simulink library "outp"  (R2021b)
settings: Solver=VariableStepAuto  StartTime=0.0  StopTime=10.0  RelTol=1e-3
undefined symbols (not defined in the file or in its folder): ENUM_PMMMODE_CHARGE, ENUM_PMMMODE_IDLE, ENUM_PMMMODE_INITIALIZE, ENUM_PMMMODE_POWERDOWN, ENUM_PMMMODE_SLEEP, FALSE, Left, outp, slcm, TRUE
libraries: FVT_lib x956, hcu_lib x4, simulink x1
(part 2 of 10)

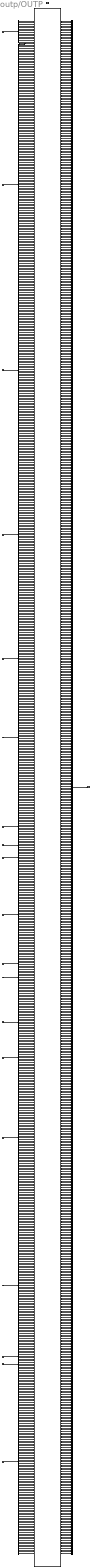
== system outp/OUTP ==
  BACC_outputs : Inport  OutDataTypeStr=Bus: BACC_outputs
  BAPM_outputs : Inport  Port=2  OutDataTypeStr=Bus: BAPM_outputs
  BBCM_outputs : Inport  Port=3  OutDataTypeStr=Bus: BBCM_outputs
  BDDM_outputs : Inport  Port=4  OutDataTypeStr=Bus: BDDM_outputs
  BDHP_outputs : Inport  Port=5  OutDataTypeStr=Bus: BDHP_outputs
  BDID_outputs : Inport  Port=6  OutDataTypeStr=Bus: BDID_outputs
  BDKC_outputs : Inport  Port=7  OutDataTypeStr=Bus: BDKC_outputs
  BDSC_outputs : Inport  Port=8  OutDataTypeStr=Bus: BDSC_outputs
  BNMM_outputs : Inport  Port=9  OutDataTypeStr=Bus: BNMM_outputs
  BPMM_outputs : Inport  Port=10  OutDataTypeStr=Bus: BPMM_outputs
  BPSA_outputs : Inport  Port=11  OutDataTypeStr=Bus: BPSA_outputs
  BSCP_outputs : Inport  Port=12  OutDataTypeStr=Bus: BSCP_outputs
  BSYS_outputs : Inport  Port=13  OutDataTypeStr=Bus: BSYS_outputs
  BTHC_outputs : Inport  Port=14  OutDataTypeStr=Bus: BTHC_outputs
  BTPM_outputs : Inport  Port=15  OutDataTypeStr=Bus: BTPM_outputs
  BTQD_outputs : Inport  Port=16  OutDataTypeStr=Bus: BTQD_outputs
  BTQR_outputs : Inport  Port=17  OutDataTypeStr=Bus: BTQR_outputs
  BV2L_outputs : Inport  Port=18  OutDataTypeStr=Bus: BV2L_outputs
  BVMC_outputs : Inport  Port=19  OutDataTypeStr=Bus: BVMC_outputs
  trig_OUTP : TriggerPort  TriggerType=function-call  VariantControl=(inherit)
  Constant : Constant  Value=FALSE
  bus_creator : BusCreator  Inputs=956  OutDataTypeStr=Bus: BOUTP_outputs  NonVirtualBus=on
  bus_selector1 : BusSelector  OutputSignals=VACC_EACEnDemand_enum,VACC_CACTempOverHigh_flg,VACC_CACPresWarn_flg,VACC_CACPresReady_flg,VACC_EHPSEnDemand_enum,VACC_CACOverrun_flg,VACC_CACRunFail_flg,VACC_EHPSMotorDemSpd_rpm,VACC_EHPSSpdDemTimeout_flg,VACC_EHPSEnTimeout_flg,VACC_EHPSDisEnTimeout_flg,VACC_DCDCEnDemamd_enum,VACC_EHPSSpdCtrlMode_enum,VACC_EACSpdDemand_rpm
  bus_selector10 : BusSelector  OutputSignals=VPMM_SysPowerMode_enum,VPMM_PowerUpState_enum,VPMM_PowerDownState_enum,VPMM_ChrgState_enum,VPMM_PowerUpFault_enum,VPMM_PowerDownFault_enum,VPMM_ChrgFault_enum,VPMM_IRCRlyClose_flg,VPMM_IGNRlyClose_flg,VPMM_BattHVDem_enum,VPMM_DCDCRlyDem_enum,VPMM_CACRlyDem_enum,VPMM_MCUHVLoopDem_enum,VPMM_EHPSRlyDem_enum,VPMM_ACHVLoopDem_enum,VPMM_HVSysReady_enum,VPMM_DrivelineRelease_enum,VPMM_ActiveDischargeReq_enum,VPMM_VCUMCUEn_flg,VPMM_VCUMCUFailRst_flg,VPMM_HVILFail_flg,VPMM_LostHVComActivePwrDown_flg,VPMM_LVBattLowInd_enum,VPMM_ChrgPowerUpFail_flg,VPMM_ChrgBCUHVFail_flg,VPMM_HVFailureChkPass_flg,VPMM_HVILDetectFail_flg,VPMM_V2BLifeSig_cnt,VPMM_V2BAux1OnOff_enum,VPMM_V2BAux2OnOff_enum,VPMM_V2BAux3OnOff_enum,VPMM_V2BMainPosRlySta_enum,VPMM_V2BMainPosRlyFit_enum,VPMM_V2BACPosRlySta_enum,VPMM_V2BACPosRlyFit_enum,VPMM_V2BAirPosRlySta_enum,VPMM_V2BAirPosRlyFit_enum,VPMM_V2BOilPosRlySta_enum,VPMM_V2BOilPosRlyFit_enum,VPMM_V2BDCDCPosRlySta_enum,VPMM_V2BDCDCPosRlyFit_enum,VPMM_V2BAux1RlySta_enum,VPMM_V2BAux1RlyFit_enum,VPMM_V2BAux2RlySta_enum,VPMM_V2BAux2RlyFit_enum,VPMM_V2BAux3RlySta_enum,VPMM_V2BAux3RlyFit_enum,VPMM_V2BAux4RlySta_enum,VPMM_V2BAux4RlyFit_enum,VPMM_VCULife1_cnt,VPMM_VCULife2_cnt,VPMM_VSPFunc_enum,VPMM_VSPIGNKeySta_enum,VPMM_VSPReversed_flg,VPMM_VSPTurnRight_enum,VPMM_VSPTurnLeft_enum,VPMM_FogTMSRlyCMD_enum,VPMM_DCCurr_A,VPMM_DCVol_V
  bus_selector11 : BusSelector  OutputSignals=VPSA_Keystatus_enum,VPSA_EmergencyShutDown_flg
  bus_selector12 : BusSelector  OutputSignals=VSCP_triggerBAM_flg,VSCP_CFGEM1Ctrl_raw,VSCP_CFGEM1BAMTSize_raw,VSCP_CFGEM1BAMTNum_raw,VSCP_CFGEM1BAMRsv_raw,VSCP_CFGEM1BAMPGN_raw,VSCP_triggerDT_flg,VSCP_DTbyte0_raw,VSCP_DTbyte1_raw,VSCP_DTbyte2_raw,VSCP_DTbyte3_raw,VSCP_DTbyte4_raw,VSCP_DTbyte5_raw,VSCP_DTbyte6_raw,VSCP_DTbyte7_raw
  bus_selector13 : BusSelector  OutputSignals=VSYS_HWVer1_cnt,VSYS_HWVer2_cnt,VSYS_HWVer3_cnt,VSYS_CarModel1_cnt,VSYS_CarModel2_cnt,VSYS_CarModel3_cnt,VSYS_ECU1_cnt,VSYS_ECU2_cnt,VSYS_Major1_cnt,VSYS_Major2_cnt,VSYS_Minor1_cnt,VSYS_Minor2_cnt,VSYS_Patch1_cnt,VSYS_Patch2_cnt,VSYS_Country1_cnt,VSYS_Country2_cnt,VSYS_Variation_cnt,VSYS_Dash1_cnt,VSYS_Change1_cnt,VSYS_Change2_cnt,VSYS_Dash2_cnt,VSYS_SHA1_cnt,VSYS_SHA2_cnt,VSYS_SHA3_cnt,VSYS_SHA4_cnt,VSYS_SHA5_cnt,VSYS_SHA6_cnt,VSYS_SHA7_cnt,VSYS_SHA8_cnt,VSYS_NvWriteReqRisingEdge_flg,VSYS_FdcSlpReqRisingEdge_flg,VSYS_FdcSlpTime_sec,VSYS_PmicBootReason_enum,VSYS_WisrBootReason_raw32,VSYS_AcoreRebootCmdACK_flg,VSYS_CurrentNmState_enum,VSYS_ECUGen1_cnt,VSYS_ECUGen2_cnt,VSYS_PmicBootPath_raw32,VSYS_DrivingMode_cnt,VSYS_ModelYear_cnt
  bus_selector14 : BusSelector  OutputSignals=VTHC_EWPPEReq_rpm,VTHC_CoolFanReq_pct,VTHC_AfterrunningMode_flg
  bus_selector15 : BusSelector  OutputSignals=VTPM_LFBatWarn_flg,VTPM_RFBatWarn_flg,VTPM_LRBatWarn_flg,VTPM_RRBatWarn_flg,VTPM_LFWheelPress_raw8,VTPM_RFWheelPress_raw8,VTPM_LRWheelPress_raw8,VTPM_RRWheelPress_raw8,VTPM_LFWheelTemp_C,VTPM_RFWheelTemp_C,VTPM_LRWheelTemp_C,VTPM_RRWheelTemp_C,VTPM_LFSensorFail_flg,VTPM_RFSensorFail_flg,VTPM_LRSensorFail_flg,VTPM_RRSensorFail_flg,VTPM_LFWheelDebug_flg,VTPM_LRWheelDebug_flg,VTPM_RFWheelDebug_flg,VTPM_RRWheelDebug_flg,VTPM_TPMSResButtAllow_flg,VTPM_TPMSCaliButtAllow_flg,VTPM_LFPressIndi_enum,VTPM_RFPressIndi_enum,VTPM_LRPressIndi_enum,VTPM_RRPressIndi_enum,VTPM_TPMSWarnIndi_enum,VTPM_LFWheelTmpIndi_flg,VTPM_RFWheelTmpIndi_flg,VTPM_LRWheelTmpIndi_flg,VTPM_RRWheelTmpIndi_flg,VTPM_LFWheelPSW_raw8,VTPM_LRWheelPSW_raw8,VTPM_RFWheelPSW_raw8,VTPM_RRWheelPSW_raw8,VTPM_CWheelTips_enum,VTPM_AutoLTips_enum,VTPM_LFSensorMode_flg,VTPM_RFSensorMode_flg,VTPM_LRSensorMode_flg,VTPM_RRSensorMode_flg,VTPM_S1ID_raw32,VTPM_S2ID_raw32,VTPM_S3ID_raw32,VTPM_S4ID_raw32,VTPM_S1L_enum,VTPM_S2L_enum,VTPM_S3L_enum,VTPM_S4L_enum,VTPM_ALFin_flg,VTPM_LFP20_raw8,VTPM_RFP20_raw8,VTPM_LRP20_raw8,VTPM_RRP20_raw8,VTPM_FAT_flg,VTPM_IDin_raw32,VTPM_S1WheelDebugALTU_pct,VTPM_S2WheelDebugALTU_pct,VTPM_S3WheelDebugALTU_pct,VTPM_S4WheelDebugALTU_pct,VTPM_ID1messageALTU_raw8,VTPM_ID2messageALTU_raw8,VTPM_ID3messageALTU_raw8,VTPM_ID4messageALTU_raw8,VTPM_Chkfin_flg,VTPM_SetIDLoc_flg,VTPM_TPMSStorge_flg,VTPM_ChkStorge_flg,VTPM_TPMSResButt_flg,VTPM_LFPindi_enum,VTPM_RFPind_enum,VTPM_LRPindi_enum,VTPM_RRPindi_enum,VTPM_WriteChkLFID_raw,VTPM_WriteChkRFID_raw,VTPM_WriteChkLRID_raw,VTPM_WriteChkRRID_raw,VTPM_WriteChkfinLFID_raw,VTPM_WriteChkfinRFID_raw,VTPM_WriteChkfinLRID_raw,VTPM_WriteChkfinRRID_raw,VTPM_Flashchkdatavalid_enum,VTPM_Flashdatavalid_enum,VTPM_unlearnSfali_flg,VTPM_unlearnSfailvalid_enum,VTPM_Prepresstempvalid_enum,VTPM_FlashS1ID_raw,VTPM_FlashS2ID_raw,VTPM_FlashS3ID_raw,VTPM_FlashS4ID_raw,VTPM_FlashIDvalid_enum,VTPM_WritingCnt_enum,VTPM_TPMSTLCmd_flg,VTPM_LProgress_enum,VTPM_TPMSSensorIDRegStart_flg,VTPM_ModelVersion_raw,VTPM_ModelVersionChksum_raw
  bus_selector16 : BusSelector  OutputSignals=VTQD_VCUMCUCtrlMdTQD_enum,VTQD_CreepSpdReq_rpm,VTQD_CreepIND_enum,VTQD_ActTUpAIND_enum,VTQD_VCUMCUDemHiPosVal_rpm,VTQD_VehAcclLimitTG_mps2,VTQD_VCUEBSHHSw_enum,VTQD_VCUEBSRd4BR_enum,VTQD_ParkingProtectWarning_flg,VTQD_ActDriveMode_enum,VTQD_VCU4PweLmtInd_flg,VTQD_GearFlashIndDis_flg,VTQD_GearFlashInd_flg,VTQD_SpdLimSta_flg,VTQD_VehSpdLimitTG_kph,VTQD_VCUTMVehSpd_kph,VTQD_TMTqReq_Nm,VTQD_VCUBCMBuzzReq_flg,VTQD_VCUEBSHBSw_enum,VTQD_EVCU1ActDrvMode_enum,VTQD_EVCU1WheelSlipdet_enum,VTQD_EVCU1EMotorSpd_rpm,VTQD_EVCU1EMotorOvrerSpd_enum,VTQD_EVCU1EMotorPerformance_pct,VTQD_EVCU1EBrakeTorqLow_enum,VTQD_EVCU2MaxTorqAvail_pct,VTQD_EVCU2MinTorqAvail_pct,VTQD_EEC3NFricPercTorq_pct,VTQD_EEC3EMPressLoss_pct,VTQD_ETC2ActDriveDirect_enum,VTQD_RC1PctTrqP4_pct,VTQD_RC1PctTrqPekTrqP5_pct,VTQD_EMRC1EMTquModeDrvBrk_enum,VTQD_EMRC1ActEMpTrq_pct,VTQD_EMRC1ActEMOutSftSpd_rpm,VTQD_EMRC1ActEMpTrqHrls_pct,VTQD_EMRC1ActMaxAvaEMRecpTrq_pct,VTQD_EC1EMSpdIdleP1_rpm,VTQD_EC1PercTorqIdleP1_pct,VTQD_EC1EMSpdIdleP2_rpm,VTQD_EC1PercTorqIdleP2_pct,VTQD_EC1EMSpdIdleP3_rpm,VTQD_EC1PercTorqIdleP3_pct,VTQD_EC1EMSpdIdleP4_rpm,VTQD_EC1PercTorqIdleP4_pct,VTQD_EC1PercTorqIdleP5_pct,VTQD_EC1EMSpdIdleP5_rpm,VTQD_EC1EMRefTorq_Nm,VTQD_EC1EMMaxMEngOvrSP7_rpm,VTQD_EC1EMMaxMOvrTmt_s,VTQD_EC1EMReqSpdCtrlLoLmt_rpm,VTQD_EC1EMReqTrqCtrlLoLmt_pct,VTQD_EC1EMReqSpdCtrlUpLmt_rpm,VTQD_EC1EMReqTrqCtrlUpLmt_pct,VTQD_EC1EMExtRSCtrlUpLmt_rpm,VTQD_EC1EMMomOfInertia_kgpm2,VTQD_EC1EMDefTrqLmt_rpm,VTQD_EC1EMSupVarRTSC1MSG_cnt,VTQD_EC1EMSupTSC1CtrlPG1_cnt,VTQD_EC1EMSupTSC1CtrlPG3_cnt,VTQD_EC1EMSupTSC1CtrlPG2_cnt,VTQD_EC1EMSupTSC1CtrlPG4_cnt,VTQD_EC1EMSpdHdleP6_rpm,VTQD_EC1EMGainEndSpdGvn_gain,VTQD_RC1RetType_enum,VTQD_RC1RetLocat_enum,VTQD_RC1RetCtrlMth_enum,VTQD_RC1RetSpdIdleP1_rpm,VTQD_RC1PctTrqIdleP1_pct,VTQD_RC1MaxRetSpdP2_rpm,VTQD_RC1RetSpdP2_pct,VTQD_RC1MaxRetSpdP3_rpm,VTQD_RC1PctTrqP3_pct,VTQD_RC1RefRetTrq_Nm,VTQD_RC1RetSpdPekTrqP5_Nm,VTQD_RC1RetSpdP4_rpm,VTQD_VCUMCUDemLoNegVal_rpm,VTQD_VCUMCUDemSpd_rpm,VTQD_VCUMCUGearSta_enum,VTQD_TUpAIND_enum,VTQD_ETC1ShiftrPgs_enum,VTQD_EVCU1RecuperHighSta_enum,VTQD_EMRC1DrvDemEMRtapTrq_pct,VTQD_EMRC1RetSelNonEng_pct,VTQD_EMRC1SACtrlDev_cnt,VTQD_VCUMCUHandBrk_flg,VTQD_VCUMCUFootBrk_flg
  bus_selector17 : BusSelector  OutputSignals=VTQR_FrTMTqReq_Nm,VTQR_RrTMTqReq_Nm
  bus_selector18 : BusSelector  OutputSignals=VV2L_ReqOBCV2LEna_enum,VV2L_ReqV2LIVIPopup_enum,VV2L_ReqV2LIVIDisChrg_enum,VV2L_ReqOBCExtrV2LEna_enum,VV2L_ReqOBCIntrV2LEna_enum,VV2L_HVPO120VGrpALDSt_enum,VV2L_HVPO120VGrpBLDSt_enum
  bus_selector19 : BusSelector  OutputSignals=VVMC_FeatSetSpdFinal_raw32,VVMC_VehicleSpeed_mph,VVMC_VehicleSpeed_kph,VVMC_MeterIndSpeed_raw32,VVMC_VMCAEBCtrlAvail_flg,VVMC_VMCACCCtrlAvail_flg,VVMC_VMCCCCtrlAvail_flg,VVMC_VMCMSACtrlAvail_flg,VVMC_FeatArbitrSta_enum,VVMC_FeatReqSpd_kph,VVMC_JerkPCT_pct,VVMC_LimitPCT_pct,VVMC_FrontRearSlipRatioCtrl_flg,VVMC_RearWhlSlipRatioCtrl_flg,VVMC_SingleWhlSlipRatioCtrl_flg,VVMC_LatAccCtrl_flg,VVMC_SafetyCtrl_flg,VVMC_SPD2ACCAct_flg,VVMC_AccCalcuPID_mps2,VVMC_ISOAccLimit_mps2,VVMC_ISODecLimit_mps2,VVMC_ISOJerkLimit_mps3,VVMC_ACCRequiredAccel_mps2,VVMC_DISCReqAcc_mps2,VVMC_FeatArbitrFinal_enum,VVMC_ActACCRequiredAccel_mps2,VVMC_LateralCtrl_flg,VVMC_ADASLKASta_enum,VVMC_LKAStrToqReq_Nm,VVMC_LKATOIFault_flg,VVMC_LKATOIAct_enum,VVMC_ADASAEBReq_enum,VVMC_ADASFaultSta_flg,VVMC_AEBVehHoldReq_flg,VVMC_ACCVehHoldReq_flg,VVMC_ADASDBSReq_enum,VVMC_ADASACCSta_enum,VVMC_ACCObjDist_m,VVMC_ACCObjRelSpd_mps,VVMC_TimeGapLevel_enum,VVMC_ACCJerkUpperLimit_mps3,VVMC_ACCComfortBandUpper_mps2,VVMC_ACCJerkLowerLimit_mps3,VVMC_ACCComfortBandLower_mps2,VVMC_ADASVehSpdLim_raw32,VVMC_ADASShftPosnReqA_flg,VVMC_ADASShftPosnReq_enum,VVMC_ADASForceIdle_flg,VVMC_HazardWarningReq_flg,VVMC_RightTurnLightReq_flg,VVMC_LeftTurnLightReq_flg,VVMC_ADASFCWSta_enum,VVMC_ADASLDWSta_enum,VVMC_ADASFltWrnReq_flg,VVMC_ACCObjDstLvl_enum,VVMC_ForceLowBeam_enum,VVMC_ACCTakeoverReq_flg,VVMC_ADASWarningMsg_enum,VVMC_ADASCAMSpdLim_enum,VVMC_TargetType_enum,VVMC_ADASSLIFSpdLim_enum,VVMC_LKAHODDisplayWarning_flg,VVMC_LKAHODSoundWarning_flg,VVMC_ADASLFCSta_enum,VVMC_ADASLaneModeL_enum,VVMC_ADASLaneModeR_enum,VVMC_ADASSLIFSta_enum,VVMC_ADASISASta_enum,VVMC_ADASLDWMute_flg,VVMC_ADASFCWMute_flg,VVMC_ADASLFCHandsOffWarning_enum,VVMC_LVDADisabled_flg,VVMC_LVDAMuteSta_enum,VVMC_LVDAFailinfo_flg,VVMC_LVDAWarning_flg,VVMC_LVDAACCStatusInformation_flg,VVMC_ADASLFCWarnSound_enum,VVMC_FCMACCmode_enum,VVMC_ADASLanetypeR_enum,VVMC_ADASLanetypeL_enum,VVMC_ADASLanecurveL_raw32,VVMC_ADASLanecurveR_raw32,VVMC_ADASAEBSta_enum,VVMC_FCMLDWRequest_enum,VVMC_FCMLDWFault_flg,VVMC_ACCCtrlAvail_flg,VVMC_ACCPedalOvrd_flg,VVMC_TimeGapCalcu_s,VVMC_CCCtrlSta_enum,VVMC_MSACtrlSta_enum,VVMC_APSCtrlAvail_flg,VVMC_APSActive_flg,VVMC_APSStaSys_enum,VVMC_APSDecReqA_flg,VVMC_APSDecReq_mps2,VVMC_APSReq_enum,VVMC_LongAcc_Gps,VVMC_CCMSASpdWar_flg,VVMC_IMUEnaCmd_flg,VVMC_CAASCtrlAvail_flg,VVMC_CAASActive_flg,VVMC_ExtraMSACtrlSta_enum,VVMC_CalibratedAccX_G,VVMC_CalibratedAccY_G,VVMC_CalibratedAccZ_G,VVMC_CalibratedGyroX_Dps,VVMC_CalibratedGyroY_Dps,VVMC_CalibratedGyroZ_Dps,VVMC_FDCVMCAPSVRqEPSCtrl_flg,VVMC_FDCVMCAPSAngleTarget_deg,VVMC_FDCVMCAPSRqEPSCtrl_flg,VVMC_FDCVMCAngCtrlTqWtGn_pct,VVMC_FDCVMCDrInpTqBstAct_flg,VVMC_FDCVMCMaxAngCtrlOutTqLim_Nm,VVMC_FDCVMCDrInpTqBstGn_pct
  bus_selector2 : BusSelector  OutputSignals=VAPM_VehSpeed_kph,VAPM_VehSpeedTimeOut_flg,VAPM_FSOffSw_enum,VAPM_FSOffSwTimeOut_flg,VAPM_ChrgPlugSta_enum,VAPM_PASDRMR_cm,VAPM_PASDRML_cm,VAPM_PASDRCR_cm,VAPM_PASDRCL_cm,VAPM_PASDFMR_cm,VAPM_PASDFML_cm,VAPM_PASDFCR_cm,VAPM_PASDFCL_cm,VAPM_APSDRLR_cm,VAPM_APSDRLL_cm,VAPM_APSDFLR_cm,VAPM_APSDFLL_cm,VAPM_PASAFCL_enum,VAPM_PASARMR_enum,VAPM_PASARML_enum,VAPM_PASARCR_enum,VAPM_PASARCL_enum,VAPM_PASAFMR_enum,VAPM_PASAFML_enum,VAPM_PASAFCR_enum,VAPM_USSStaRMR_flg,VAPM_USSStaRML_flg,VAPM_USSStaRLR_flg,VAPM_USSStaRLL_flg,VAPM_USSStaRCR_flg,VAPM_USSStaRCL_flg,VAPM_USSStaFMR_flg,VAPM_USSStaFML_flg,VAPM_USSStaFLR_flg,VAPM_USSStaFLL_flg,VAPM_USSStaFCR_flg,VAPM_USSStaFCL_flg,VAPM_Chime_enum,VAPM_SNSRLayout_enum,VAPM_StaFSya_flg,VAPM_ModOperation_enum,VAPM_BrkPedalPos_pct,VAPM_BrkPedalPosTimeOut_flg,VAPM_LFRawWhlSpeed_kph,VAPM_LFRawWhlSpeedTimeOut_flg,VAPM_RFRawWhlSpeed_kph,VAPM_RFRawWhlSpeedTimeOut_flg,VAPM_LRRawWhlSpeed_kph,VAPM_LRRawWhlSpeedTimeOut_flg,VAPM_RRRawWhlSpeed_kph,VAPM_RRRawWhlSpeedTimeOut_flg,VAPM_LFRawWhlSpeedV_flg,VAPM_LFRawWhlSpeedVTimeOut_flg,VAPM_RFRawWhlSpeedV_flg,VAPM_RFRawWhlSpeedVTimeOut_flg,VAPM_LRRawWhlSpeedV_flg,VAPM_LRRawWhlSpeedVTimeOut_flg,VAPM_RRRawWhlSpeedV_flg,VAPM_RRRawWhlSpeedVTimeOut_flg,VAPM_LFWhlRotDir_enum,VAPM_LFWhlRotDirTimeOut_flg,VAPM_RFWhlRotDir_enum,VAPM_RFWhlRotDirTimeOut_flg,VAPM_LRWhlRotDir_enum,VAPM_LRWhlRotDirTimeOut_flg,VAPM_RRWhlRotDir_enum,VAPM_RRWhlRotDirTimeOut_flg,VAPM_LFPulseCountV_flg,VAPM_LFPulseCountVTimeOut_flg,VAPM_RFPulseCountV_flg,VAPM_RFPulseCountVTimeOut_flg,VAPM_LRPulseCountV_flg,VAPM_LRPulseCountVTimeOut_flg,VAPM_RRPulseCountV_flg,VAPM_RRPulseCountVTimeOut_flg,VAPM_LFPulseCount_enum,VAPM_LFPulseCountTimeOut_flg,VAPM_RFPulseCount_enum,VAPM_RFPulseCountTimeOut_flg,VAPM_LRPulseCount_enum,VAPM_LRPulseCountTimeOut_flg,VAPM_RRPulseCount_enum,VAPM_RRPulseCountTimeOut_flg,VAPM_ShifterHandleCmd_enum,VAPM_ShifterHandleCmdTimeOut_flg,VAPM_DriIntend_enum,VAPM_DriIntendTimeOut_flg,VAPM_EPSAOIControl_enum,VAPM_EPSAOIControlTimeOut_flg,VAPM_SASAngle_Deg,VAPM_SASAngleTimeOut_flg,VAPM_SASSpeed_degps,VAPM_SASSpeedTimeOut_flg,VAPM_SASSpeedValid_flg,VAPM_SASSpeedValidTimeOut_flg,VAPM_SASCAL_flg,VAPM_SASCALTimeOut_flg,VAPM_SASV_flg,VAPM_SASVTimeOut_flg,VAPM_GRADE_Deg,VAPM_GRADETimeOut_flg,VAPM_YawRate_degps,VAPM_YawRateTimeOut_flg,VAPM_LatAccel_Gps,VAPM_LatAccelTimeOut_flg,VAPM_LongAccel_Gps,VAPM_LongAccelTimeOut_flg,VAPM_MCPressure_bar,VAPM_MCPressureTimeOut_flg,VAPM_YawRateV_flg,VAPM_YawRateVTimeOut_flg,VAPM_LatAccelV_flg,VAPM_LatAccelVTimeOut_flg,VAPM_LongAccelV_flg,VAPM_LongAccelVTimeOut_flg,VAPM_MCPressureV_bar,VAPM_MCPressureVTimeOut_flg,VAPM_BrkSwSta_flg,VAPM_BrkSwStaTimeOut_flg,VAPM_BrkSwV_flg,VAPM_BrkSwVTimeOut_flg,VAPM_ESCStandstill_flg,VAPM_ESCStandstillTimeOut_flg,VAPM_ESCAPSSta_enum,VAPM_ESCAPSStaTimeOut_flg,VAPM_EPBExtReleaseAvail_flg,VAPM_EPBExtReleaseAvailTimeOut_flg,VAPM_EPBExtApplyAvail_flg,VAPM_EPBExtApplyAvailTimeOut_flg,VAPM_EPBErrSta_enum,VAPM_EPBErrStaTimeOut_flg,VAPM_EPBSta_enum,VAPM_EPBStaTimeOut_flg,VAPM_AVMparkingcancel_enum,VAPM_AVMparkingcancelTimeOut_flg,VAPM_AVMparkingexcute_enum,VAPM_AVMparkingexcuteTimeOut_flg,VAPM_AVMParkingmode_enum,VAPM_AVMParkingmodeTimeOut_flg,VAPM_AVMErrSTA_flg,VAPM_AVMErrSTATimeOut_flg,VAPM_IVIStatus_flg,VAPM_IVIStatusTimeOut_flg,VAPM_CAASSw_enum,VAPM_CAASSwTimeOut_flg,VAPM_IVIScreen_enum,VAPM_IVIScreenTimeOut_flg,VAPM_ABSActive_flg,VAPM_ABSActiveTimeOut_flg,VAPM_TCSActive_flg,VAPM_TCSActiveTimeOut_flg,VAPM_DriverSeatBeltCmd_flg,VAPM_DriverSeatBeltCmdTimeOut_flg,VAPM_APSProgressPCT_pct,VAPM_APSRQDisplay_enum,VAPM_APSSWVer_enum,VAPM_APSHWVer_enum,VAPM_APSExitCondition_enum,VAPM_APSAngleTarget_Deg,VAPM_APSVRqEPASCtrl_flg,VAPM_APSRqEPASCtrl_flg,VAPM_CAASSta_enum,VAPM_DKCPDkeyAreaRAPSSta_enum,VAPM_DKCParkingModeCmd_enum,VAPM_PUIDLowPower_flg,VAPM_CAASVMCReqA_flg,VAPM_APSShiftPosnReq_enum,VAPM_APSSpeedCMD_kph,VAPM_APSVMCReqA_flg,VAPM_RAPSBCMLamp_enum,VAPM_RAPSBCMLockReq_flg,VAPM_APSPwrReq_enum,VAPM_RAPSErrWarnSta_enum,VAPM_RAPSErrLv1_flg,VAPM_IVIUserTakeOverAPSSta_flg
  bus_selector3 : BusSelector  OutputSignals=VBCM_FDCBCMLBeamCmd_flg,VBCM_FDCBCMPLampCmd_flg,VBCM_FDCBCMHBeamCmd_flg,VBCM_FDCBCMSMKLCmd_flg,VBCM_FDCBCMSMKRCmd_flg,VBCM_FDCBCMDVRSignalLCmd_flg,VBCM_FDCBCMDVRSignalRCmd_flg,VBCM_FDCBCMBSDBuzzerCmd_flg,VBCM_FDCBCMSLTLpCmd_flg,VBCM_FDCBCMSRTLpCmd_flg,VBCM_FDCBCMLTurnLpCmd_flg,VBCM_FDCBCMRTurnLpCmd_flg,VBCM_FDCBCMStopINDCmd_flg,VBCM_FDCBCMSTOPBALLCmd_flg,VBCM_FDCBCMInnerCallBellCmd_flg,VBCM_FDCBCMCallBellCmd_flg,VBCM_FDCBCMWiperHCmd_flg,VBCM_FDCBCMWasherCmd_flg,VBCM_FDCBCMWiperLCmd_flg,VBCM_FDCBCMLDRLCmd_flg,VBCM_FDCBCMRDRLCmd_flg,VBCM_FDCBCMRFLampCmd_flg,VBCM_TurnLpPatternSta_enum,VBCM_FDCBCMFDoorSta_flg,VBCM_FDCBCMMDoorSta_flg,VBCM_FDCBCMRDoorSta_flg,VBCM_FDCBCMRoomLpAmbCmd_flg,VBCM_FDCBCMLBSDRCmd_flg,VBCM_FDCBCMLBSDYCmd_flg,VBCM_FDCBCMRBSDRCmd_flg,VBCM_FDCBCMRBSDYCmd_flg,VBCM_FDCBCMEmExitSWSta_flg,VBCM_InnerBuzzerModeSta_enum,VBCM_FDCBCMInnerBuzzerCmd_flg,VBCM_FDCBCMRoomLpAmbSetSta_flg,VBCM_FDCBCMRoomLpSetSta_flg,VBCM_FDCBCMFRoomLpSetSta_pct,VBCM_FDCBCMFRoomLpCmd_pct,VBCM_FDCBCMMRoomLpSetSta_pct,VBCM_FDCBCMMRoomLpCmd_pct,VBCM_FDCBCMRRoomLpSetSta_pct,VBCM_FDCBCMRRoomLpCmd_pct,VBCM_FDCBCMHelpINDCmd_flg,VBCM_FDCBCMOSDrOpenSWSta_enum,VBCM_FDCBCMEmSVCmd_flg,VBCM_FDCBCMFDOpenSVCmd_flg,VBCM_FDCBCMFDCloseSVCmd_flg,VBCM_FDCBCMMDOpenSVCmd_flg,VBCM_FDCBCMMDCloseSVCmd_flg,VBCM_FDCBCMLTurnSWSta_flg,VBCM_FDCBCMRTurnSWSta_flg,VBCM_FDCBCMRGearSta_flg,VBCM_FDCBCMBrakeCmd_flg,VBCM_FDCBCMTurnBuzzerENSta_flg,VBCM_WakeUp_flg,VBCM_KeepWakeUp_flg
  bus_selector4 : BusSelector  OutputSignals=VDDM_C3BMS6RCDTC_raw32,VDDM_C3BMS6CSDTC_raw32,VDDM_C3BMS6LCDTC_raw32,VDDM_C3BMS1RCDTC_raw32,VDDM_C3BMS1CSDTC_raw32,VDDM_C3BMS1LCDTC_raw32,VDDM_C3CCU1RCDTC_raw32,VDDM_C3CCU1CSDTC_raw32,VDDM_C3CCU1LCDTC_raw32,VDDM_C3CCU2RCDTC_raw32,VDDM_C3CCU2CSDTC_raw32,VDDM_C3CCU2LCDTC_raw32,VDDM_C1ABM1RCDTC_raw32,VDDM_C1ABM1CSDTC_raw32,VDDM_C1ABM1LCDTC_raw32,VDDM_Lv1ErrDTC_raw32,VDDM_Lv2ErrDTC_raw32,VDDM_Lv3ErrDTC_raw32,VDDM_Lv4ErrDTC_raw32,VDDM_BrkSWErrDTC_raw32,VDDM_BrkSWNoBacDTC_raw32,VDDM_KeyAuthDTC_raw32,VDDM_ONtoRdyDTC_raw32,VDDM_HVB4PreDTC_raw32,VDDM_MCU4PreDTC_raw32,VDDM_DCDC4PreDTC_raw32,VDDM_HVRlyCloDTC_raw32,VDDM_BMSRdyDTC_raw32,VDDM_DCDCEnaDTC_raw32,VDDM_HiLvSaChkDTC_raw32,VDDM_MidLvSaChkDTC_raw32,VDDM_MCUDisDTC_raw32,VDDM_DCDCDisDTC_raw32,VDDM_HVRlyOpDTC_raw32,VDDM_MCUActDTC_raw32,VDDM_OBC4PreDTC_raw32,VDDM_IniLVLoDTC_raw32,VDDM_LVSupLoDTC_raw32,VDDM_LVSupHiDTC_raw32,VDDM_DrStSWDTC_raw32,VDDM_FLDoorSWDTC_raw32,VDDM_RLDoorSWDTC_raw32,VDDM_FRDoorSWDTC_raw32,VDDM_RRDoorSWDTC_raw32,VDDM_HoodSWDTC_raw32,VDDM_TailgaSWDTC_raw32,VDDM_EDriveSysErrVCUErr_flg,VDDM_VehMalfunLevel_enum,VDDM_APS1SigOoRDTC_raw32,VDDM_APS2SigOoRDTC_raw32,VDDM_APSCorrErrDTC_raw32,VDDM_MCUF1NoComDTC_raw32,VDDM_MCUR1NoComDTC_raw32,VDDM_Shifter1NoComDTC_raw32,VDDM_ESC7NoComDTC_raw32,VDDM_ESC1NoComDTC_raw32,VDDM_ESC5NoComDTC_raw32,VDDM_EnterNewOperCyc_flg,VDDM_DiagHCrashDTC_raw32,VDDM_DiagFLTSDTC_raw32,VDDM_DiagFRTSDTC_raw32,VDDM_DiagRLTSDTC_raw32,VDDM_DiagRRTSDTC_raw32,VDDM_FCLUSSDTC_raw32,VDDM_FMLUSSDTC_raw32,VDDM_FMRUSSDTC_raw32,VDDM_FCRUSSDTC_raw32,VDDM_RCLUSSDTC_raw32,VDDM_RMLUSSDTC_raw32,VDDM_RMRUSSDTC_raw32,VDDM_RCRUSSDTC_raw32,VDDM_FLLUSSDTC_raw32,VDDM_FLRUSSDTC_raw32,VDDM_RLLUSSDTC_raw32,VDDM_RLRUSSDTC_raw32,VDDM_FCM2NoComDTC_raw32,VDDM_FCM2RCErrDTC_raw32,VDDM_FCM2CSErrDTC_raw32,VDDM_FCM3NoComDTC_raw32,VDDM_FCM3RCErrDTC_raw32,VDDM_FCM3CSErrDTC_raw32,VDDM_FCM4NoComDTC_raw32,VDDM_FCM4CSErrDTC_raw32,VDDM_FCM5NoComDTC_raw32,VDDM_FCM5CSErrDTC_raw32,VDDM_ZoneSCPNoComDTC_raw32,VDDM_BMSSigErrDetDTC_raw32,VDDM_FCMACCSigErrDetDTC_raw32,VDDM_FrMCUSigErrDetDTC_raw32,VDDM_RrMCUSigErrDetDTC_raw32,VDDM_CCUSigErrDetDTC_raw32,VDDM_ACCAccelCmdErrDetDTC_raw32,VDDM_ACCMalfuncDetDTC_raw32,VDDM_CCMalfuncDetDTC_raw32,VDDM_MSAMalfuncDetDTC_raw32,VDDM_ISAMalfuncDetDTC_raw32,VDDM_MCUF1RCErrDTC_raw32,VDDM_MCUR1RCErrDTC_raw32,VDDM_MCUF1CSErrDTC_raw32,VDDM_MCUR1CSErrDTC_raw32,VDDM_Shifter1RCErrDTC_raw32,VDDM_Shifter1CSErrDTC_raw32,VDDM_ESC7RCErrDTC_raw32,VDDM_ESC7CSErrDTC_raw32,VDDM_ESC1RCErrDTC_raw32,VDDM_ESC1CSErrDTC_raw32,VDDM_ESC5RCErrDTC_raw32,VDDM_ESC5CSErrDTC_raw32,VDDM_FrMCUTqErrDTC_raw32,VDDM_RrMCUTqErrDTC_raw32,VDDM_LFBatwarnDTC_raw32,VDDM_RFBatwarnDTC_raw32,VDDM_LRBatwarnDTC_raw32,VDDM_RRBatwarnDTC_raw32,VDDM_LFPressIndiDTC_raw32,VDDM_RFPressIndiDTC_raw32,VDDM_LRPressIndiDTC_raw32,VDDM_RRPressIndiDTC_raw32,VDDM_LFWheelTmpHighDTC_raw32,VDDM_RFWheelTmpHighDTC_raw32,VDDM_LRWheelTmpHighDTC_raw32,VDDM_RRWheelTmpHighDTC_raw32,VDDM_LFSensorFailDTC_raw32,VDDM_RFSensorFailDTC_raw32,VDDM_LRSensorFailDTC_raw32,VDDM_RRSensorFailDTC_raw32,VDDM_C1EPAS2LCDTC_raw32,VDDM_5vAPS1PwrErrDTC_raw32,VDDM_5vAPS2PwrErrDTC_raw32,VDDM_EPBLockTODTC_raw32,VDDM_EPBUnlockTODTC_raw32,VDDM_LimpHomeActTmp_flg,VDDM_DTCDetect_enum,VDDM_EngagePFail_flg,VDDM_DisengagePFail_flg,VDDM_VCURAPSErrLv2_flg,VDDM_VCURAPSErrLv3_flg,VDDM_EDriveSysErrShifterErr_flg,VDDM_LVSysErrPwrOutErr_flg,VDDM_HVRlyOpFail_flg,VDDM_MCUActDisFail_flg,VDDM_VCUBrkSWSta_enum,VDDM_VCUFLDoorSta_flg,VDDM_VCUFRDoorSta_flg,VDDM_VCURLDoorSta_flg,VDDM_VCURRDoorSta_flg,VDDM_SysAllowReadySta_flg,VDDM_VCUHoodSWSta_flg,VDDM_VCUTailgateSWSta_flg
  bus_selector5 : BusSelector  OutputSignals=VDHP_ActAPSPosn_pct,VDHP_EAPS1MIN_pct,VDHP_EAPS2MIN_pct,VDHP_ResetPedalZeroPosStart_flg,VDHP_EAPS1NRM_pct,VDHP_EAPS2NRM_pct
  bus_selector6 : BusSelector  OutputSignals=VDID_VSS_kph,VDID_RUNTM_s,VDID_MILDIST_km,VDID_WARMUPS_cnt,VDID_CLRDIST_km,VDID_APPD_pct,VDID_APPE_pct,VDID_MILTIME_min,VDID_CLRTIME_min,VDID_BATSOC_pct,VDID_HEVBATT_V,VDID_ODOMETER_km,VDID_BATSOH_pct,VDID_HVBCellVoltMin_V,VDID_HVBCellVoltMax_V,VDID_HVESSCHARGELIM_kW,VDID_HVESSCHARGEACT_kW,VDID_HVESSENER_Whps,VDID_NUMPSATRIPSFLTMEMCLR_cnt,VDID_HVBattCurr_Ahps,VDID_PSAR_sec,VDID_PSAL_sec,VDID_IPSAR_sec,VDID_IPSAL_sec,VDID_CPSAR_sec,VDID_CPSAL_sec,VDID_HVBNAH_Ahr,VDID_HVBNE_kWh,VDID_IGNCNTR_cnt,VDID_TNBCPSAR_Ahr,VDID_TNBCPSAL_Ahr,VDID_TNECPSAR_kWh,VDID_TNECPSAL_kWh,VDID_TEBPSAR_kWh,VDID_TEBPSAL_kWh,VDID_TGEOVCR_kWh,VDID_TGEOVCL_kWh,VDID_GECHGOVCDCR_kWh,VDID_GECHGOVCDCL_kWh,VDID_GECHGOVCACR_kWh,VDID_GECHGOVCACL_kWh,VDID_RESSV2XENNONPSAR_kWh,VDID_RESSV2XENNONPSAL_kWh,VDID_PKER_kphsqr,VDID_PKEL_kphsqr,VDID_ResetCDEODTR_km,VDID_CDEODTR_km,VDID_CDEODTL_km,VDID_AvgBattTempPSAR_C,VDID_AvgBattTempPSAL_C,VDID_AvgBattTempOVCR_C,VDID_AvgBattTempOVCL_C,VDID_AvgBattTempOFFR_C,VDID_AvgBattTempOFFL_C,VDID_QTYPSATRIPSR_cnt,VDID_QTYPSATRIPSL_cnt,VDID_RESSCNTDODRNGR_cnt,VDID_RESSCNTDODRNGL_cnt,VDID_ETMATOER_kWh,VDID_ETMATOEL_kWh,VDID_ETMBTOER_kWh,VDID_ETMBTOEL_kWh,VDID_RESSTIMESOCPSARNGR_s,VDID_RESSTIMESOCPSARNGL_s,VDID_RESSTIMESOCCHGRNGR_s,VDID_RESSTIMESOCCHGRNGL_s,VDID_RESSTIMESOCOFFRNGR_s,VDID_RESSTIMESOCOFFRNGL_s,VDID_MAXBATTEMPL_C,VDID_MINBATTEMPL_C,VDID_AVGBATTEMPL_C,VDID_PROTOCOLID_enum,VDID_RESSTTEMPRNGAXIS_enum,VDID_RESSTIMESOCRNGAXIS_enum,VDID_RESSCNTSDODRNGAXIS_enum,VDID_CALID_cnt,VDID_ECUNAME_cnt,VDID_PKERNumerator_kphsqr,VDID_PKELNumerator_kphsqr,VDID_BattTempPSAR_sec,VDID_BattTempPSAL_sec,VDID_OVCR_sec,VDID_OVCL_sec,VDID_OFFR_sec,VDID_OFFL_sec,VDID_AVGBATTEMPL_sec,VDID_VinCode_cnt,VDID_STASUP_enum,VDID_HEVMODE_enum,VDID_HVBATT_A,VDID_DIDModelVersion_raw,VDID_DIDModelVersionChksum_raw
  bus_selector7 : BusSelector  OutputSignals=VDKC_DKCTimeSN_cnt,VDKC_DKCAuthSta_enum,VDKC_TimeSNDKCFbk_cnt,VDKC_KeyMissSta_flg,VDKC_KeyModeSta_enum,VDKC_DkeyShowIVISta_enum,VDKC_KeyAreaPS_enum,VDKC_KeyAreaLockUnlock_enum,VDKC_PCommandToBCM_enum,VDKC_DKeyWelcomeSta_enum,VDKC_KeyAreaPTG_enum,VDKC_KeyAreaSPTGSta_enum,VDKC_UIDLowPowerSta_enum,VDKC_DkeyAreaRAPSSta_enum,VDKC_ParkingModeCmd_enum,VDKC_KeyNumSta_enum,VDKC_KeyTypeSta_enum,VDKC_FDCDKCAllowSleep_flg,VDKC_JudgeKeepUnlockZone_flg
  bus_selector8 : BusSelector  OutputSignals=VDSC_DISCTurn_flg,VDSC_DISCTargetSpd_kph,VDSC_DISCSta_enum,VDSC_DISCButtSta_flg
  bus_selector9 : BusSelector  OutputSignals=VNMM_AllCANTxReq_flg,VNMM_NMmTxReq_flg,VNMM_Awake_enum,VNMM_CSB_flg,VNMM_ErrorState_enum,VNMM_NodeID_enum,VNMM_PNI_flg,VNMM_RptMsgReq_flg,VNMM_WakeUp_enum,VNMM_ActiveWU_flg,VNMM_SysNMmSta_enum,VNMM_NetworkReq_flg
  outpmodule : Subsystem
  BOUTP_outputs : Outport  OutDataTypeStr=Bus: BOUTP_outputs
  wires:
  outpmodule/952(VOUTP_FDCVMCAPSRqEPSCtrl_flg) -> bus_creator/952
  outpmodule/950(VOUTP_FDCVMCAPSVRqEPSCtrl_flg) -> bus_creator/950
  outpmodule/948(VOUTP_CalibratedGyroY_Dps) -> bus_creator/948
  outpmodule/947(VOUTP_CalibratedGyroX_Dps) -> bus_creator/947
  outpmodule/942(VOUTP_CAASActive_flg) -> bus_creator/942
  outpmodule/940(VOUTP_IMUEnaCmd_flg) -> bus_creator/940
  outpmodule/938(VOUTP_LongAcc_Gps) -> bus_creator/938
  outpmodule/936(VOUTP_APSDecReq_mps2) -> bus_creator/936
  outpmodule/933(VOUTP_APSActive_flg) -> bus_creator/933
  outpmodule/928(VOUTP_ACCPedalOvrd_flg) -> bus_creator/928
  outpmodule/929(VOUTP_TimeGapCalcu_s) -> bus_creator/929
  outpmodule/925(VOUTP_FCMLDWRequest_enum) -> bus_creator/925
  outpmodule/923(VOUTP_ADASLanecurveR_raw32) -> bus_creator/923
  outpmodule/918(VOUTP_ADASLFCWarnSound_enum) -> bus_creator/918
  outpmodule/914(VOUTP_LVDAMuteSta_enum) -> bus_creator/914
  outpmodule/913(VOUTP_LVDADisabled_flg) -> bus_creator/913
  outpmodule/911(VOUTP_ADASFCWMute_flg) -> bus_creator/911
  outpmodule/910(VOUTP_ADASLDWMute_flg) -> bus_creator/910
  outpmodule/907(VOUTP_ADASLaneModeR_enum) -> bus_creator/907
  outpmodule/908(VOUTP_ADASSLIFSta_enum) -> bus_creator/908
  outpmodule/902(VOUTP_ADASSLIFSpdLim_enum) -> bus_creator/902
  outpmodule/904(VOUTP_LKAHODSoundWarning_flg) -> bus_creator/904
  outpmodule/903(VOUTP_LKAHODDisplayWarning_flg) -> bus_creator/903
  outpmodule/900(VOUTP_ADASCAMSpdLim_enum) -> bus_creator/900
  outpmodule/901(VOUTP_TargetType_enum) -> bus_creator/901
  outpmodule/898(VOUTP_ACCTakeoverReq_flg) -> bus_creator/898
  outpmodule/895(VOUTP_ADASFltWrnReq_flg) -> bus_creator/895
  outpmodule/892(VOUTP_LeftTurnLightReq_flg) -> bus_creator/892
  outpmodule/893(VOUTP_ADASFCWSta_enum) -> bus_creator/893
  outpmodule/890(VOUTP_HazardWarningReq_flg) -> bus_creator/890
  outpmodule/889(VOUTP_ADASForceIdle_flg) -> bus_creator/889
  outpmodule/886(VOUTP_ADASVehSpdLim_raw32) -> bus_creator/886
  outpmodule/883(VOUTP_ACCComfortBandUpper_mps2) -> bus_creator/883
  bus_creator/1 -> BOUTP_outputs/1
  outpmodule/956(VOUTP_FDCVMCDrInpTqBstGn_pct) -> bus_creator/956
  outpmodule/835(VOUTP_ReqOBCV2LEna_enum) -> bus_creator/835
  outpmodule/830(VOUTP_EMRC1SACtrlDev_cnt) -> bus_creator/830
  outpmodule/822(VOUTP_VCUMCUDemLoNegVal_rpm) -> bus_creator/822
  outpmodule/821(VOUTP_RC1RetSpdP4_rpm) -> bus_creator/821
  outpmodule/823(VOUTP_VCUMCUDemSpd_rpm) -> bus_creator/823
  outpmodule/820(VOUTP_RC1RetSpdPekTrqP5_Nm) -> bus_creator/820
  outpmodule/819(VOUTP_RC1RefRetTrq_Nm) -> bus_creator/819
  outpmodule/816(VOUTP_RC1RetSpdP2_pct) -> bus_creator/816
  outpmodule/814(VOUTP_RC1PctTrqIdleP1_pct) -> bus_creator/814
  outpmodule/811(VOUTP_RC1RetLocat_enum) -> bus_creator/811
  outpmodule/808(VOUTP_EC1EMSpdHdleP6_rpm) -> bus_creator/808
  outpmodule/806(VOUTP_EC1EMSupTSC1CtrlPG2_cnt) -> bus_creator/806
  outpmodule/804(VOUTP_EC1EMSupTSC1CtrlPG1_cnt) -> bus_creator/804
  outpmodule/803(VOUTP_EC1EMSupVarRTSC1MSG_cnt) -> bus_creator/803
  outpmodule/799(VOUTP_EC1EMReqTrqCtrlUpLmt_pct) -> bus_creator/799
  outpmodule/794(VOUTP_EC1EMMaxMEngOvrSP7_rpm) -> bus_creator/794
  outpmodule/795(VOUTP_EC1EMMaxMOvrTmt_s) -> bus_creator/795
  outpmodule/789(VOUTP_EC1EMSpdIdleP4_rpm) -> bus_creator/789
  outpmodule/790(VOUTP_EC1PercTorqIdleP4_pct) -> bus_creator/790
  outpmodule/780(VOUTP_EMRC1ActEMOutSftSpd_rpm) -> bus_creator/780
  outpmodule/781(VOUTP_EMRC1ActEMpTrqHrls_pct) -> bus_creator/781
  outpmodule/775(VOUTP_ETC2ActDriveDirect_enum) -> bus_creator/775
  outpmodule/772(VOUTP_EVCU2MinTorqAvail_pct) -> bus_creator/772
  outpmodule/769(VOUTP_EVCU1EMotorPerformance_pct) -> bus_creator/769
  outpmodule/765(VOUTP_EVCU1ActDrvMode_enum) -> bus_creator/765
  outpmodule/843(VOUTP_VehicleSpeed_mph) -> bus_creator/843
  outpmodule/840(VOUTP_HVPO120VGrpALDSt_enum) -> bus_creator/840
  outpmodule/842(VOUTP_FeatSetSpdFinal_raw32) -> bus_creator/842
  outpmodule/838(VOUTP_ReqOBCExtrV2LEna_enum) -> bus_creator/838
  outpmodule/837(VOUTP_ReqV2LIVIDisChrg_enum) -> bus_creator/837
  outpmodule/757(VOUTP_GearFlashIndDis_flg) -> bus_creator/757
  outpmodule/756(VOUTP_VCU4PweLmtInd_flg) -> bus_creator/756
  outpmodule/754(VOUTP_ParkingProtectWarning_flg) -> bus_creator/754
  outpmodule/749(VOUTP_ActTUpAIND_enum) -> bus_creator/749
  outpmodule/747(VOUTP_CreepSpdReq_rpm) -> bus_creator/747
  outpmodule/745(VOUTP_ModelVersionChksum_raw) -> bus_creator/745
  outpmodule/744(VOUTP_ModelVersion_raw) -> bus_creator/744
  outpmodule/741(VOUTP_TPMSTLCmd_flg) -> bus_creator/741
  outpmodule/739(VOUTP_FlashIDvalid_enum) -> bus_creator/739
  outpmodule/736(VOUTP_FlashS2ID_raw) -> bus_creator/736
  outpmodule/734(VOUTP_Prepresstempvalid_enum) -> bus_creator/734
  outpmodule/733(VOUTP_unlearnSfailvalid_enum) -> bus_creator/733
  outpmodule/731(VOUTP_Flashdatavalid_enum) -> bus_creator/731
  outpmodule/727(VOUTP_WriteChkfinRFID_raw) -> bus_creator/727
  outpmodule/728(VOUTP_WriteChkfinLRID_raw) -> bus_creator/728
  outpmodule/726(VOUTP_WriteChkfinLFID_raw) -> bus_creator/726
  outpmodule/724(VOUTP_WriteChkLRID_raw) -> bus_creator/724
  outpmodule/922(VOUTP_ADASLanecurveL_raw32) -> bus_creator/922
  outpmodule/722(VOUTP_WriteChkLFID_raw) -> bus_creator/722
  outpmodule/721(VOUTP_RRPindi_enum) -> bus_creator/721
  outpmodule/720(VOUTP_LRPindi_enum) -> bus_creator/720
  outpmodule/716(VOUTP_ChkStorge_flg) -> bus_creator/716
  outpmodule/713(VOUTP_Chkfin_flg) -> bus_creator/713
  outpmodule/714(VOUTP_SetIDLoc_flg) -> bus_creator/714
  outpmodule/712(VOUTP_ID4messageALTU_raw8) -> bus_creator/712
  outpmodule/709(VOUTP_ID1messageALTU_raw8) -> bus_creator/709
  outpmodule/708(VOUTP_S4WheelDebugALTU_pct) -> bus_creator/708
  outpmodule/706(VOUTP_S2WheelDebugALTU_pct) -> bus_creator/706
  outpmodule/707(VOUTP_S3WheelDebugALTU_pct) -> bus_creator/707
  outpmodule/703(VOUTP_FAT_flg) -> bus_creator/703
  outpmodule/695(VOUTP_S2L_enum) -> bus_creator/695
  outpmodule/693(VOUTP_S4ID_raw32) -> bus_creator/693
  outpmodule/694(VOUTP_S1L_enum) -> bus_creator/694
  outpmodule/691(VOUTP_S2ID_raw32) -> bus_creator/691
  outpmodule/687(VOUTP_RFSensorMode_flg) -> bus_creator/687
  outpmodule/685(VOUTP_AutoLTips_enum) -> bus_creator/685
  outpmodule/682(VOUTP_RFWheelPSW_raw8) -> bus_creator/682
  outpmodule/759(VOUTP_SpdLimSta_flg) -> bus_creator/759
  outpmodule/760(VOUTP_VehSpdLimitTG_kph) -> bus_creator/760
  outpmodule/761(VOUTP_VCUTMVehSpd_kph) -> bus_creator/761
  outpmodule/679(VOUTP_RRWheelTmpIndi_flg) -> bus_creator/679
  outpmodule/681(VOUTP_LRWheelPSW_raw8) -> bus_creator/681
  outpmodule/680(VOUTP_LFWheelPSW_raw8) -> bus_creator/680
  outpmodule/671(VOUTP_LFPressIndi_enum) -> bus_creator/671
  outpmodule/954(VOUTP_FDCVMCDrInpTqBstAct_flg) -> bus_creator/954
  outpmodule/669(VOUTP_TPMSResButtAllow_flg) -> bus_creator/669
  outpmodule/665(VOUTP_LFWheelDebug_flg) -> bus_creator/665
  outpmodule/666(VOUTP_LRWheelDebug_flg) -> bus_creator/666
  outpmodule/662(VOUTP_RFSensorFail_flg) -> bus_creator/662
  outpmodule/661(VOUTP_LFSensorFail_flg) -> bus_creator/661
  outpmodule/652(VOUTP_RRBatWarn_flg) -> bus_creator/652
  outpmodule/650(VOUTP_RFBatWarn_flg) -> bus_creator/650
  outpmodule/649(VOUTP_LFBatWarn_flg) -> bus_creator/649
  outpmodule/644(VOUTP_DrivingMode_cnt) -> bus_creator/644
  outpmodule/639(VOUTP_AcoreRebootCmdACK_flg) -> bus_creator/639
  outpmodule/641(VOUTP_ECUGen1_cnt) -> bus_creator/641
  outpmodule/640(VOUTP_CurrentNmState_enum) -> bus_creator/640
  outpmodule/637(VOUTP_PmicBootReason_enum) -> bus_creator/637
  outpmodule/636(VOUTP_FdcSlpTime_sec) -> bus_creator/636
  outpmodule/633(VOUTP_SHA8_cnt) -> bus_creator/633
  outpmodule/630(VOUTP_SHA5_cnt) -> bus_creator/630
  outpmodule/629(VOUTP_SHA4_cnt) -> bus_creator/629
  outpmodule/628(VOUTP_SHA3_cnt) -> bus_creator/628
  outpmodule/625(VOUTP_Dash2_cnt) -> bus_creator/625
  outpmodule/624(VOUTP_Change2_cnt) -> bus_creator/624
  outpmodule/618(VOUTP_Patch2_cnt) -> bus_creator/618
  outpmodule/619(VOUTP_Country1_cnt) -> bus_creator/619
  outpmodule/617(VOUTP_Patch1_cnt) -> bus_creator/617
  outpmodule/616(VOUTP_Minor2_cnt) -> bus_creator/616
  outpmodule/608(VOUTP_CarModel1_cnt) -> bus_creator/608
  outpmodule/606(VOUTP_HWVer2_cnt) -> bus_creator/606
  outpmodule/604(VOUTP_DTbyte7_raw) -> bus_creator/604
  outpmodule/603(VOUTP_DTbyte6_raw) -> bus_creator/603
  outpmodule/602(VOUTP_DTbyte5_raw) -> bus_creator/602
  outpmodule/597(VOUTP_DTbyte0_raw) -> bus_creator/597
  outpmodule/596(VOUTP_triggerDT_flg) -> bus_creator/596
  outpmodule/595(VOUTP_CFGEM1BAMPGN_raw) -> bus_creator/595
  outpmodule/590(VOUTP_triggerBAM_flg) -> bus_creator/590
  outpmodule/924(VOUTP_ADASAEBSta_enum) -> bus_creator/924
  outpmodule/591(VOUTP_CFGEM1Ctrl_raw) -> bus_creator/591
  outpmodule/589(VOUTP_EmergencyShutDown_flg) -> bus_creator/589
  outpmodule/588(VOUTP_Keystatus_enum) -> bus_creator/588
  outpmodule/586(VOUTP_DCCurr_A) -> bus_creator/586
  outpmodule/585(VOUTP_FogTMSRlyCMD_enum) -> bus_creator/585
  outpmodule/581(VOUTP_VSPIGNKeySta_enum) -> bus_creator/581
  outpmodule/899(VOUTP_ADASWarningMsg_enum) -> bus_creator/899
  outpmodule/578(VOUTP_VCULife1_cnt) -> bus_creator/578
  outpmodule/573(VOUTP_V2BAux2RlyFit_enum) -> bus_creator/573
  outpmodule/571(VOUTP_V2BAux1RlyFit_enum) -> bus_creator/571
  outpmodule/570(VOUTP_V2BAux1RlySta_enum) -> bus_creator/570
  outpmodule/563(VOUTP_V2BACPosRlyFit_enum) -> bus_creator/563
  outpmodule/927(VOUTP_ACCCtrlAvail_flg) -> bus_creator/927
  outpmodule/564(VOUTP_V2BAirPosRlySta_enum) -> bus_creator/564
  outpmodule/560(VOUTP_V2BMainPosRlySta_enum) -> bus_creator/560
  outpmodule/561(VOUTP_V2BMainPosRlyFit_enum) -> bus_creator/561
  outpmodule/551(VOUTP_LVBattLowInd_enum) -> bus_creator/551
  outpmodule/543(VOUTP_ACHVLoopDem_enum) -> bus_creator/543
  outpmodule/541(VOUTP_MCUHVLoopDem_enum) -> bus_creator/541
  outpmodule/538(VOUTP_BattHVDem_enum) -> bus_creator/538
  outpmodule/540(VOUTP_CACRlyDem_enum) -> bus_creator/540
  outpmodule/536(VOUTP_IRCRlyClose_flg) -> bus_creator/536
  outpmodule/531(VOUTP_PowerDownState_enum) -> bus_creator/531
  outpmodule/526(VOUTP_ActiveWU_flg) -> bus_creator/526
  outpmodule/524(VOUTP_RptMsgReq_flg) -> bus_creator/524
  outpmodule/522(VOUTP_NodeID_enum) -> bus_creator/522
  outpmodule/474(VOUTP_RESSTTEMPRNGAXIS_enum) -> bus_creator/474
  outpmodule/471(VOUTP_MINBATTEMPL_C) -> bus_creator/471
  outpmodule/468(VOUTP_RESSTIMESOCOFFRNGR_s) -> bus_creator/468
  outpmodule/465(VOUTP_RESSTIMESOCPSARNGL_s) -> bus_creator/465
  outpmodule/461(VOUTP_ETMATOEL_kWh) -> bus_creator/461
  outpmodule/462(VOUTP_ETMBTOER_kWh) -> bus_creator/462
  outpmodule/792(VOUTP_EC1EMSpdIdleP5_rpm) -> bus_creator/792
  outpmodule/459(VOUTP_RESSCNTDODRNGL_cnt) -> bus_creator/459
  outpmodule/458(VOUTP_RESSCNTDODRNGR_cnt) -> bus_creator/458
  outpmodule/621(VOUTP_Variation_cnt) -> bus_creator/621
  outpmodule/456(VOUTP_QTYPSATRIPSR_cnt) -> bus_creator/456
  outpmodule/453(VOUTP_AvgBattTempOVCL_C) -> bus_creator/453
  outpmodule/751(VOUTP_VehAcclLimitTG_mps2) -> bus_creator/751
  outpmodule/455(VOUTP_AvgBattTempOFFL_C) -> bus_creator/455
  outpmodule/448(VOUTP_CDEODTR_km) -> bus_creator/448
  outpmodule/798(VOUTP_EC1EMReqSpdCtrlUpLmt_rpm) -> bus_creator/798
  outpmodule/447(VOUTP_ResetCDEODTR_km) -> bus_creator/447
  outpmodule/446(VOUTP_PKEL_kphsqr) -> bus_creator/446
  outpmodule/587(VOUTP_DCVol_V) -> bus_creator/587
  outpmodule/443(VOUTP_RESSV2XENNONPSAR_kWh) -> bus_creator/443
  outpmodule/836(VOUTP_ReqV2LIVIPopup_enum) -> bus_creator/836
  outpmodule/444(VOUTP_RESSV2XENNONPSAL_kWh) -> bus_creator/444
  outpmodule/441(VOUTP_GECHGOVCACR_kWh) -> bus_creator/441
  outpmodule/437(VOUTP_TGEOVCR_kWh) -> bus_creator/437
  outpmodule/937(VOUTP_APSReq_enum) -> bus_creator/937
  outpmodule/436(VOUTP_TEBPSAL_kWh) -> bus_creator/436
  outpmodule/438(VOUTP_TGEOVCL_kWh) -> bus_creator/438
  outpmodule/431(VOUTP_TNBCPSAR_Ahr) -> bus_creator/431
  outpmodule/433(VOUTP_TNECPSAR_kWh) -> bus_creator/433
  outpmodule/430(VOUTP_IGNCNTR_cnt) -> bus_creator/430
  outpmodule/427(VOUTP_CPSAL_sec) -> bus_creator/427
  outpmodule/428(VOUTP_HVBNAH_Ahr) -> bus_creator/428
  outpmodule/424(VOUTP_IPSAR_sec) -> bus_creator/424
  outpmodule/423(VOUTP_PSAL_sec) -> bus_creator/423
  outpmodule/422(VOUTP_PSAR_sec) -> bus_creator/422
  outpmodule/420(VOUTP_NUMPSATRIPSFLTMEMCLR_cnt) -> bus_creator/420
  outpmodule/419(VOUTP_HVESSENER_Whps) -> bus_creator/419
  outpmodule/418(VOUTP_HVESSCHARGEACT_kW) -> bus_creator/418
  outpmodule/416(VOUTP_HVBCellVoltMax_V) -> bus_creator/416
  outpmodule/414(VOUTP_BATSOH_pct) -> bus_creator/414
  outpmodule/413(VOUTP_ODOMETER_km) -> bus_creator/413
  outpmodule/412(VOUTP_HEVBATT_V) -> bus_creator/412
  outpmodule/834(VOUTP_RrTMTqReq_Nm) -> bus_creator/834
  outpmodule/410(VOUTP_CLRTIME_min) -> bus_creator/410
  outpmodule/407(VOUTP_APPD_pct) -> bus_creator/407
  outpmodule/916(VOUTP_LVDAWarning_flg) -> bus_creator/916
  outpmodule/404(VOUTP_MILDIST_km) -> bus_creator/404
  outpmodule/405(VOUTP_WARMUPS_cnt) -> bus_creator/405
  outpmodule/403(VOUTP_RUNTM_s) -> bus_creator/403
  outpmodule/479(VOUTP_PKERNumerator_kphsqr) -> bus_creator/479
  outpmodule/909(VOUTP_ADASISASta_enum) -> bus_creator/909
  outpmodule/475(VOUTP_RESSTIMESOCRNGAXIS_enum) -> bus_creator/475
  outpmodule/776(VOUTP_RC1PctTrqP4_pct) -> bus_creator/776
  outpmodule/515(VOUTP_DISCSta_enum) -> bus_creator/515
  outpmodule/512(VOUTP_JudgeKeepUnlockZone_flg) -> bus_creator/512
  outpmodule/506(VOUTP_UIDLowPowerSta_enum) -> bus_creator/506
  outpmodule/507(VOUTP_DkeyAreaRAPSSta_enum) -> bus_creator/507
  outpmodule/501(VOUTP_KeyAreaLockUnlock_enum) -> bus_creator/501
  outpmodule/500(VOUTP_KeyAreaPS_enum) -> bus_creator/500
  outpmodule/498(VOUTP_KeyModeSta_enum) -> bus_creator/498
  outpmodule/496(VOUTP_TimeSNDKCFbk_cnt) -> bus_creator/496
  outpmodule/488(VOUTP_VinCode_cnt) -> bus_creator/488
  outpmodule/486(VOUTP_OFFL_sec) -> bus_creator/486
  outpmodule/483(VOUTP_OVCR_sec) -> bus_creator/483
  outpmodule/388(VOUTP_VCUBrkSWSta_enum) -> bus_creator/388
  outpmodule/387(VOUTP_MCUActDisFail_flg) -> bus_creator/387
  outpmodule/384(VOUTP_EDriveSysErrShifterErr_flg) -> bus_creator/384
  outpmodule/382(VOUTP_VCURAPSErrLv2_flg) -> bus_creator/382
  outpmodule/379(VOUTP_DTCDetect_enum) -> bus_creator/379
  outpmodule/380(VOUTP_EngagePFail_flg) -> bus_creator/380
  outpmodule/377(VOUTP_EPBUnlockTODTC_raw32) -> bus_creator/377
  outpmodule/376(VOUTP_EPBLockTODTC_raw32) -> bus_creator/376
  outpmodule/375(VOUTP_5vAPS2PwrErrDTC_raw32) -> bus_creator/375
  outpmodule/373(VOUTP_C1EPAS2LCDTC_raw32) -> bus_creator/373
  outpmodule/372(VOUTP_RRSensorFailDTC_raw32) -> bus_creator/372
  outpmodule/743(VOUTP_TPMSSensorIDRegStart_flg) -> bus_creator/743
  outpmodule/374(VOUTP_5vAPS1PwrErrDTC_raw32) -> bus_creator/374
  outpmodule/370(VOUTP_RFSensorFailDTC_raw32) -> bus_creator/370
  outpmodule/548(VOUTP_VCUMCUFailRst_flg) -> bus_creator/548
  outpmodule/369(VOUTP_LFSensorFailDTC_raw32) -> bus_creator/369
  outpmodule/365(VOUTP_LFWheelTmpHighDTC_raw32) -> bus_creator/365
  outpmodule/362(VOUTP_RFPressIndiDTC_raw32) -> bus_creator/362
  outpmodule/364(VOUTP_RRPressIndiDTC_raw32) -> bus_creator/364
  outpmodule/363(VOUTP_LRPressIndiDTC_raw32) -> bus_creator/363
  outpmodule/360(VOUTP_RRBatwarnDTC_raw32) -> bus_creator/360
  outpmodule/356(VOUTP_RrMCUTqErrDTC_raw32) -> bus_creator/356
  outpmodule/355(VOUTP_FrMCUTqErrDTC_raw32) -> bus_creator/355
  outpmodule/626(VOUTP_SHA1_cnt) -> bus_creator/626
  outpmodule/353(VOUTP_ESC5RCErrDTC_raw32) -> bus_creator/353
  outpmodule/351(VOUTP_ESC1RCErrDTC_raw32) -> bus_creator/351
  outpmodule/352(VOUTP_ESC1CSErrDTC_raw32) -> bus_creator/352
  outpmodule/350(VOUTP_ESC7CSErrDTC_raw32) -> bus_creator/350
  outpmodule/348(VOUTP_Shifter1CSErrDTC_raw32) -> bus_creator/348
  outpmodule/347(VOUTP_Shifter1RCErrDTC_raw32) -> bus_creator/347
  outpmodule/345(VOUTP_MCUF1CSErrDTC_raw32) -> bus_creator/345
  outpmodule/346(VOUTP_MCUR1CSErrDTC_raw32) -> bus_creator/346
  outpmodule/344(VOUTP_MCUR1RCErrDTC_raw32) -> bus_creator/344
  outpmodule/343(VOUTP_MCUF1RCErrDTC_raw32) -> bus_creator/343
  outpmodule/341(VOUTP_MSAMalfuncDetDTC_raw32) -> bus_creator/341
  outpmodule/340(VOUTP_CCMalfuncDetDTC_raw32) -> bus_creator/340
  outpmodule/337(VOUTP_CCUSigErrDetDTC_raw32) -> bus_creator/337
  outpmodule/931(VOUTP_MSACtrlSta_enum) -> bus_creator/931
  outpmodule/335(VOUTP_FrMCUSigErrDetDTC_raw32) -> bus_creator/335
  outpmodule/336(VOUTP_RrMCUSigErrDetDTC_raw32) -> bus_creator/336
  outpmodule/333(VOUTP_BMSSigErrDetDTC_raw32) -> bus_creator/333
  outpmodule/371(VOUTP_LRSensorFailDTC_raw32) -> bus_creator/371
  outpmodule/334(VOUTP_FCMACCSigErrDetDTC_raw32) -> bus_creator/334
  outpmodule/331(VOUTP_FCM5CSErrDTC_raw32) -> bus_creator/331
  outpmodule/813(VOUTP_RC1RetSpdIdleP1_rpm) -> bus_creator/813
  outpmodule/329(VOUTP_FCM4CSErrDTC_raw32) -> bus_creator/329
  outpmodule/326(VOUTP_FCM3RCErrDTC_raw32) -> bus_creator/326
  outpmodule/323(VOUTP_FCM2RCErrDTC_raw32) -> bus_creator/323
  outpmodule/325(VOUTP_FCM3NoComDTC_raw32) -> bus_creator/325
  outpmodule/324(VOUTP_FCM2CSErrDTC_raw32) -> bus_creator/324
  outpmodule/322(VOUTP_FCM2NoComDTC_raw32) -> bus_creator/322
  outpmodule/320(VOUTP_RLLUSSDTC_raw32) -> bus_creator/320
  outpmodule/394(VOUTP_VCUHoodSWSta_flg) -> bus_creator/394
  outpmodule/396(VOUTP_ActAPSPosn_pct) -> bus_creator/396
  outpmodule/557(VOUTP_V2BAux1OnOff_enum) -> bus_creator/557
  outpmodule/393(VOUTP_SysAllowReadySta_flg) -> bus_creator/393
  outpmodule/317(VOUTP_RCRUSSDTC_raw32) -> bus_creator/317
  outpmodule/316(VOUTP_RMRUSSDTC_raw32) -> bus_creator/316
  outpmodule/314(VOUTP_RCLUSSDTC_raw32) -> bus_creator/314
  outpmodule/670(VOUTP_TPMSCaliButtAllow_flg) -> bus_creator/670
  outpmodule/313(VOUTP_FCRUSSDTC_raw32) -> bus_creator/313
  outpmodule/311(VOUTP_FMLUSSDTC_raw32) -> bus_creator/311
  outpmodule/309(VOUTP_DiagRRTSDTC_raw32) -> bus_creator/309
  outpmodule/310(VOUTP_FCLUSSDTC_raw32) -> bus_creator/310
  outpmodule/378(VOUTP_LimpHomeActTmp_flg) -> bus_creator/378
  outpmodule/658(VOUTP_RFWheelTemp_C) -> bus_creator/658
  outpmodule/308(VOUTP_DiagRLTSDTC_raw32) -> bus_creator/308
  outpmodule/647(VOUTP_CoolFanReq_pct) -> bus_creator/647
  outpmodule/306(VOUTP_DiagFLTSDTC_raw32) -> bus_creator/306
  outpmodule/304(VOUTP_EnterNewOperCyc_flg) -> bus_creator/304
  outpmodule/723(VOUTP_WriteChkRFID_raw) -> bus_creator/723
  outpmodule/955(VOUTP_FDCVMCMaxAngCtrlOutTqLim_Nm) -> bus_creator/955
  outpmodule/302(VOUTP_ESC1NoComDTC_raw32) -> bus_creator/302
  outpmodule/409(VOUTP_MILTIME_min) -> bus_creator/409
  outpmodule/301(VOUTP_ESC7NoComDTC_raw32) -> bus_creator/301
  outpmodule/300(VOUTP_Shifter1NoComDTC_raw32) -> bus_creator/300
  outpmodule/297(VOUTP_APSCorrErrDTC_raw32) -> bus_creator/297
  outpmodule/296(VOUTP_APS2SigOoRDTC_raw32) -> bus_creator/296
  outpmodule/293(VOUTP_EDriveSysErrVCUErr_flg) -> bus_creator/293
  outpmodule/473(VOUTP_PROTOCOLID_enum) -> bus_creator/473
  outpmodule/294(VOUTP_VehMalfunLevel_enum) -> bus_creator/294
  outpmodule/472(VOUTP_AVGBATTEMPL_C) -> bus_creator/472
  outpmodule/887(VOUTP_ADASShftPosnReqA_flg) -> bus_creator/887
  outpmodule/291(VOUTP_HoodSWDTC_raw32) -> bus_creator/291
  outpmodule/549(VOUTP_HVILFail_flg) -> bus_creator/549
  outpmodule/290(VOUTP_RRDoorSWDTC_raw32) -> bus_creator/290
  outpmodule/289(VOUTP_FRDoorSWDTC_raw32) -> bus_creator/289
  outpmodule/664(VOUTP_RRSensorFail_flg) -> bus_creator/664
  outpmodule/287(VOUTP_FLDoorSWDTC_raw32) -> bus_creator/287
  outpmodule/285(VOUTP_LVSupHiDTC_raw32) -> bus_creator/285
  outpmodule/484(VOUTP_OVCL_sec) -> bus_creator/484
  outpmodule/283(VOUTP_IniLVLoDTC_raw32) -> bus_creator/283
  outpmodule/282(VOUTP_OBC4PreDTC_raw32) -> bus_creator/282
  outpmodule/281(VOUTP_MCUActDTC_raw32) -> bus_creator/281
  outpmodule/951(VOUTP_FDCVMCAPSAngleTarget_deg) -> bus_creator/951
  outpmodule/278(VOUTP_MCUDisDTC_raw32) -> bus_creator/278
  outpmodule/280(VOUTP_HVRlyOpDTC_raw32) -> bus_creator/280
  outpmodule/279(VOUTP_DCDCDisDTC_raw32) -> bus_creator/279
  outpmodule/622(VOUTP_Dash1_cnt) -> bus_creator/622
  outpmodule/276(VOUTP_HiLvSaChkDTC_raw32) -> bus_creator/276
  outpmodule/797(VOUTP_EC1EMReqTrqCtrlLoLmt_pct) -> bus_creator/797
  outpmodule/275(VOUTP_DCDCEnaDTC_raw32) -> bus_creator/275
  outpmodule/274(VOUTP_BMSRdyDTC_raw32) -> bus_creator/274
  outpmodule/429(VOUTP_HVBNE_kWh) -> bus_creator/429
  outpmodule/796(VOUTP_EC1EMReqSpdCtrlLoLmt_rpm) -> bus_creator/796
  outpmodule/271(VOUTP_MCU4PreDTC_raw32) -> bus_creator/271
  outpmodule/273(VOUTP_HVRlyCloDTC_raw32) -> bus_creator/273
  outpmodule/318(VOUTP_FLLUSSDTC_raw32) -> bus_creator/318
  outpmodule/270(VOUTP_HVB4PreDTC_raw32) -> bus_creator/270
  outpmodule/269(VOUTP_ONtoRdyDTC_raw32) -> bus_creator/269
  outpmodule/266(VOUTP_BrkSWErrDTC_raw32) -> bus_creator/266
  outpmodule/265(VOUTP_Lv4ErrDTC_raw32) -> bus_creator/265
  outpmodule/262(VOUTP_Lv1ErrDTC_raw32) -> bus_creator/262
  outpmodule/259(VOUTP_C1ABM1RCDTC_raw32) -> bus_creator/259
  outpmodule/258(VOUTP_C3CCU2LCDTC_raw32) -> bus_creator/258
  outpmodule/601(VOUTP_DTbyte4_raw) -> bus_creator/601
  outpmodule/257(VOUTP_C3CCU2CSDTC_raw32) -> bus_creator/257
  outpmodule/593(VOUTP_CFGEM1BAMTNum_raw) -> bus_creator/593
  outpmodule/253(VOUTP_C3CCU1RCDTC_raw32) -> bus_creator/253
  outpmodule/298(VOUTP_MCUF1NoComDTC_raw32) -> bus_creator/298
  outpmodule/252(VOUTP_C3BMS1LCDTC_raw32) -> bus_creator/252
  outpmodule/755(VOUTP_ActDriveMode_enum) -> bus_creator/755
  outpmodule/251(VOUTP_C3BMS1CSDTC_raw32) -> bus_creator/251
  outpmodule/250(VOUTP_C3BMS1RCDTC_raw32) -> bus_creator/250
  outpmodule/520(VOUTP_CSB_flg) -> bus_creator/520
  outpmodule/245(VOUTP_WakeUp_flg) -> bus_creator/245
  outpmodule/556(VOUTP_V2BLifeSig_cnt) -> bus_creator/556
  outpmodule/244(VOUTP_FDCBCMTurnBuzzerENSta_flg) -> bus_creator/244
  outpmodule/246(VOUTP_KeepWakeUp_flg) -> bus_creator/246
  outpmodule/242(VOUTP_FDCBCMRGearSta_flg) -> bus_creator/242
  outpmodule/511(VOUTP_FDCDKCAllowSleep_flg) -> bus_creator/511
  outpmodule/239(VOUTP_FDCBCMMDCloseSVCmd_flg) -> bus_creator/239
  outpmodule/238(VOUTP_FDCBCMMDOpenSVCmd_flg) -> bus_creator/238
  outpmodule/226(VOUTP_FDCBCMRoomLpSetSta_flg) -> bus_creator/226
  outpmodule/224(VOUTP_FDCBCMInnerBuzzerCmd_flg) -> bus_creator/224
  outpmodule/221(VOUTP_FDCBCMRBSDYCmd_flg) -> bus_creator/221
  outpmodule/218(VOUTP_FDCBCMLBSDRCmd_flg) -> bus_creator/218
  outpmodule/219(VOUTP_FDCBCMLBSDYCmd_flg) -> bus_creator/219
  outpmodule/217(VOUTP_FDCBCMRoomLpAmbCmd_flg) -> bus_creator/217
  outpmodule/215(VOUTP_FDCBCMMDoorSta_flg) -> bus_creator/215
  outpmodule/214(VOUTP_FDCBCMFDoorSta_flg) -> bus_creator/214
  outpmodule/212(VOUTP_FDCBCMRFLampCmd_flg) -> bus_creator/212
  outpmodule/208(VOUTP_FDCBCMWasherCmd_flg) -> bus_creator/208
  outpmodule/328(VOUTP_FCM4NoComDTC_raw32) -> bus_creator/328
  outpmodule/788(VOUTP_EC1PercTorqIdleP3_pct) -> bus_creator/788
  outpmodule/207(VOUTP_FDCBCMWiperHCmd_flg) -> bus_creator/207
  outpmodule/415(VOUTP_HVBCellVoltMin_V) -> bus_creator/415
  outpmodule/204(VOUTP_FDCBCMSTOPBALLCmd_flg) -> bus_creator/204
  outpmodule/440(VOUTP_GECHGOVCDCL_kWh) -> bus_creator/440
  outpmodule/201(VOUTP_FDCBCMLTurnLpCmd_flg) -> bus_creator/201
  outpmodule/467(VOUTP_RESSTIMESOCCHGRNGL_s) -> bus_creator/467
  outpmodule/198(VOUTP_FDCBCMBSDBuzzerCmd_flg) -> bus_creator/198
  outpmodule/411(VOUTP_BATSOC_pct) -> bus_creator/411
  outpmodule/194(VOUTP_FDCBCMSMKLCmd_flg) -> bus_creator/194
  outpmodule/663(VOUTP_LRSensorFail_flg) -> bus_creator/663
  outpmodule/191(VOUTP_FDCBCMLBeamCmd_flg) -> bus_creator/191
  outpmodule/186(VOUTP_RAPSBCMLockReq_flg) -> bus_creator/186
  outpmodule/183(VOUTP_APSSpeedCMD_kph) -> bus_creator/183
  outpmodule/182(VOUTP_APSShiftPosnReq_enum) -> bus_creator/182
  outpmodule/180(VOUTP_PUIDLowPower_flg) -> bus_creator/180
  outpmodule/445(VOUTP_PKER_kphsqr) -> bus_creator/445
  outpmodule/181(VOUTP_CAASVMCReqA_flg) -> bus_creator/181
  outpmodule/175(VOUTP_APSVRqEPASCtrl_flg) -> bus_creator/175
  outpmodule/173(VOUTP_APSExitCondition_enum) -> bus_creator/173
  outpmodule/170(VOUTP_APSRQDisplay_enum) -> bus_creator/170
  outpmodule/168(VOUTP_DriverSeatBeltCmdTimeOut_flg) -> bus_creator/168
  outpmodule/452(VOUTP_AvgBattTempOVCR_C) -> bus_creator/452
  outpmodule/167(VOUTP_DriverSeatBeltCmd_flg) -> bus_creator/167
  outpmodule/164(VOUTP_ABSActiveTimeOut_flg) -> bus_creator/164
  outpmodule/165(VOUTP_TCSActive_flg) -> bus_creator/165
  outpmodule/161(VOUTP_IVIScreen_enum) -> bus_creator/161
  outpmodule/268(VOUTP_KeyAuthDTC_raw32) -> bus_creator/268
  outpmodule/417(VOUTP_HVESSCHARGELIM_kW) -> bus_creator/417
  outpmodule/157(VOUTP_IVIStatus_flg) -> bus_creator/157
  outpmodule/247(VOUTP_C3BMS6RCDTC_raw32) -> bus_creator/247
  outpmodule/700(VOUTP_RFP20_raw8) -> bus_creator/700
  outpmodule/235(VOUTP_FDCBCMEmSVCmd_flg) -> bus_creator/235
  outpmodule/236(VOUTP_FDCBCMFDOpenSVCmd_flg) -> bus_creator/236
  outpmodule/514(VOUTP_DISCTargetSpd_kph) -> bus_creator/514
  outpmodule/231(VOUTP_FDCBCMRRoomLpSetSta_pct) -> bus_creator/231
  outpmodule/229(VOUTP_FDCBCMMRoomLpSetSta_pct) -> bus_creator/229
  outpmodule/154(VOUTP_AVMParkingmodeTimeOut_flg) -> bus_creator/154
  outpmodule/155(VOUTP_AVMErrSTA_flg) -> bus_creator/155
  outpmodule/402(VOUTP_VSS_kph) -> bus_creator/402
  outpmodule/152(VOUTP_AVMparkingexcuteTimeOut_flg) -> bus_creator/152
  outpmodule/383(VOUTP_VCURAPSErrLv3_flg) -> bus_creator/383
  outpmodule/150(VOUTP_AVMparkingcancelTimeOut_flg) -> bus_creator/150
  outpmodule/696(VOUTP_S3L_enum) -> bus_creator/696
  outpmodule/147(VOUTP_EPBSta_enum) -> bus_creator/147
  outpmodule/653(VOUTP_LFWheelPress_raw8) -> bus_creator/653
  outpmodule/145(VOUTP_EPBErrSta_enum) -> bus_creator/145
  outpmodule/521(VOUTP_ErrorState_enum) -> bus_creator/521
  outpmodule/140(VOUTP_ESCAPSStaTimeOut_flg) -> bus_creator/140
  outpmodule/367(VOUTP_LRWheelTmpHighDTC_raw32) -> bus_creator/367
  outpmodule/141(VOUTP_EPBExtReleaseAvail_flg) -> bus_creator/141
  outpmodule/138(VOUTP_ESCStandstillTimeOut_flg) -> bus_creator/138
  outpmodule/136(VOUTP_BrkSwVTimeOut_flg) -> bus_creator/136
  outpmodule/134(VOUTP_BrkSwStaTimeOut_flg) -> bus_creator/134
  outpmodule/135(VOUTP_BrkSwV_flg) -> bus_creator/135
  outpmodule/133(VOUTP_BrkSwSta_flg) -> bus_creator/133
  outpmodule/129(VOUTP_LongAccelV_flg) -> bus_creator/129
  outpmodule/480(VOUTP_PKELNumerator_kphsqr) -> bus_creator/480
  outpmodule/131(VOUTP_MCPressureV_bar) -> bus_creator/131
  outpmodule/399(VOUTP_ResetPedalZeroPosStart_flg) -> bus_creator/399
  outpmodule/655(VOUTP_LRWheelPress_raw8) -> bus_creator/655
  outpmodule/127(VOUTP_LatAccelV_flg) -> bus_creator/127
  outpmodule/124(VOUTP_MCPressureTimeOut_flg) -> bus_creator/124
  outpmodule/125(VOUTP_YawRateV_flg) -> bus_creator/125
  outpmodule/126(VOUTP_YawRateVTimeOut_flg) -> bus_creator/126
  outpmodule/121(VOUTP_LongAccel_Gps) -> bus_creator/121
  outpmodule/457(VOUTP_QTYPSATRIPSL_cnt) -> bus_creator/457
  outpmodule/120(VOUTP_LatAccelTimeOut_flg) -> bus_creator/120
  outpmodule/115(VOUTP_GRADE_Deg) -> bus_creator/115
  outpmodule/112(VOUTP_SASCALTimeOut_flg) -> bus_creator/112
  outpmodule/113(VOUTP_SASV_flg) -> bus_creator/113
  outpmodule/108(VOUTP_SASSpeedTimeOut_flg) -> bus_creator/108
  outpmodule/107(VOUTP_SASSpeed_degps) -> bus_creator/107
  outpmodule/105(VOUTP_SASAngle_Deg) -> bus_creator/105
  outpmodule/104(VOUTP_EPSAOIControlTimeOut_flg) -> bus_creator/104
  outpmodule/103(VOUTP_EPSAOIControl_enum) -> bus_creator/103
  outpmodule/98(VOUTP_RRPulseCountTimeOut_flg) -> bus_creator/98
  outpmodule/97(VOUTP_RRPulseCount_enum) -> bus_creator/97
  outpmodule/95(VOUTP_LRPulseCount_enum) -> bus_creator/95
  outpmodule/92(VOUTP_LFPulseCountTimeOut_flg) -> bus_creator/92
  outpmodule/90(VOUTP_RRPulseCountVTimeOut_flg) -> bus_creator/90
  outpmodule/89(VOUTP_RRPulseCountV_flg) -> bus_creator/89
  outpmodule/509(VOUTP_KeyNumSta_enum) -> bus_creator/509
  outpmodule/86(VOUTP_RFPulseCountVTimeOut_flg) -> bus_creator/86
  outpmodule/83(VOUTP_LFPulseCountV_flg) -> bus_creator/83
  outpmodule/81(VOUTP_RRWhlRotDir_enum) -> bus_creator/81
  outpmodule/77(VOUTP_RFWhlRotDir_enum) -> bus_creator/77
  outpmodule/877(VOUTP_ADASDBSReq_enum) -> bus_creator/877
  outpmodule/879(VOUTP_ACCObjDist_m) -> bus_creator/879
  outpmodule/600(VOUTP_DTbyte3_raw) -> bus_creator/600
  outpmodule/878(VOUTP_ADASACCSta_enum) -> bus_creator/878
  outpmodule/876(VOUTP_ACCVehHoldReq_flg) -> bus_creator/876
  outpmodule/660(VOUTP_RRWheelTemp_C) -> bus_creator/660
  outpmodule/875(VOUTP_AEBVehHoldReq_flg) -> bus_creator/875
  outpmodule/631(VOUTP_SHA6_cnt) -> bus_creator/631
  outpmodule/871(VOUTP_LKATOIFault_flg) -> bus_creator/871
  outpmodule/735(VOUTP_FlashS1ID_raw) -> bus_creator/735
  outpmodule/870(VOUTP_LKAStrToqReq_Nm) -> bus_creator/870
  outpmodule/332(VOUTP_ZoneSCPNoComDTC_raw32) -> bus_creator/332
  outpmodule/390(VOUTP_VCUFRDoorSta_flg) -> bus_creator/390
  outpmodule/869(VOUTP_ADASLKASta_enum) -> bus_creator/869
  outpmodule/80(VOUTP_LRWhlRotDirTimeOut_flg) -> bus_creator/80
  outpmodule/867(VOUTP_ActACCRequiredAccel_mps2) -> bus_creator/867
  outpmodule/863(VOUTP_ISOJerkLimit_mps3) -> bus_creator/863
  outpmodule/537(VOUTP_IGNRlyClose_flg) -> bus_creator/537
  outpmodule/862(VOUTP_ISODecLimit_mps2) -> bus_creator/862
  outpmodule/361(VOUTP_LFPressIndiDTC_raw32) -> bus_creator/361
  outpmodule/858(VOUTP_SafetyCtrl_flg) -> bus_creator/858
  outpmodule/859(VOUTP_SPD2ACCAct_flg) -> bus_creator/859
  outpmodule/857(VOUTP_LatAccCtrl_flg) -> bus_creator/857
  outpmodule/856(VOUTP_SingleWhlSlipRatioCtrl_flg) -> bus_creator/856
  outpmodule/853(VOUTP_LimitPCT_pct) -> bus_creator/853
  outpmodule/854(VOUTP_FrontRearSlipRatioCtrl_flg) -> bus_creator/854
  outpmodule/849(VOUTP_VMCMSACtrlAvail_flg) -> bus_creator/849
  outpmodule/847(VOUTP_VMCACCCtrlAvail_flg) -> bus_creator/847
  outpmodule/110(VOUTP_SASSpeedValidTimeOut_flg) -> bus_creator/110
  outpmodule/846(VOUTP_VMCAEBCtrlAvail_flg) -> bus_creator/846
  outpmodule/848(VOUTP_VMCCCCtrlAvail_flg) -> bus_creator/848
  outpmodule/844(VOUTP_VehicleSpeed_kph) -> bus_creator/844
  outpmodule/523(VOUTP_PNI_flg) -> bus_creator/523
  outpmodule/845(VOUTP_MeterIndSpeed_raw32) -> bus_creator/845
  outpmodule/880(VOUTP_ACCObjRelSpd_mps) -> bus_creator/880
  outpmodule/553(VOUTP_ChrgBCUHVFail_flg) -> bus_creator/553
  outpmodule/882(VOUTP_ACCJerkUpperLimit_mps3) -> bus_creator/882
  outpmodule/93(VOUTP_RFPulseCount_enum) -> bus_creator/93
  outpmodule/27(VOUTP_PASDFCR_cm) -> bus_creator/27
  outpmodule/57(VOUTP_BrkPedalPos_pct) -> bus_creator/57
  outpmodule/55(VOUTP_StaFSya_flg) -> bus_creator/55
  outpmodule/562(VOUTP_V2BACPosRlySta_enum) -> bus_creator/562
  outpmodule/53(VOUTP_Chime_enum) -> bus_creator/53
  outpmodule/54(VOUTP_SNSRLayout_enum) -> bus_creator/54
  outpmodule/888(VOUTP_ADASShftPosnReq_enum) -> bus_creator/888
  outpmodule/52(VOUTP_USSStaFCL_flg) -> bus_creator/52
  outpmodule/51(VOUTP_USSStaFCR_flg) -> bus_creator/51
  outpmodule/49(VOUTP_USSStaFLR_flg) -> bus_creator/49
  outpmodule/48(VOUTP_USSStaFML_flg) -> bus_creator/48
  outpmodule/497(VOUTP_KeyMissSta_flg) -> bus_creator/497
  outpmodule/47(VOUTP_USSStaFMR_flg) -> bus_creator/47
  outpmodule/44(VOUTP_USSStaRLL_flg) -> bus_creator/44
  outpmodule/42(VOUTP_USSStaRML_flg) -> bus_creator/42
  outpmodule/943(VOUTP_ExtraMSACtrlSta_enum) -> bus_creator/943
  outpmodule/43(VOUTP_USSStaRLR_flg) -> bus_creator/43
  outpmodule/40(VOUTP_PASAFCR_enum) -> bus_creator/40
  outpmodule/38(VOUTP_PASAFMR_enum) -> bus_creator/38
  outpmodule/546(VOUTP_ActiveDischargeReq_enum) -> bus_creator/546
  outpmodule/37(VOUTP_PASARCL_enum) -> bus_creator/37
  outpmodule/533(VOUTP_PowerUpFault_enum) -> bus_creator/533
  outpmodule/770(VOUTP_EVCU1EBrakeTorqLow_enum) -> bus_creator/770
  outpmodule/36(VOUTP_PASARCR_enum) -> bus_creator/36
  outpmodule/35(VOUTP_PASARML_enum) -> bus_creator/35
  outpmodule/288(VOUTP_RLDoorSWDTC_raw32) -> bus_creator/288
  outpmodule/510(VOUTP_KeyTypeSta_enum) -> bus_creator/510
  outpmodule/701(VOUTP_LRP20_raw8) -> bus_creator/701
  outpmodule/34(VOUTP_PASARMR_enum) -> bus_creator/34
  outpmodule/30(VOUTP_APSDRLL_cm) -> bus_creator/30
  outpmodule/29(VOUTP_APSDRLR_cm) -> bus_creator/29
  outpmodule/482(VOUTP_BattTempPSAL_sec) -> bus_creator/482
  outpmodule/22(VOUTP_PASDRML_cm) -> bus_creator/22
  outpmodule/19(VOUTP_FSOffSwTimeOut_flg) -> bus_creator/19
  outpmodule/17(VOUTP_VehSpeedTimeOut_flg) -> bus_creator/17
  outpmodule/16(VOUTP_VehSpeed_kph) -> bus_creator/16
  outpmodule/833(VOUTP_FrTMTqReq_Nm) -> bus_creator/833
  outpmodule/9(VOUTP_EHPSMotorDemSpd_rpm) -> bus_creator/9
  outpmodule/6(VOUTP_CACOverrun_flg) -> bus_creator/6
  outpmodule/5(VOUTP_EHPSEnDemand_enum) -> bus_creator/5
  outpmodule/4(VOUTP_CACPresReady_flg) -> bus_creator/4
  outpmodule/2(VOUTP_CACTempOverHigh_flg) -> bus_creator/2
  outpmodule/1(VOUTP_EACEnDemand_enum) -> bus_creator/1
  outpmodule/26(VOUTP_PASDFML_cm) -> bus_creator/26
  outpmodule/264(VOUTP_Lv3ErrDTC_raw32) -> bus_creator/264
  outpmodule/25(VOUTP_PASDFMR_cm) -> bus_creator/25
  outpmodule/24(VOUTP_PASDRCL_cm) -> bus_creator/24
  bus_selector19/3 -> outpmodule/844(VVMC_VehicleSpeed_kph)  "<VVMC_VehicleSpeed_kph>"
  bus_selector19/19 -> outpmodule/860(VVMC_AccCalcuPID_mps2)  "<VVMC_AccCalcuPID_mps2>"
  bus_selector19/16 -> outpmodule/857(VVMC_LatAccCtrl_flg)  "<VVMC_LatAccCtrl_flg>"
  outpmodule/119(VOUTP_LatAccel_Gps) -> bus_creator/119
  bus_selector19/14 -> outpmodule/855(VVMC_RearWhlSlipRatioCtrl_flg)  "<VVMC_RearWhlSlipRatioCtrl_flg>"
  outpmodule/643(VOUTP_PmicBootPath_raw32) -> bus_creator/643
  bus_selector19/13 -> outpmodule/854(VVMC_FrontRearSlipRatioCtrl_flg)  "<VVMC_FrontRearSlipRatioCtrl_flg>"
  bus_selector19/11 -> outpmodule/852(VVMC_JerkPCT_pct)  "<VVMC_JerkPCT_pct>"
  outpmodule/648(VOUTP_AfterrunningMode_flg) -> bus_creator/648
  bus_selector19/7 -> outpmodule/848(VVMC_VMCCCCtrlAvail_flg)  "<VVMC_VMCCCCtrlAvail_flg>"
  outpmodule/579(VOUTP_VCULife2_cnt) -> bus_creator/579
  outpmodule/946(VOUTP_CalibratedAccZ_G) -> bus_creator/946
  bus_selector19/20 -> outpmodule/861(VVMC_ISOAccLimit_mps2)  "<VVMC_ISOAccLimit_mps2>"
  outpmodule/225(VOUTP_FDCBCMRoomLpAmbSetSta_flg) -> bus_creator/225
  bus_selector18/6 -> outpmodule/840(VV2L_HVPO120VGrpALDSt_enum)  "<VV2L_HVPO120VGrpALDSt_enum>"
  bus_selector18/5 -> outpmodule/839(VV2L_ReqOBCIntrV2LEna_enum)  "<VV2L_ReqOBCIntrV2LEna_enum>"
  outpmodule/172(VOUTP_APSHWVer_enum) -> bus_creator/172
  bus_selector18/7 -> outpmodule/841(VV2L_HVPO120VGrpBLDSt_enum)  "<VV2L_HVPO120VGrpBLDSt_enum>"
  outpmodule/905(VOUTP_ADASLFCSta_enum) -> bus_creator/905
  BV2L_outputs/1 -> bus_selector18/1
  outpmodule/142(VOUTP_EPBExtReleaseAvailTimeOut_flg) -> bus_creator/142
  bus_selector18/3 -> outpmodule/837(VV2L_ReqV2LIVIDisChrg_enum)  "<VV2L_ReqV2LIVIDisChrg_enum>"
  bus_selector18/2 -> outpmodule/836(VV2L_ReqV2LIVIPopup_enum)  "<VV2L_ReqV2LIVIPopup_enum>"
  bus_selector18/1 -> outpmodule/835(VV2L_ReqOBCV2LEna_enum)  "<VV2L_ReqOBCV2LEna_enum>"
  outpmodule/45(VOUTP_USSStaRCR_flg) -> bus_creator/45
  outpmodule/525(VOUTP_WakeUp_enum) -> bus_creator/525
  bus_selector17/1 -> outpmodule/833(VTQR_FrTMTqReq_Nm)  "<VTQR_FrTMTqReq_Nm>"
  outpmodule/580(VOUTP_VSPFunc_enum) -> bus_creator/580
  bus_selector16/82 -> outpmodule/827(VTQD_EVCU1RecuperHighSta_enum)  "<VTQD_EVCU1RecuperHighSta_enum>"
  bus_selector16/80 -> outpmodule/825(VTQD_TUpAIND_enum)  "<VTQD_TUpAIND_enum>"
  outpmodule/248(VOUTP_C3BMS6CSDTC_raw32) -> bus_creator/248
  outpmodule/505(VOUTP_KeyAreaSPTGSta_enum) -> bus_creator/505
  bus_selector16/77 -> outpmodule/822(VTQD_VCUMCUDemLoNegVal_rpm)  "<VTQD_VCUMCUDemLoNegVal_rpm>"
  bus_selector16/74 -> outpmodule/819(VTQD_RC1RefRetTrq_Nm)  "<VTQD_RC1RefRetTrq_Nm>"
  bus_selector16/78 -> outpmodule/823(VTQD_VCUMCUDemSpd_rpm)  "<VTQD_VCUMCUDemSpd_rpm>"
  outpmodule/123(VOUTP_MCPressure_bar) -> bus_creator/123
  bus_selector16/76 -> outpmodule/821(VTQD_RC1RetSpdP4_rpm)  "<VTQD_RC1RetSpdP4_rpm>"
  outpmodule/610(VOUTP_CarModel3_cnt) -> bus_creator/610
  bus_selector16/69 -> outpmodule/814(VTQD_RC1PctTrqIdleP1_pct)  "<VTQD_RC1PctTrqIdleP1_pct>"
  outpmodule/400(VOUTP_EAPS1NRM_pct) -> bus_creator/400
  bus_selector16/68 -> outpmodule/813(VTQD_RC1RetSpdIdleP1_rpm)  "<VTQD_RC1RetSpdIdleP1_rpm>"
  outpmodule/599(VOUTP_DTbyte2_raw) -> bus_creator/599
  bus_selector16/67 -> outpmodule/812(VTQD_RC1RetCtrlMth_enum)  "<VTQD_RC1RetCtrlMth_enum>"
  outpmodule/425(VOUTP_IPSAL_sec) -> bus_creator/425
  bus_selector16/66 -> outpmodule/811(VTQD_RC1RetLocat_enum)  "<VTQD_RC1RetLocat_enum>"
  bus_selector16/65 -> outpmodule/810(VTQD_RC1RetType_enum)  "<VTQD_RC1RetType_enum>"
  bus_selector16/62 -> outpmodule/807(VTQD_EC1EMSupTSC1CtrlPG4_cnt)  "<VTQD_EC1EMSupTSC1CtrlPG4_cnt>"
  bus_selector16/58 -> outpmodule/803(VTQD_EC1EMSupVarRTSC1MSG_cnt)  "<VTQD_EC1EMSupVarRTSC1MSG_cnt>"
  outpmodule/852(VOUTP_JerkPCT_pct) -> bus_creator/852
  outpmodule/193(VOUTP_FDCBCMHBeamCmd_flg) -> bus_creator/193
  bus_selector16/57 -> outpmodule/802(VTQD_EC1EMDefTrqLmt_rpm)  "<VTQD_EC1EMDefTrqLmt_rpm>"
  outpmodule/545(VOUTP_DrivelineRelease_enum) -> bus_creator/545
  bus_selector16/55 -> outpmodule/800(VTQD_EC1EMExtRSCtrlUpLmt_rpm)  "<VTQD_EC1EMExtRSCtrlUpLmt_rpm>"
  outpmodule/762(VOUTP_TMTqReq_Nm) -> bus_creator/762
  bus_selector16/52 -> outpmodule/797(VTQD_EC1EMReqTrqCtrlLoLmt_pct)  "<VTQD_EC1EMReqTrqCtrlLoLmt_pct>"
  bus_selector16/49 -> outpmodule/794(VTQD_EC1EMMaxMEngOvrSP7_rpm)  "<VTQD_EC1EMMaxMEngOvrSP7_rpm>"
  outpmodule/686(VOUTP_LFSensorMode_flg) -> bus_creator/686
  bus_selector16/48 -> outpmodule/793(VTQD_EC1EMRefTorq_Nm)  "<VTQD_EC1EMRefTorq_Nm>"
  outpmodule/79(VOUTP_LRWhlRotDir_enum) -> bus_creator/79
  outpmodule/785(VOUTP_EC1EMSpdIdleP2_rpm) -> bus_creator/785
  bus_selector16/46 -> outpmodule/791(VTQD_EC1PercTorqIdleP5_pct)  "<VTQD_EC1PercTorqIdleP5_pct>"
  bus_selector16/39 -> outpmodule/784(VTQD_EC1PercTorqIdleP1_pct)  "<VTQD_EC1PercTorqIdleP1_pct>"
  outpmodule/544(VOUTP_HVSysReady_enum) -> bus_creator/544
  bus_selector16/35 -> outpmodule/780(VTQD_EMRC1ActEMOutSftSpd_rpm)  "<VTQD_EMRC1ActEMOutSftSpd_rpm>"
  bus_selector16/33 -> outpmodule/778(VTQD_EMRC1EMTquModeDrvBrk_enum)  "<VTQD_EMRC1EMTquModeDrvBrk_enum>"
  outpmodule/188(VOUTP_RAPSErrWarnSta_enum) -> bus_creator/188
  outpmodule/470(VOUTP_MAXBATTEMPL_C) -> bus_creator/470
  bus_selector16/31 -> outpmodule/776(VTQD_RC1PctTrqP4_pct)  "<VTQD_RC1PctTrqP4_pct>"
  bus_selector16/32 -> outpmodule/777(VTQD_RC1PctTrqPekTrqP5_pct)  "<VTQD_RC1PctTrqPekTrqP5_pct>"
  bus_selector16/28 -> outpmodule/773(VTQD_EEC3NFricPercTorq_pct)  "<VTQD_EEC3NFricPercTorq_pct>"
  outpmodule/642(VOUTP_ECUGen2_cnt) -> bus_creator/642
  bus_selector16/29 -> outpmodule/774(VTQD_EEC3EMPressLoss_pct)  "<VTQD_EEC3EMPressLoss_pct>"
  outpmodule/542(VOUTP_EHPSRlyDem_enum) -> bus_creator/542
  bus_selector16/26 -> outpmodule/771(VTQD_EVCU2MaxTorqAvail_pct)  "<VTQD_EVCU2MaxTorqAvail_pct>"
  bus_selector16/22 -> outpmodule/767(VTQD_EVCU1EMotorSpd_rpm)  "<VTQD_EVCU1EMotorSpd_rpm>"
  bus_selector16/21 -> outpmodule/766(VTQD_EVCU1WheelSlipdet_enum)  "<VTQD_EVCU1WheelSlipdet_enum>"
  outpmodule/197(VOUTP_FDCBCMDVRSignalRCmd_flg) -> bus_creator/197
  outpmodule/469(VOUTP_RESSTIMESOCOFFRNGL_s) -> bus_creator/469
  outpmodule/917(VOUTP_LVDAACCStatusInformation_flg) -> bus_creator/917
  bus_selector16/17 -> outpmodule/762(VTQD_TMTqReq_Nm)  "<VTQD_TMTqReq_Nm>"
  bus_selector16/15 -> outpmodule/760(VTQD_VehSpdLimitTG_kph)  "<VTQD_VehSpdLimitTG_kph>"
  bus_selector16/13 -> outpmodule/758(VTQD_GearFlashInd_flg)  "<VTQD_GearFlashInd_flg>"
  bus_selector16/12 -> outpmodule/757(VTQD_GearFlashIndDis_flg)  "<VTQD_GearFlashIndDis_flg>"
  bus_selector16/8 -> outpmodule/753(VTQD_VCUEBSRd4BR_enum)  "<VTQD_VCUEBSRd4BR_enum>"
  bus_selector16/6 -> outpmodule/751(VTQD_VehAcclLimitTG_mps2)  "<VTQD_VehAcclLimitTG_mps2>"
  bus_selector16/3 -> outpmodule/748(VTQD_CreepIND_enum)  "<VTQD_CreepIND_enum>"
  bus_selector16/1 -> outpmodule/746(VTQD_VCUMCUCtrlMdTQD_enum)  "<VTQD_VCUMCUCtrlMdTQD_enum>"
  outpmodule/678(VOUTP_LRWheelTmpIndi_flg) -> bus_creator/678
  bus_selector16/59 -> outpmodule/804(VTQD_EC1EMSupTSC1CtrlPG1_cnt)  "<VTQD_EC1EMSupTSC1CtrlPG1_cnt>"
  outpmodule/605(VOUTP_HWVer1_cnt) -> bus_creator/605
  bus_selector16/9 -> outpmodule/754(VTQD_ParkingProtectWarning_flg)  "<VTQD_ParkingProtectWarning_flg>"
  bus_selector15/91 -> outpmodule/739(VTPM_FlashIDvalid_enum)  "<VTPM_FlashIDvalid_enum>"
  bus_selector16/43 -> outpmodule/788(VTQD_EC1PercTorqIdleP3_pct)  "<VTQD_EC1PercTorqIdleP3_pct>"
  bus_selector15/92 -> outpmodule/740(VTPM_WritingCnt_enum)  "<VTPM_WritingCnt_enum>"
  bus_selector15/90 -> outpmodule/738(VTPM_FlashS4ID_raw)  "<VTPM_FlashS4ID_raw>"
  bus_selector15/82 -> outpmodule/730(VTPM_Flashchkdatavalid_enum)  "<VTPM_Flashchkdatavalid_enum>"
  outpmodule/130(VOUTP_LongAccelVTimeOut_flg) -> bus_creator/130
  outpmodule/508(VOUTP_ParkingModeCmd_enum) -> bus_creator/508
  bus_selector15/84 -> outpmodule/732(VTPM_unlearnSfali_flg)  "<VTPM_unlearnSfali_flg>"
  outpmodule/535(VOUTP_ChrgFault_enum) -> bus_creator/535
  bus_selector15/79 -> outpmodule/727(VTPM_WriteChkfinRFID_raw)  "<VTPM_WriteChkfinRFID_raw>"
  outpmodule/56(VOUTP_ModOperation_enum) -> bus_creator/56
  outpmodule/705(VOUTP_S1WheelDebugALTU_pct) -> bus_creator/705
  bus_selector15/75 -> outpmodule/723(VTPM_WriteChkRFID_raw)  "<VTPM_WriteChkRFID_raw>"
  bus_selector15/77 -> outpmodule/725(VTPM_WriteChkRRID_raw)  "<VTPM_WriteChkRRID_raw>"
  bus_selector15/74 -> outpmodule/722(VTPM_WriteChkLFID_raw)  "<VTPM_WriteChkLFID_raw>"
  outpmodule/366(VOUTP_RFWheelTmpHighDTC_raw32) -> bus_creator/366
  bus_selector15/78 -> outpmodule/726(VTPM_WriteChkfinLFID_raw)  "<VTPM_WriteChkfinLFID_raw>"
  bus_selector15/71 -> outpmodule/719(VTPM_RFPind_enum)  "<VTPM_RFPind_enum>"
  bus_selector15/66 -> outpmodule/714(VTPM_SetIDLoc_flg)  "<VTPM_SetIDLoc_flg>"
  bus_selector16/41 -> outpmodule/786(VTQD_EC1PercTorqIdleP2_pct)  "<VTQD_EC1PercTorqIdleP2_pct>"
  bus_selector15/68 -> outpmodule/716(VTPM_ChkStorge_flg)  "<VTPM_ChkStorge_flg>"
  bus_selector15/67 -> outpmodule/715(VTPM_TPMSStorge_flg)  "<VTPM_TPMSStorge_flg>"
  outpmodule/434(VOUTP_TNECPSAL_kWh) -> bus_creator/434
  bus_selector15/63 -> outpmodule/711(VTPM_ID3messageALTU_raw8)  "<VTPM_ID3messageALTU_raw8>"
  bus_selector16/42 -> outpmodule/787(VTQD_EC1EMSpdIdleP3_rpm)  "<VTQD_EC1EMSpdIdleP3_rpm>"
  outpmodule/699(VOUTP_LFP20_raw8) -> bus_creator/699
  bus_selector15/59 -> outpmodule/707(VTPM_S3WheelDebugALTU_pct)  "<VTPM_S3WheelDebugALTU_pct>"
  bus_selector15/60 -> outpmodule/708(VTPM_S4WheelDebugALTU_pct)  "<VTPM_S4WheelDebugALTU_pct>"
  outpmodule/518(VOUTP_NMmTxReq_flg) -> bus_creator/518
  bus_selector15/55 -> outpmodule/703(VTPM_FAT_flg)  "<VTPM_FAT_flg>"
  outpmodule/805(VOUTP_EC1EMSupTSC1CtrlPG3_cnt) -> bus_creator/805
  bus_selector15/53 -> outpmodule/701(VTPM_LRP20_raw8)  "<VTPM_LRP20_raw8>"
  outpmodule/178(VOUTP_DKCPDkeyAreaRAPSSta_enum) -> bus_creator/178
  bus_selector15/50 -> outpmodule/698(VTPM_ALFin_flg)  "<VTPM_ALFin_flg>"
  bus_selector15/52 -> outpmodule/700(VTPM_RFP20_raw8)  "<VTPM_RFP20_raw8>"
  outpmodule/192(VOUTP_FDCBCMPLampCmd_flg) -> bus_creator/192
  bus_selector15/49 -> outpmodule/697(VTPM_S4L_enum)  "<VTPM_S4L_enum>"
  outpmodule/389(VOUTP_VCUFLDoorSta_flg) -> bus_creator/389
  bus_selector15/43 -> outpmodule/691(VTPM_S2ID_raw32)  "<VTPM_S2ID_raw32>"
  outpmodule/99(VOUTP_ShifterHandleCmd_enum) -> bus_creator/99
  bus_selector15/45 -> outpmodule/693(VTPM_S4ID_raw32)  "<VTPM_S4ID_raw32>"
  bus_selector16/63 -> outpmodule/808(VTQD_EC1EMSpdHdleP6_rpm)  "<VTQD_EC1EMSpdHdleP6_rpm>"
  bus_selector15/44 -> outpmodule/692(VTPM_S3ID_raw32)  "<VTPM_S3ID_raw32>"
  outpmodule/435(VOUTP_TEBPSAR_kWh) -> bus_creator/435
  bus_selector15/42 -> outpmodule/690(VTPM_S1ID_raw32)  "<VTPM_S1ID_raw32>"
  outpmodule/185(VOUTP_RAPSBCMLamp_enum) -> bus_creator/185
  bus_selector15/40 -> outpmodule/688(VTPM_LRSensorMode_flg)  "<VTPM_LRSensorMode_flg>"
  bus_selector15/38 -> outpmodule/686(VTPM_LFSensorMode_flg)  "<VTPM_LFSensorMode_flg>"
  bus_selector15/39 -> outpmodule/687(VTPM_RFSensorMode_flg)  "<VTPM_RFSensorMode_flg>"
  outpmodule/240(VOUTP_FDCBCMLTurnSWSta_flg) -> bus_creator/240
  bus_selector15/34 -> outpmodule/682(VTPM_RFWheelPSW_raw8)  "<VTPM_RFWheelPSW_raw8>"
  bus_selector15/29 -> outpmodule/677(VTPM_RFWheelTmpIndi_flg)  "<VTPM_RFWheelTmpIndi_flg>"
  outpmodule/763(VOUTP_VCUBCMBuzzReq_flg) -> bus_creator/763
  bus_selector15/30 -> outpmodule/678(VTPM_LRWheelTmpIndi_flg)  "<VTPM_LRWheelTmpIndi_flg>"
  outpmodule/689(VOUTP_RRSensorMode_flg) -> bus_creator/689
  BVMC_outputs/1 -> bus_selector19/1
  bus_selector15/25 -> outpmodule/673(VTPM_LRPressIndi_enum)  "<VTPM_LRPressIndi_enum>"
  bus_selector15/73 -> outpmodule/721(VTPM_RRPindi_enum)  "<VTPM_RRPindi_enum>"
  bus_selector15/24 -> outpmodule/672(VTPM_RFPressIndi_enum)  "<VTPM_RFPressIndi_enum>"
  bus_selector15/23 -> outpmodule/671(VTPM_LFPressIndi_enum)  "<VTPM_LFPressIndi_enum>"
  bus_selector15/21 -> outpmodule/669(VTPM_TPMSResButtAllow_flg)  "<VTPM_TPMSResButtAllow_flg>"
  outpmodule/23(VOUTP_PASDRCR_cm) -> bus_creator/23
  outpmodule/688(VOUTP_LRSensorMode_flg) -> bus_creator/688
  bus_selector15/19 -> outpmodule/667(VTPM_RFWheelDebug_flg)  "<VTPM_RFWheelDebug_flg>"
  bus_selector16/7 -> outpmodule/752(VTQD_VCUEBSHHSw_enum)  "<VTQD_VCUEBSHHSw_enum>"
  bus_selector15/15 -> outpmodule/663(VTPM_LRSensorFail_flg)  "<VTPM_LRSensorFail_flg>"
  bus_selector15/17 -> outpmodule/665(VTPM_LFWheelDebug_flg)  "<VTPM_LFWheelDebug_flg>"
  bus_selector15/16 -> outpmodule/664(VTPM_RRSensorFail_flg)  "<VTPM_RRSensorFail_flg>"
  outpmodule/8(VOUTP_CACFanReq_flg) -> bus_creator/8
  outpmodule/800(VOUTP_EC1EMExtRSCtrlUpLmt_rpm) -> bus_creator/800
  bus_selector15/13 -> outpmodule/661(VTPM_LFSensorFail_flg)  "<VTPM_LFSensorFail_flg>"
  outpmodule/261(VOUTP_C1ABM1LCDTC_raw32) -> bus_creator/261
  bus_selector15/12 -> outpmodule/660(VTPM_RRWheelTemp_C)  "<VTPM_RRWheelTemp_C>"
  bus_selector15/11 -> outpmodule/659(VTPM_LRWheelTemp_C)  "<VTPM_LRWheelTemp_C>"
  bus_selector15/9 -> outpmodule/657(VTPM_LFWheelTemp_C)  "<VTPM_LFWheelTemp_C>"
  outpmodule/915(VOUTP_LVDAFailinfo_flg) -> bus_creator/915
  bus_selector15/10 -> outpmodule/658(VTPM_RFWheelTemp_C)  "<VTPM_RFWheelTemp_C>"
  bus_selector16/4 -> outpmodule/749(VTQD_ActTUpAIND_enum)  "<VTQD_ActTUpAIND_enum>"
  outpmodule/577(VOUTP_V2BAux4RlyFit_enum) -> bus_creator/577
  bus_selector15/7 -> outpmodule/655(VTPM_LRWheelPress_raw8)  "<VTPM_LRWheelPress_raw8>"
  bus_selector15/2 -> outpmodule/650(VTPM_RFBatWarn_flg)  "<VTPM_RFBatWarn_flg>"
  outpmodule/398(VOUTP_EAPS2MIN_pct) -> bus_creator/398
  bus_selector15/1 -> outpmodule/649(VTPM_LFBatWarn_flg)  "<VTPM_LFBatWarn_flg>"
  outpmodule/449(VOUTP_CDEODTL_km) -> bus_creator/449
  outpmodule/15(VOUTP_EACSpdDemand_rpm) -> bus_creator/15
  bus_selector15/5 -> outpmodule/653(VTPM_LFWheelPress_raw8)  "<VTPM_LFWheelPress_raw8>"
  BTPM_outputs/1 -> bus_selector15/1
  bus_selector16/71 -> outpmodule/816(VTQD_RC1RetSpdP2_pct)  "<VTQD_RC1RetSpdP2_pct>"
  bus_selector15/94 -> outpmodule/742(VTPM_LProgress_enum)  "<VTPM_LProgress_enum>"
  outpmodule/866(VOUTP_FeatArbitrFinal_enum) -> bus_creator/866
  outpmodule/358(VOUTP_RFBatwarnDTC_raw32) -> bus_creator/358
  bus_selector15/93 -> outpmodule/741(VTPM_TPMSTLCmd_flg)  "<VTPM_TPMSTLCmd_flg>"
  bus_selector16/56 -> outpmodule/801(VTQD_EC1EMMomOfInertia_kgpm2)  "<VTQD_EC1EMMomOfInertia_kgpm2>"
  outpmodule/715(VOUTP_TPMSStorge_flg) -> bus_creator/715
  bus_selector15/95 -> outpmodule/743(VTPM_TPMSSensorIDRegStart_flg)  "<VTPM_TPMSSensorIDRegStart_flg>"
  outpmodule/144(VOUTP_EPBExtApplyAvailTimeOut_flg) -> bus_creator/144
  bus_selector15/97 -> outpmodule/745(VTPM_ModelVersionChksum_raw)  "<VTPM_ModelVersionChksum_raw>"
  bus_selector16/72 -> outpmodule/817(VTQD_RC1MaxRetSpdP3_rpm)  "<VTQD_RC1MaxRetSpdP3_rpm>"
  bus_selector15/62 -> outpmodule/710(VTPM_ID2messageALTU_raw8)  "<VTPM_ID2messageALTU_raw8>"
  bus_selector13/38 -> outpmodule/642(VSYS_ECUGen2_cnt)  "<VSYS_ECUGen2_cnt>"
  outpmodule/169(VOUTP_APSProgressPCT_pct) -> bus_creator/169
  outpmodule/11(VOUTP_EHPSEnTimeout_flg) -> bus_creator/11
  bus_selector13/36 -> outpmodule/640(VSYS_CurrentNmState_enum)  "<VSYS_CurrentNmState_enum>"
  outpmodule/935(VOUTP_APSDecReqA_flg) -> bus_creator/935
  bus_selector13/35 -> outpmodule/639(VSYS_AcoreRebootCmdACK_flg)  "<VSYS_AcoreRebootCmdACK_flg>"
  outpmodule/783(VOUTP_EC1EMSpdIdleP1_rpm) -> bus_creator/783
  bus_selector13/34 -> outpmodule/638(VSYS_WisrBootReason_raw32)  "<VSYS_WisrBootReason_raw32>"
  bus_selector13/32 -> outpmodule/636(VSYS_FdcSlpTime_sec)  "<VSYS_FdcSlpTime_sec>"
  bus_selector13/31 -> outpmodule/635(VSYS_FdcSlpReqRisingEdge_flg)  "<VSYS_FdcSlpReqRisingEdge_flg>"
  outpmodule/949(VOUTP_CalibratedGyroZ_Dps) -> bus_creator/949
  bus_selector13/28 -> outpmodule/632(VSYS_SHA7_cnt)  "<VSYS_SHA7_cnt>"
  bus_selector13/27 -> outpmodule/631(VSYS_SHA6_cnt)  "<VSYS_SHA6_cnt>"
  outpmodule/829(VOUTP_EMRC1RetSelNonEng_pct) -> bus_creator/829
  bus_selector13/25 -> outpmodule/629(VSYS_SHA4_cnt)  "<VSYS_SHA4_cnt>"
  bus_selector13/24 -> outpmodule/628(VSYS_SHA3_cnt)  "<VSYS_SHA3_cnt>"
  bus_selector13/23 -> outpmodule/627(VSYS_SHA2_cnt)  "<VSYS_SHA2_cnt>"
  bus_selector13/19 -> outpmodule/623(VSYS_Change1_cnt)  "<VSYS_Change1_cnt>"
  bus_selector13/22 -> outpmodule/626(VSYS_SHA1_cnt)  "<VSYS_SHA1_cnt>"
  bus_selector13/16 -> outpmodule/620(VSYS_Country2_cnt)  "<VSYS_Country2_cnt>"
  bus_selector13/14 -> outpmodule/618(VSYS_Patch2_cnt)  "<VSYS_Patch2_cnt>"
  outpmodule/672(VOUTP_RFPressIndi_enum) -> bus_creator/672
  bus_selector13/12 -> outpmodule/616(VSYS_Minor2_cnt)  "<VSYS_Minor2_cnt>"
  outpmodule/381(VOUTP_DisengagePFail_flg) -> bus_creator/381
  bus_selector13/10 -> outpmodule/614(VSYS_Major2_cnt)  "<VSYS_Major2_cnt>"
  bus_selector13/9 -> outpmodule/613(VSYS_Major1_cnt)  "<VSYS_Major1_cnt>"
  bus_selector13/5 -> outpmodule/609(VSYS_CarModel2_cnt)  "<VSYS_CarModel2_cnt>"
  bus_selector13/1 -> outpmodule/605(VSYS_HWVer1_cnt)  "<VSYS_HWVer1_cnt>"
  bus_selector13/4 -> outpmodule/608(VSYS_CarModel1_cnt)  "<VSYS_CarModel1_cnt>"
  bus_selector12/7 -> outpmodule/596(VSCP_triggerDT_flg)  "<VSCP_triggerDT_flg>"
  BPMM_outputs/1 -> bus_selector10/1
  bus_selector11/1 -> outpmodule/588(VPSA_Keystatus_enum)  "<VPSA_Keystatus_enum>"
  bus_selector10/56 -> outpmodule/584(VPMM_VSPTurnLeft_enum)  "<VPMM_VSPTurnLeft_enum>"
  bus_selector10/51 -> outpmodule/579(VPMM_VCULife2_cnt)  "<VPMM_VCULife2_cnt>"
  bus_selector10/49 -> outpmodule/577(VPMM_V2BAux4RlyFit_enum)  "<VPMM_V2BAux4RlyFit_enum>"
  outpmodule/223(VOUTP_InnerBuzzerModeSta_enum) -> bus_creator/223
  outpmodule/243(VOUTP_FDCBCMBrakeCmd_flg) -> bus_creator/243
  bus_selector10/50 -> outpmodule/578(VPMM_VCULife1_cnt)  "<VPMM_VCULife1_cnt>"
  bus_selector10/52 -> outpmodule/580(VPMM_VSPFunc_enum)  "<VPMM_VSPFunc_enum>"
  bus_selector10/47 -> outpmodule/575(VPMM_V2BAux3RlyFit_enum)  "<VPMM_V2BAux3RlyFit_enum>"
  outpmodule/401(VOUTP_EAPS2NRM_pct) -> bus_creator/401
  bus_selector10/48 -> outpmodule/576(VPMM_V2BAux4RlySta_enum)  "<VPMM_V2BAux4RlySta_enum>"
  outpmodule/222(VOUTP_FDCBCMEmExitSWSta_flg) -> bus_creator/222
  bus_selector16/24 -> outpmodule/769(VTQD_EVCU1EMotorPerformance_pct)  "<VTQD_EVCU1EMotorPerformance_pct>"
  bus_selector10/46 -> outpmodule/574(VPMM_V2BAux3RlySta_enum)  "<VPMM_V2BAux3RlySta_enum>"
  outpmodule/202(VOUTP_FDCBCMRTurnLpCmd_flg) -> bus_creator/202
  outpmodule/70(VOUTP_RFRawWhlSpeedVTimeOut_flg) -> bus_creator/70
  outpmodule/831(VOUTP_VCUMCUHandBrk_flg) -> bus_creator/831
  bus_selector10/45 -> outpmodule/573(VPMM_V2BAux2RlyFit_enum)  "<VPMM_V2BAux2RlyFit_enum>"
  bus_selector13/15 -> outpmodule/619(VSYS_Country1_cnt)  "<VSYS_Country1_cnt>"
  outpmodule/7(VOUTP_CACRunFail_flg) -> bus_creator/7
  bus_selector10/41 -> outpmodule/569(VPMM_V2BDCDCPosRlyFit_enum)  "<VPMM_V2BDCDCPosRlyFit_enum>"
  bus_selector10/36 -> outpmodule/564(VPMM_V2BAirPosRlySta_enum)  "<VPMM_V2BAirPosRlySta_enum>"
  bus_selector10/37 -> outpmodule/565(VPMM_V2BAirPosRlyFit_enum)  "<VPMM_V2BAirPosRlyFit_enum>"
  bus_selector10/35 -> outpmodule/563(VPMM_V2BACPosRlyFit_enum)  "<VPMM_V2BACPosRlyFit_enum>"
  outpmodule/807(VOUTP_EC1EMSupTSC1CtrlPG4_cnt) -> bus_creator/807
  bus_selector16/45 -> outpmodule/790(VTQD_EC1PercTorqIdleP4_pct)  "<VTQD_EC1PercTorqIdleP4_pct>"
  bus_selector10/31 -> outpmodule/559(VPMM_V2BAux3OnOff_enum)  "<VPMM_V2BAux3OnOff_enum>"
  bus_selector10/33 -> outpmodule/561(VPMM_V2BMainPosRlyFit_enum)  "<VPMM_V2BMainPosRlyFit_enum>"
  bus_selector15/58 -> outpmodule/706(VTPM_S2WheelDebugALTU_pct)  "<VTPM_S2WheelDebugALTU_pct>"
  bus_selector10/30 -> outpmodule/558(VPMM_V2BAux2OnOff_enum)  "<VPMM_V2BAux2OnOff_enum>"
  bus_selector15/65 -> outpmodule/713(VTPM_Chkfin_flg)  "<VTPM_Chkfin_flg>"
  bus_selector10/29 -> outpmodule/557(VPMM_V2BAux1OnOff_enum)  "<VPMM_V2BAux1OnOff_enum>"
  outpmodule/810(VOUTP_RC1RetType_enum) -> bus_creator/810
  bus_selector16/36 -> outpmodule/781(VTQD_EMRC1ActEMpTrqHrls_pct)  "<VTQD_EMRC1ActEMpTrqHrls_pct>"
  outpmodule/74(VOUTP_RRRawWhlSpeedVTimeOut_flg) -> bus_creator/74
  bus_selector16/14 -> outpmodule/759(VTQD_SpdLimSta_flg)  "<VTQD_SpdLimSta_flg>"
  bus_selector10/28 -> outpmodule/556(VPMM_V2BLifeSig_cnt)  "<VPMM_V2BLifeSig_cnt>"
  outpmodule/592(VOUTP_CFGEM1BAMTSize_raw) -> bus_creator/592
  bus_selector15/33 -> outpmodule/681(VTPM_LRWheelPSW_raw8)  "<VTPM_LRWheelPSW_raw8>"
  bus_selector10/26 -> outpmodule/554(VPMM_HVFailureChkPass_flg)  "<VPMM_HVFailureChkPass_flg>"
  bus_selector10/23 -> outpmodule/551(VPMM_LVBattLowInd_enum)  "<VPMM_LVBattLowInd_enum>"
  bus_selector10/21 -> outpmodule/549(VPMM_HVILFail_flg)  "<VPMM_HVILFail_flg>"
  outpmodule/386(VOUTP_HVRlyOpFail_flg) -> bus_creator/386
  outpmodule/764(VOUTP_VCUEBSHBSw_enum) -> bus_creator/764
  bus_selector10/19 -> outpmodule/547(VPMM_VCUMCUEn_flg)  "<VPMM_VCUMCUEn_flg>"
  outpmodule/884(VOUTP_ACCJerkLowerLimit_mps3) -> bus_creator/884
  bus_selector10/18 -> outpmodule/546(VPMM_ActiveDischargeReq_enum)  "<VPMM_ActiveDischargeReq_enum>"
  bus_selector16/44 -> outpmodule/789(VTQD_EC1EMSpdIdleP4_rpm)  "<VTQD_EC1EMSpdIdleP4_rpm>"
  bus_selector10/15 -> outpmodule/543(VPMM_ACHVLoopDem_enum)  "<VPMM_ACHVLoopDem_enum>"
  bus_selector10/14 -> outpmodule/542(VPMM_EHPSRlyDem_enum)  "<VPMM_EHPSRlyDem_enum>"
  bus_selector10/17 -> outpmodule/545(VPMM_DrivelineRelease_enum)  "<VPMM_DrivelineRelease_enum>"
  bus_selector16/23 -> outpmodule/768(VTQD_EVCU1EMotorOvrerSpd_enum)  "<VTQD_EVCU1EMotorOvrerSpd_enum>"
  bus_selector10/11 -> outpmodule/539(VPMM_DCDCRlyDem_enum)  "<VPMM_DCDCRlyDem_enum>"
  bus_selector16/25 -> outpmodule/770(VTQD_EVCU1EBrakeTorqLow_enum)  "<VTQD_EVCU1EBrakeTorqLow_enum>"
  bus_selector10/13 -> outpmodule/541(VPMM_MCUHVLoopDem_enum)  "<VPMM_MCUHVLoopDem_enum>"
  bus_selector10/12 -> outpmodule/540(VPMM_CACRlyDem_enum)  "<VPMM_CACRlyDem_enum>"
  bus_selector10/9 -> outpmodule/537(VPMM_IGNRlyClose_flg)  "<VPMM_IGNRlyClose_flg>"
  bus_selector10/10 -> outpmodule/538(VPMM_BattHVDem_enum)  "<VPMM_BattHVDem_enum>"
  bus_selector11/2 -> outpmodule/589(VPSA_EmergencyShutDown_flg)  "<VPSA_EmergencyShutDown_flg>"
  bus_selector10/8 -> outpmodule/536(VPMM_IRCRlyClose_flg)  "<VPMM_IRCRlyClose_flg>"
  bus_selector10/6 -> outpmodule/534(VPMM_PowerDownFault_enum)  "<VPMM_PowerDownFault_enum>"
  outpmodule/162(VOUTP_IVIScreenTimeOut_flg) -> bus_creator/162
  bus_selector15/4 -> outpmodule/652(VTPM_RRBatWarn_flg)  "<VTPM_RRBatWarn_flg>"
  bus_selector10/7 -> outpmodule/535(VPMM_ChrgFault_enum)  "<VPMM_ChrgFault_enum>"
  bus_selector10/2 -> outpmodule/530(VPMM_PowerUpState_enum)  "<VPMM_PowerUpState_enum>"
  outpmodule/817(VOUTP_RC1MaxRetSpdP3_rpm) -> bus_creator/817
  bus_selector10/4 -> outpmodule/532(VPMM_ChrgState_enum)  "<VPMM_ChrgState_enum>"
  outpmodule/146(VOUTP_EPBErrStaTimeOut_flg) -> bus_creator/146
  bus_selector10/1 -> outpmodule/529(VPMM_SysPowerMode_enum)  "<VPMM_SysPowerMode_enum>"
  bus_selector10/3 -> outpmodule/531(VPMM_PowerDownState_enum)  "<VPMM_PowerDownState_enum>"
  outpmodule/855(VOUTP_RearWhlSlipRatioCtrl_flg) -> bus_creator/855
  bus_selector12/11 -> outpmodule/600(VSCP_DTbyte3_raw)  "<VSCP_DTbyte3_raw>"
  outpmodule/729(VOUTP_WriteChkfinRRID_raw) -> bus_creator/729
  bus_selector12/12 -> outpmodule/601(VSCP_DTbyte4_raw)  "<VSCP_DTbyte4_raw>"
  outpmodule/702(VOUTP_RRP20_raw8) -> bus_creator/702
  bus_selector15/28 -> outpmodule/676(VTPM_LFWheelTmpIndi_flg)  "<VTPM_LFWheelTmpIndi_flg>"
  BNMM_outputs/1 -> bus_selector9/1
  outpmodule/14(VOUTP_EHPSSpdCtrlMode_enum) -> bus_creator/14
  bus_selector15/48 -> outpmodule/696(VTPM_S3L_enum)  "<VTPM_S3L_enum>"
  BSCP_outputs/1 -> bus_selector12/1
  bus_selector9/9 -> outpmodule/525(VNMM_WakeUp_enum)  "<VNMM_WakeUp_enum>"
  bus_selector16/70 -> outpmodule/815(VTQD_RC1MaxRetSpdP2_rpm)  "<VTQD_RC1MaxRetSpdP2_rpm>"
  bus_selector9/8 -> outpmodule/524(VNMM_RptMsgReq_flg)  "<VNMM_RptMsgReq_flg>"
  bus_selector17/2 -> outpmodule/834(VTQR_RrTMTqReq_Nm)  "<VTQR_RrTMTqReq_Nm>"
  bus_selector9/7 -> outpmodule/523(VNMM_PNI_flg)  "<VNMM_PNI_flg>"
  bus_selector9/2 -> outpmodule/518(VNMM_NMmTxReq_flg)  "<VNMM_NMmTxReq_flg>"
  bus_selector19/12 -> outpmodule/853(VVMC_LimitPCT_pct)  "<VVMC_LimitPCT_pct>"
  bus_selector9/3 -> outpmodule/519(VNMM_Awake_enum)  "<VNMM_Awake_enum>"
  outpmodule/368(VOUTP_RRWheelTmpHighDTC_raw32) -> bus_creator/368
  bus_selector7/11 -> outpmodule/504(VDKC_KeyAreaPTG_enum)  "<VDKC_KeyAreaPTG_enum>"
  outpmodule/753(VOUTP_VCUEBSRd4BR_enum) -> bus_creator/753
  bus_selector7/10 -> outpmodule/503(VDKC_DKeyWelcomeSta_enum)  "<VDKC_DKeyWelcomeSta_enum>"
  bus_selector12/4 -> outpmodule/593(VSCP_CFGEM1BAMTNum_raw)  "<VSCP_CFGEM1BAMTNum_raw>"
  bus_selector7/8 -> outpmodule/501(VDKC_KeyAreaLockUnlock_enum)  "<VDKC_KeyAreaLockUnlock_enum>"
  outpmodule/827(VOUTP_EVCU1RecuperHighSta_enum) -> bus_creator/827
  bus_selector7/7 -> outpmodule/500(VDKC_KeyAreaPS_enum)  "<VDKC_KeyAreaPS_enum>"
  bus_selector7/6 -> outpmodule/499(VDKC_DkeyShowIVISta_enum)  "<VDKC_DkeyShowIVISta_enum>"
  outpmodule/485(VOUTP_OFFR_sec) -> bus_creator/485
  bus_selector7/5 -> outpmodule/498(VDKC_KeyModeSta_enum)  "<VDKC_KeyModeSta_enum>"
  bus_selector10/53 -> outpmodule/581(VPMM_VSPIGNKeySta_enum)  "<VPMM_VSPIGNKeySta_enum>"
  bus_selector7/4 -> outpmodule/497(VDKC_KeyMissSta_flg)  "<VDKC_KeyMissSta_flg>"
  bus_selector7/2 -> outpmodule/495(VDKC_DKCAuthSta_enum)  "<VDKC_DKCAuthSta_enum>"
  outpmodule/607(VOUTP_HWVer3_cnt) -> bus_creator/607
  bus_selector7/1 -> outpmodule/494(VDKC_DKCTimeSN_cnt)  "<VDKC_DKCTimeSN_cnt>"
  bus_selector7/3 -> outpmodule/496(VDKC_TimeSNDKCFbk_cnt)  "<VDKC_TimeSNDKCFbk_cnt>"
  bus_selector6/91 -> outpmodule/492(VDID_DIDModelVersion_raw)  "<VDID_DIDModelVersion_raw>"
  bus_selector6/90 -> outpmodule/491(VDID_HVBATT_A)  "<VDID_HVBATT_A>"
  BPSA_outputs/1 -> bus_selector11/1
  bus_selector6/89 -> outpmodule/490(VDID_HEVMODE_enum)  "<VDID_HEVMODE_enum>"
  outpmodule/13(VOUTP_DCDCEnDemamd_enum) -> bus_creator/13
  outpmodule/572(VOUTP_V2BAux2RlySta_enum) -> bus_creator/572
  bus_selector6/86 -> outpmodule/487(VDID_AVGBATTEMPL_sec)  "<VDID_AVGBATTEMPL_sec>"
  outpmodule/594(VOUTP_CFGEM1BAMRsv_raw) -> bus_creator/594
  bus_selector6/82 -> outpmodule/483(VDID_OVCR_sec)  "<VDID_OVCR_sec>"
  outpmodule/357(VOUTP_LFBatwarnDTC_raw32) -> bus_creator/357
  bus_selector6/81 -> outpmodule/482(VDID_BattTempPSAL_sec)  "<VDID_BattTempPSAL_sec>"
  bus_selector15/61 -> outpmodule/709(VTPM_ID1messageALTU_raw8)  "<VTPM_ID1messageALTU_raw8>"
  bus_selector6/79 -> outpmodule/480(VDID_PKELNumerator_kphsqr)  "<VDID_PKELNumerator_kphsqr>"
  bus_selector6/76 -> outpmodule/477(VDID_CALID_cnt)  "<VDID_CALID_cnt>"
  bus_selector6/74 -> outpmodule/475(VDID_RESSTIMESOCRNGAXIS_enum)  "<VDID_RESSTIMESOCRNGAXIS_enum>"
  bus_selector6/73 -> outpmodule/474(VDID_RESSTTEMPRNGAXIS_enum)  "<VDID_RESSTTEMPRNGAXIS_enum>"
  outpmodule/627(VOUTP_SHA2_cnt) -> bus_creator/627
  bus_selector19/18 -> outpmodule/859(VVMC_SPD2ACCAct_flg)  "<VVMC_SPD2ACCAct_flg>"
  bus_selector6/70 -> outpmodule/471(VDID_MINBATTEMPL_C)  "<VDID_MINBATTEMPL_C>"
  bus_selector6/69 -> outpmodule/470(VDID_MAXBATTEMPL_C)  "<VDID_MAXBATTEMPL_C>"
  outpmodule/220(VOUTP_FDCBCMRBSDRCmd_flg) -> bus_creator/220
  bus_selector6/66 -> outpmodule/467(VDID_RESSTIMESOCCHGRNGL_s)  "<VDID_RESSTIMESOCCHGRNGL_s>"
  outpmodule/476(VOUTP_RESSCNTSDODRNGAXIS_enum) -> bus_creator/476
  bus_selector6/68 -> outpmodule/469(VDID_RESSTIMESOCOFFRNGL_s)  "<VDID_RESSTIMESOCOFFRNGL_s>"
  bus_selector6/67 -> outpmodule/468(VDID_RESSTIMESOCOFFRNGR_s)  "<VDID_RESSTIMESOCOFFRNGR_s>"
  bus_selector6/62 -> outpmodule/463(VDID_ETMBTOEL_kWh)  "<VDID_ETMBTOEL_kWh>"
  outpmodule/839(VOUTP_ReqOBCIntrV2LEna_enum) -> bus_creator/839
  bus_selector6/64 -> outpmodule/465(VDID_RESSTIMESOCPSARNGL_s)  "<VDID_RESSTIMESOCPSARNGL_s>"
  outpmodule/832(VOUTP_VCUMCUFootBrk_flg) -> bus_creator/832
  bus_selector16/18 -> outpmodule/763(VTQD_VCUBCMBuzzReq_flg)  "<VTQD_VCUBCMBuzzReq_flg>"
  bus_selector6/61 -> outpmodule/462(VDID_ETMBTOER_kWh)  "<VDID_ETMBTOER_kWh>"
  bus_selector6/59 -> outpmodule/460(VDID_ETMATOER_kWh)  "<VDID_ETMATOER_kWh>"
  outpmodule/554(VOUTP_HVFailureChkPass_flg) -> bus_creator/554
  bus_selector6/57 -> outpmodule/458(VDID_RESSCNTDODRNGR_cnt)  "<VDID_RESSCNTDODRNGR_cnt>"
  bus_selector6/54 -> outpmodule/455(VDID_AvgBattTempOFFL_C)  "<VDID_AvgBattTempOFFL_C>"
  bus_selector6/50 -> outpmodule/451(VDID_AvgBattTempPSAL_C)  "<VDID_AvgBattTempPSAL_C>"
  bus_selector6/49 -> outpmodule/450(VDID_AvgBattTempPSAR_C)  "<VDID_AvgBattTempPSAR_C>"
  outpmodule/184(VOUTP_APSVMCReqA_flg) -> bus_creator/184
  outpmodule/491(VOUTP_HVBATT_A) -> bus_creator/491
  bus_selector16/11 -> outpmodule/756(VTQD_VCU4PweLmtInd_flg)  "<VTQD_VCU4PweLmtInd_flg>"
  bus_selector16/50 -> outpmodule/795(VTQD_EC1EMMaxMOvrTmt_s)  "<VTQD_EC1EMMaxMOvrTmt_s>"
  bus_selector6/47 -> outpmodule/448(VDID_CDEODTR_km)  "<VDID_CDEODTR_km>"
  bus_selector6/48 -> outpmodule/449(VDID_CDEODTL_km)  "<VDID_CDEODTL_km>"
  outpmodule/598(VOUTP_DTbyte1_raw) -> bus_creator/598
  bus_selector6/43 -> outpmodule/444(VDID_RESSV2XENNONPSAL_kWh)  "<VDID_RESSV2XENNONPSAL_kWh>"
  outpmodule/567(VOUTP_V2BOilPosRlyFit_enum) -> bus_creator/567
  bus_selector6/44 -> outpmodule/445(VDID_PKER_kphsqr)  "<VDID_PKER_kphsqr>"
  bus_selector6/45 -> outpmodule/446(VDID_PKEL_kphsqr)  "<VDID_PKEL_kphsqr>"
  bus_selector6/41 -> outpmodule/442(VDID_GECHGOVCACL_kWh)  "<VDID_GECHGOVCACL_kWh>"
  bus_selector12/15 -> outpmodule/604(VSCP_DTbyte7_raw)  "<VSCP_DTbyte7_raw>"
  bus_selector6/40 -> outpmodule/441(VDID_GECHGOVCACR_kWh)  "<VDID_GECHGOVCACR_kWh>"
  bus_selector13/11 -> outpmodule/615(VSYS_Minor1_cnt)  "<VSYS_Minor1_cnt>"
  outpmodule/233(VOUTP_FDCBCMHelpINDCmd_flg) -> bus_creator/233
  bus_selector6/38 -> outpmodule/439(VDID_GECHGOVCDCR_kWh)  "<VDID_GECHGOVCDCR_kWh>"
  bus_selector15/76 -> outpmodule/724(VTPM_WriteChkLRID_raw)  "<VTPM_WriteChkLRID_raw>"
  bus_selector6/77 -> outpmodule/478(VDID_ECUNAME_cnt)  "<VDID_ECUNAME_cnt>"
  outpmodule/495(VOUTP_DKCAuthSta_enum) -> bus_creator/495
  bus_selector6/36 -> outpmodule/437(VDID_TGEOVCR_kWh)  "<VDID_TGEOVCR_kWh>"
  bus_selector6/34 -> outpmodule/435(VDID_TEBPSAR_kWh)  "<VDID_TEBPSAR_kWh>"
  bus_selector6/32 -> outpmodule/433(VDID_TNECPSAR_kWh)  "<VDID_TNECPSAR_kWh>"
  bus_selector15/87 -> outpmodule/735(VTPM_FlashS1ID_raw)  "<VTPM_FlashS1ID_raw>"
  bus_selector6/31 -> outpmodule/432(VDID_TNBCPSAL_Ahr)  "<VDID_TNBCPSAL_Ahr>"
  outpmodule/87(VOUTP_LRPulseCountV_flg) -> bus_creator/87
  outpmodule/342(VOUTP_ISAMalfuncDetDTC_raw32) -> bus_creator/342
  bus_selector16/2 -> outpmodule/747(VTQD_CreepSpdReq_rpm)  "<VTQD_CreepSpdReq_rpm>"
  bus_selector8/1 -> outpmodule/513(VDSC_DISCTurn_flg)  "<VDSC_DISCTurn_flg>"
  bus_selector16/5 -> outpmodule/750(VTQD_VCUMCUDemHiPosVal_rpm)  "<VTQD_VCUMCUDemHiPosVal_rpm>"
  bus_selector7/17 -> outpmodule/510(VDKC_KeyTypeSta_enum)  "<VDKC_KeyTypeSta_enum>"
  outpmodule/766(VOUTP_EVCU1WheelSlipdet_enum) -> bus_creator/766
  bus_selector7/15 -> outpmodule/508(VDKC_ParkingModeCmd_enum)  "<VDKC_ParkingModeCmd_enum>"
  bus_selector7/16 -> outpmodule/509(VDKC_KeyNumSta_enum)  "<VDKC_KeyNumSta_enum>"
  bus_selector7/14 -> outpmodule/507(VDKC_DkeyAreaRAPSSta_enum)  "<VDKC_DkeyAreaRAPSSta_enum>"
  bus_selector15/86 -> outpmodule/734(VTPM_Prepresstempvalid_enum)  "<VTPM_Prepresstempvalid_enum>"
  bus_selector7/12 -> outpmodule/505(VDKC_KeyAreaSPTGSta_enum)  "<VDKC_KeyAreaSPTGSta_enum>"
  bus_selector6/26 -> outpmodule/427(VDID_CPSAL_sec)  "<VDID_CPSAL_sec>"
  outpmodule/730(VOUTP_Flashchkdatavalid_enum) -> bus_creator/730
  bus_selector6/24 -> outpmodule/425(VDID_IPSAL_sec)  "<VDID_IPSAL_sec>"
  outpmodule/307(VOUTP_DiagFRTSDTC_raw32) -> bus_creator/307
  outpmodule/930(VOUTP_CCCtrlSta_enum) -> bus_creator/930
  BDID_outputs/1 -> bus_selector6/1
  outpmodule/675(VOUTP_TPMSWarnIndi_enum) -> bus_creator/675
  bus_selector6/20 -> outpmodule/421(VDID_HVBattCurr_Ahps)  "<VDID_HVBattCurr_Ahps>"
  bus_selector6/19 -> outpmodule/420(VDID_NUMPSATRIPSFLTMEMCLR_cnt)  "<VDID_NUMPSATRIPSFLTMEMCLR_cnt>"
  bus_selector6/17 -> outpmodule/418(VDID_HVESSCHARGEACT_kW)  "<VDID_HVESSCHARGEACT_kW>"
  outpmodule/635(VOUTP_FdcSlpReqRisingEdge_flg) -> bus_creator/635
  bus_selector6/15 -> outpmodule/416(VDID_HVBCellVoltMax_V)  "<VDID_HVBCellVoltMax_V>"
  bus_selector6/13 -> outpmodule/414(VDID_BATSOH_pct)  "<VDID_BATSOH_pct>"
  bus_selector6/65 -> outpmodule/466(VDID_RESSTIMESOCCHGRNGR_s)  "<VDID_RESSTIMESOCCHGRNGR_s>"
  bus_selector10/59 -> outpmodule/587(VPMM_DCVol_V)  "<VPMM_DCVol_V>"
  BDHP_outputs/1 -> bus_selector5/1
  outpmodule/566(VOUTP_V2BOilPosRlySta_enum) -> bus_creator/566
  bus_selector5/6 -> outpmodule/401(VDHP_EAPS2NRM_pct)  "<VDHP_EAPS2NRM_pct>"
  outpmodule/209(VOUTP_FDCBCMWiperLCmd_flg) -> bus_creator/209
  outpmodule/896(VOUTP_ACCObjDstLvl_enum) -> bus_creator/896
  bus_selector5/1 -> outpmodule/396(VDHP_ActAPSPosn_pct)  "<VDHP_ActAPSPosn_pct>"
  bus_selector6/58 -> outpmodule/459(VDID_RESSCNTDODRNGL_cnt)  "<VDID_RESSCNTDODRNGL_cnt>"
  outpmodule/860(VOUTP_AccCalcuPID_mps2) -> bus_creator/860
  bus_selector5/4 -> outpmodule/399(VDHP_ResetPedalZeroPosStart_flg)  "<VDHP_ResetPedalZeroPosStart_flg>"
  bus_selector5/3 -> outpmodule/398(VDHP_EAPS2MIN_pct)  "<VDHP_EAPS2MIN_pct>"
  outpmodule/740(VOUTP_WritingCnt_enum) -> bus_creator/740
  bus_selector15/46 -> outpmodule/694(VTPM_S1L_enum)  "<VTPM_S1L_enum>"
  bus_selector5/5 -> outpmodule/400(VDHP_EAPS1NRM_pct)  "<VDHP_EAPS1NRM_pct>"
  bus_selector5/2 -> outpmodule/397(VDHP_EAPS1MIN_pct)  "<VDHP_EAPS1MIN_pct>"
  outpmodule/516(VOUTP_DISCButtSta_flg) -> bus_creator/516
  outpmodule/612(VOUTP_ECU2_cnt) -> bus_creator/612
  BDDM_outputs/1 -> bus_selector4/1
  bus_selector15/32 -> outpmodule/680(VTPM_LFWheelPSW_raw8)  "<VTPM_LFWheelPSW_raw8>"
  outpmodule/10(VOUTP_EHPSSpdDemTimeout_flg) -> bus_creator/10
  bus_selector4/149 -> outpmodule/395(VDDM_VCUTailgateSWSta_flg)  "<VDDM_VCUTailgateSWSta_flg>"
  outpmodule/547(VOUTP_VCUMCUEn_flg) -> bus_creator/547
  bus_selector4/147 -> outpmodule/393(VDDM_SysAllowReadySta_flg)  "<VDDM_SysAllowReadySta_flg>"
  bus_selector4/142 -> outpmodule/388(VDDM_VCUBrkSWSta_enum)  "<VDDM_VCUBrkSWSta_enum>"
  outpmodule/710(VOUTP_ID2messageALTU_raw8) -> bus_creator/710
  bus_selector4/146 -> outpmodule/392(VDDM_VCURRDoorSta_flg)  "<VDDM_VCURRDoorSta_flg>"
  bus_selector8/3 -> outpmodule/515(VDSC_DISCSta_enum)  "<VDSC_DISCSta_enum>"
  bus_selector4/144 -> outpmodule/390(VDDM_VCUFRDoorSta_flg)  "<VDDM_VCUFRDoorSta_flg>"
  bus_selector4/145 -> outpmodule/391(VDDM_VCURLDoorSta_flg)  "<VDDM_VCURLDoorSta_flg>"
  bus_selector15/8 -> outpmodule/656(VTPM_RRWheelPress_raw8)  "<VTPM_RRWheelPress_raw8>"
  bus_selector4/143 -> outpmodule/389(VDDM_VCUFLDoorSta_flg)  "<VDDM_VCUFLDoorSta_flg>"
  outpmodule/868(VOUTP_LateralCtrl_flg) -> bus_creator/868
  outpmodule/494(VOUTP_DKCTimeSN_cnt) -> bus_creator/494
  bus_selector19/115 -> outpmodule/956(VVMC_FDCVMCDrInpTqBstGn_pct)  "<VVMC_FDCVMCDrInpTqBstGn_pct>"
  bus_selector19/111 -> outpmodule/952(VVMC_FDCVMCAPSRqEPSCtrl_flg)  "<VVMC_FDCVMCAPSRqEPSCtrl_flg>"
  bus_selector19/113 -> outpmodule/954(VVMC_FDCVMCDrInpTqBstAct_flg)  "<VVMC_FDCVMCDrInpTqBstAct_flg>"
  bus_selector19/110 -> outpmodule/951(VVMC_FDCVMCAPSAngleTarget_deg)  "<VVMC_FDCVMCAPSAngleTarget_deg>"
  bus_selector19/112 -> outpmodule/953(VVMC_FDCVMCAngCtrlTqWtGn_pct)  "<VVMC_FDCVMCAngCtrlTqWtGn_pct>"
  outpmodule/503(VOUTP_DKeyWelcomeSta_enum) -> bus_creator/503
  outpmodule/539(VOUTP_DCDCRlyDem_enum) -> bus_creator/539
  bus_selector19/108 -> outpmodule/949(VVMC_CalibratedGyroZ_Dps)  "<VVMC_CalibratedGyroZ_Dps>"
  outpmodule/801(VOUTP_EC1EMMomOfInertia_kgpm2) -> bus_creator/801
  bus_selector19/107 -> outpmodule/948(VVMC_CalibratedGyroY_Dps)  "<VVMC_CalibratedGyroY_Dps>"
  bus_selector15/35 -> outpmodule/683(VTPM_RRWheelPSW_raw8)  "<VTPM_RRWheelPSW_raw8>"
  bus_selector16/10 -> outpmodule/755(VTQD_ActDriveMode_enum)  "<VTQD_ActDriveMode_enum>"
  bus_selector19/105 -> outpmodule/946(VVMC_CalibratedAccZ_G)  "<VVMC_CalibratedAccZ_G>"
  outpmodule/613(VOUTP_Major1_cnt) -> bus_creator/613
  bus_selector19/106 -> outpmodule/947(VVMC_CalibratedGyroX_Dps)  "<VVMC_CalibratedGyroX_Dps>"
  bus_selector19/102 -> outpmodule/943(VVMC_ExtraMSACtrlSta_enum)  "<VVMC_ExtraMSACtrlSta_enum>"
  bus_selector19/104 -> outpmodule/945(VVMC_CalibratedAccY_G)  "<VVMC_CalibratedAccY_G>"
  bus_selector19/100 -> outpmodule/941(VVMC_CAASCtrlAvail_flg)  "<VVMC_CAASCtrlAvail_flg>"
  bus_selector19/99 -> outpmodule/940(VVMC_IMUEnaCmd_flg)  "<VVMC_IMUEnaCmd_flg>"
  bus_selector19/95 -> outpmodule/936(VVMC_APSDecReq_mps2)  "<VVMC_APSDecReq_mps2>"
  bus_selector12/2 -> outpmodule/591(VSCP_CFGEM1Ctrl_raw)  "<VSCP_CFGEM1Ctrl_raw>"
  bus_selector19/94 -> outpmodule/935(VVMC_APSDecReqA_flg)  "<VVMC_APSDecReqA_flg>"
  bus_selector19/93 -> outpmodule/934(VVMC_APSStaSys_enum)  "<VVMC_APSStaSys_enum>"
  outpmodule/793(VOUTP_EC1EMRefTorq_Nm) -> bus_creator/793
  bus_selector19/92 -> outpmodule/933(VVMC_APSActive_flg)  "<VVMC_APSActive_flg>"
  bus_selector19/89 -> outpmodule/930(VVMC_CCCtrlSta_enum)  "<VVMC_CCCtrlSta_enum>"
  bus_selector19/90 -> outpmodule/931(VVMC_MSACtrlSta_enum)  "<VVMC_MSACtrlSta_enum>"
  outpmodule/646(VOUTP_EWPPEReq_rpm) -> bus_creator/646
  bus_selector19/87 -> outpmodule/928(VVMC_ACCPedalOvrd_flg)  "<VVMC_ACCPedalOvrd_flg>"
  outpmodule/213(VOUTP_TurnLpPatternSta_enum) -> bus_creator/213
  outpmodule/312(VOUTP_FMRUSSDTC_raw32) -> bus_creator/312
  bus_selector19/86 -> outpmodule/927(VVMC_ACCCtrlAvail_flg)  "<VVMC_ACCCtrlAvail_flg>"
  outpmodule/885(VOUTP_ACCComfortBandLower_mps2) -> bus_creator/885
  bus_selector19/88 -> outpmodule/929(VVMC_TimeGapCalcu_s)  "<VVMC_TimeGapCalcu_s>"
  outpmodule/327(VOUTP_FCM3CSErrDTC_raw32) -> bus_creator/327
  bus_selector19/84 -> outpmodule/925(VVMC_FCMLDWRequest_enum)  "<VVMC_FCMLDWRequest_enum>"
  bus_selector19/82 -> outpmodule/923(VVMC_ADASLanecurveR_raw32)  "<VVMC_ADASLanecurveR_raw32>"
  outpmodule/574(VOUTP_V2BAux3RlySta_enum) -> bus_creator/574
  bus_selector19/83 -> outpmodule/924(VVMC_ADASAEBSta_enum)  "<VVMC_ADASAEBSta_enum>"
  bus_selector19/80 -> outpmodule/921(VVMC_ADASLanetypeL_enum)  "<VVMC_ADASLanetypeL_enum>"
  bus_selector19/77 -> outpmodule/918(VVMC_ADASLFCWarnSound_enum)  "<VVMC_ADASLFCWarnSound_enum>"
  bus_selector16/87 -> outpmodule/832(VTQD_VCUMCUFootBrk_flg)  "<VTQD_VCUMCUFootBrk_flg>"
  bus_selector19/73 -> outpmodule/914(VVMC_LVDAMuteSta_enum)  "<VVMC_LVDAMuteSta_enum>"
  outpmodule/330(VOUTP_FCM5NoComDTC_raw32) -> bus_creator/330
  bus_selector19/75 -> outpmodule/916(VVMC_LVDAWarning_flg)  "<VVMC_LVDAWarning_flg>"
  bus_selector7/13 -> outpmodule/506(VDKC_UIDLowPowerSta_enum)  "<VDKC_UIDLowPowerSta_enum>"
  bus_selector19/71 -> outpmodule/912(VVMC_ADASLFCHandsOffWarning_enum)  "<VVMC_ADASLFCHandsOffWarning_enum>"
  outpmodule/176(VOUTP_APSRqEPASCtrl_flg) -> bus_creator/176
  outpmodule/791(VOUTP_EC1PercTorqIdleP5_pct) -> bus_creator/791
  bus_selector19/67 -> outpmodule/908(VVMC_ADASSLIFSta_enum)  "<VVMC_ADASSLIFSta_enum>"
  bus_selector19/65 -> outpmodule/906(VVMC_ADASLaneModeL_enum)  "<VVMC_ADASLaneModeL_enum>"
  bus_selector6/55 -> outpmodule/456(VDID_QTYPSATRIPSR_cnt)  "<VDID_QTYPSATRIPSR_cnt>"
  outpmodule/750(VOUTP_VCUMCUDemHiPosVal_rpm) -> bus_creator/750
  bus_selector10/25 -> outpmodule/553(VPMM_ChrgBCUHVFail_flg)  "<VPMM_ChrgBCUHVFail_flg>"
  bus_selector19/64 -> outpmodule/905(VVMC_ADASLFCSta_enum)  "<VVMC_ADASLFCSta_enum>"
  bus_selector10/39 -> outpmodule/567(VPMM_V2BOilPosRlyFit_enum)  "<VPMM_V2BOilPosRlyFit_enum>"
  bus_selector19/60 -> outpmodule/901(VVMC_TargetType_enum)  "<VVMC_TargetType_enum>"
  outpmodule/657(VOUTP_LFWheelTemp_C) -> bus_creator/657
  bus_selector13/13 -> outpmodule/617(VSYS_Patch1_cnt)  "<VSYS_Patch1_cnt>"
  bus_selector19/61 -> outpmodule/902(VVMC_ADASSLIFSpdLim_enum)  "<VVMC_ADASSLIFSpdLim_enum>"
  outpmodule/778(VOUTP_EMRC1EMTquModeDrvBrk_enum) -> bus_creator/778
  bus_selector19/69 -> outpmodule/910(VVMC_ADASLDWMute_flg)  "<VVMC_ADASLDWMute_flg>"
  bus_selector19/58 -> outpmodule/899(VVMC_ADASWarningMsg_enum)  "<VVMC_ADASWarningMsg_enum>"
  outpmodule/771(VOUTP_EVCU2MaxTorqAvail_pct) -> bus_creator/771
  bus_selector19/53 -> outpmodule/894(VVMC_ADASLDWSta_enum)  "<VVMC_ADASLDWSta_enum>"
  outpmodule/873(VOUTP_ADASAEBReq_enum) -> bus_creator/873
  bus_selector19/51 -> outpmodule/892(VVMC_LeftTurnLightReq_flg)  "<VVMC_LeftTurnLightReq_flg>"
  bus_selector13/18 -> outpmodule/622(VSYS_Dash1_cnt)  "<VSYS_Dash1_cnt>"
  bus_selector19/49 -> outpmodule/890(VVMC_HazardWarningReq_flg)  "<VVMC_HazardWarningReq_flg>"
  outpmodule/861(VOUTP_ISOAccLimit_mps2) -> bus_creator/861
  bus_selector19/48 -> outpmodule/889(VVMC_ADASForceIdle_flg)  "<VVMC_ADASForceIdle_flg>"
  bus_selector19/46 -> outpmodule/887(VVMC_ADASShftPosnReqA_flg)  "<VVMC_ADASShftPosnReqA_flg>"
  outpmodule/638(VOUTP_WisrBootReason_raw32) -> bus_creator/638
  bus_selector9/6 -> outpmodule/522(VNMM_NodeID_enum)  "<VNMM_NodeID_enum>"
  bus_selector19/42 -> outpmodule/883(VVMC_ACCComfortBandUpper_mps2)  "<VVMC_ACCComfortBandUpper_mps2>"
  bus_selector19/36 -> outpmodule/877(VVMC_ADASDBSReq_enum)  "<VVMC_ADASDBSReq_enum>"
  bus_selector19/37 -> outpmodule/878(VVMC_ADASACCSta_enum)  "<VVMC_ADASACCSta_enum>"
  bus_selector19/74 -> outpmodule/915(VVMC_LVDAFailinfo_flg)  "<VVMC_LVDAFailinfo_flg>"
  outpmodule/451(VOUTP_AvgBattTempPSAL_C) -> bus_creator/451
  bus_selector19/31 -> outpmodule/872(VVMC_LKATOIAct_enum)  "<VVMC_LKATOIAct_enum>"
  outpmodule/504(VOUTP_KeyAreaPTG_enum) -> bus_creator/504
  bus_selector19/30 -> outpmodule/871(VVMC_LKATOIFault_flg)  "<VVMC_LKATOIFault_flg>"
  outpmodule/826(VOUTP_ETC1ShiftrPgs_enum) -> bus_creator/826
  bus_selector19/32 -> outpmodule/873(VVMC_ADASAEBReq_enum)  "<VVMC_ADASAEBReq_enum>"
  bus_selector19/26 -> outpmodule/867(VVMC_ActACCRequiredAccel_mps2)  "<VVMC_ActACCRequiredAccel_mps2>"
  bus_selector19/22 -> outpmodule/863(VVMC_ISOJerkLimit_mps3)  "<VVMC_ISOJerkLimit_mps3>"
  outpmodule/272(VOUTP_DCDC4PreDTC_raw32) -> bus_creator/272
  outpmodule/406(VOUTP_CLRDIST_km) -> bus_creator/406
  bus_selector4/137 -> outpmodule/383(VDDM_VCURAPSErrLv3_flg)  "<VDDM_VCURAPSErrLv3_flg>"
  outpmodule/315(VOUTP_RMLUSSDTC_raw32) -> bus_creator/315
  outpmodule/620(VOUTP_Country2_cnt) -> bus_creator/620
  bus_selector15/22 -> outpmodule/670(VTPM_TPMSCaliButtAllow_flg)  "<VTPM_TPMSCaliButtAllow_flg>"
  outpmodule/3(VOUTP_CACPresWarn_flg) -> bus_creator/3
  bus_selector4/136 -> outpmodule/382(VDDM_VCURAPSErrLv2_flg)  "<VDDM_VCURAPSErrLv2_flg>"
  bus_selector4/134 -> outpmodule/380(VDDM_EngagePFail_flg)  "<VDDM_EngagePFail_flg>"
  bus_selector6/21 -> outpmodule/422(VDID_PSAR_sec)  "<VDID_PSAR_sec>"
  bus_selector4/135 -> outpmodule/381(VDDM_DisengagePFail_flg)  "<VDDM_DisengagePFail_flg>"
  bus_selector19/21 -> outpmodule/862(VVMC_ISODecLimit_mps2)  "<VVMC_ISODecLimit_mps2>"
  outpmodule/477(VOUTP_CALID_cnt) -> bus_creator/477
  bus_selector4/133 -> outpmodule/379(VDDM_DTCDetect_enum)  "<VDDM_DTCDetect_enum>"
  bus_selector15/88 -> outpmodule/736(VTPM_FlashS2ID_raw)  "<VTPM_FlashS2ID_raw>"
  bus_selector4/130 -> outpmodule/376(VDDM_EPBLockTODTC_raw32)  "<VDDM_EPBLockTODTC_raw32>"
  bus_selector4/129 -> outpmodule/375(VDDM_5vAPS2PwrErrDTC_raw32)  "<VDDM_5vAPS2PwrErrDTC_raw32>"
  outpmodule/677(VOUTP_RFWheelTmpIndi_flg) -> bus_creator/677
  bus_selector4/128 -> outpmodule/374(VDDM_5vAPS1PwrErrDTC_raw32)  "<VDDM_5vAPS1PwrErrDTC_raw32>"
  outpmodule/28(VOUTP_PASDFCL_cm) -> bus_creator/28
  bus_selector4/126 -> outpmodule/372(VDDM_RRSensorFailDTC_raw32)  "<VDDM_RRSensorFailDTC_raw32>"
  outpmodule/519(VOUTP_Awake_enum) -> bus_creator/519
  bus_selector19/97 -> outpmodule/938(VVMC_LongAcc_Gps)  "<VVMC_LongAcc_Gps>"
  outpmodule/195(VOUTP_FDCBCMSMKRCmd_flg) -> bus_creator/195
  outpmodule/748(VOUTP_CreepIND_enum) -> bus_creator/748
  bus_selector4/124 -> outpmodule/370(VDDM_RFSensorFailDTC_raw32)  "<VDDM_RFSensorFailDTC_raw32>"
  bus_selector4/119 -> outpmodule/365(VDDM_LFWheelTmpHighDTC_raw32)  "<VDDM_LFWheelTmpHighDTC_raw32>"
  outpmodule/891(VOUTP_RightTurnLightReq_flg) -> bus_creator/891
  bus_selector16/51 -> outpmodule/796(VTQD_EC1EMReqSpdCtrlLoLmt_rpm)  "<VTQD_EC1EMReqSpdCtrlLoLmt_rpm>"
  bus_selector4/117 -> outpmodule/363(VDDM_LRPressIndiDTC_raw32)  "<VDDM_LRPressIndiDTC_raw32>"
  bus_selector16/19 -> outpmodule/764(VTQD_VCUEBSHBSw_enum)  "<VTQD_VCUEBSHBSw_enum>"
  outpmodule/439(VOUTP_GECHGOVCDCR_kWh) -> bus_creator/439
  outpmodule/667(VOUTP_RFWheelDebug_flg) -> bus_creator/667
  bus_selector4/118 -> outpmodule/364(VDDM_RRPressIndiDTC_raw32)  "<VDDM_RRPressIndiDTC_raw32>"
  outpmodule/117(VOUTP_YawRate_degps) -> bus_creator/117
  bus_selector4/115 -> outpmodule/361(VDDM_LFPressIndiDTC_raw32)  "<VDDM_LFPressIndiDTC_raw32>"
  bus_selector16/16 -> outpmodule/761(VTQD_VCUTMVehSpd_kph)  "<VTQD_VCUTMVehSpd_kph>"
  bus_selector4/111 -> outpmodule/357(VDDM_LFBatwarnDTC_raw32)  "<VDDM_LFBatwarnDTC_raw32>"
  outpmodule/489(VOUTP_STASUP_enum) -> bus_creator/489
  bus_selector4/110 -> outpmodule/356(VDDM_RrMCUTqErrDTC_raw32)  "<VDDM_RrMCUTqErrDTC_raw32>"
  outpmodule/171(VOUTP_APSSWVer_enum) -> bus_creator/171
  outpmodule/319(VOUTP_FLRUSSDTC_raw32) -> bus_creator/319
  bus_selector4/107 -> outpmodule/353(VDDM_ESC5RCErrDTC_raw32)  "<VDDM_ESC5RCErrDTC_raw32>"
  bus_selector6/88 -> outpmodule/489(VDID_STASUP_enum)  "<VDID_STASUP_enum>"
  outpmodule/555(VOUTP_HVILDetectFail_flg) -> bus_creator/555
  bus_selector4/109 -> outpmodule/355(VDDM_FrMCUTqErrDTC_raw32)  "<VDDM_FrMCUTqErrDTC_raw32>"
  bus_selector15/31 -> outpmodule/679(VTPM_RRWheelTmpIndi_flg)  "<VTPM_RRWheelTmpIndi_flg>"
  bus_selector4/106 -> outpmodule/352(VDDM_ESC1CSErrDTC_raw32)  "<VDDM_ESC1CSErrDTC_raw32>"
  outpmodule/111(VOUTP_SASCAL_flg) -> bus_creator/111
  bus_selector4/103 -> outpmodule/349(VDDM_ESC7RCErrDTC_raw32)  "<VDDM_ESC7RCErrDTC_raw32>"
  bus_selector6/51 -> outpmodule/452(VDID_AvgBattTempOVCR_C)  "<VDID_AvgBattTempOVCR_C>"
  outpmodule/200(VOUTP_FDCBCMSRTLpCmd_flg) -> bus_creator/200
  bus_selector4/102 -> outpmodule/348(VDDM_Shifter1CSErrDTC_raw32)  "<VDDM_Shifter1CSErrDTC_raw32>"
  bus_selector6/46 -> outpmodule/447(VDID_ResetCDEODTR_km)  "<VDID_ResetCDEODTR_km>"
  outpmodule/654(VOUTP_RFWheelPress_raw8) -> bus_creator/654
  bus_selector15/3 -> outpmodule/651(VTPM_LRBatWarn_flg)  "<VTPM_LRBatWarn_flg>"
  outpmodule/623(VOUTP_Change1_cnt) -> bus_creator/623
  bus_selector16/60 -> outpmodule/805(VTQD_EC1EMSupTSC1CtrlPG3_cnt)  "<VTQD_EC1EMSupTSC1CtrlPG3_cnt>"
  bus_selector4/101 -> outpmodule/347(VDDM_Shifter1RCErrDTC_raw32)  "<VDDM_Shifter1RCErrDTC_raw32>"
  outpmodule/575(VOUTP_V2BAux3RlyFit_enum) -> bus_creator/575
  bus_selector4/100 -> outpmodule/346(VDDM_MCUR1CSErrDTC_raw32)  "<VDDM_MCUR1CSErrDTC_raw32>"
  outpmodule/582(VOUTP_VSPReversed_flg) -> bus_creator/582
  bus_selector19/8 -> outpmodule/849(VVMC_VMCMSACtrlAvail_flg)  "<VVMC_VMCMSACtrlAvail_flg>"
  bus_selector4/97 -> outpmodule/343(VDDM_MCUF1RCErrDTC_raw32)  "<VDDM_MCUF1RCErrDTC_raw32>"
  bus_selector4/98 -> outpmodule/344(VDDM_MCUR1RCErrDTC_raw32)  "<VDDM_MCUR1RCErrDTC_raw32>"
  bus_selector19/52 -> outpmodule/893(VVMC_ADASFCWSta_enum)  "<VVMC_ADASFCWSta_enum>"
  bus_selector4/95 -> outpmodule/341(VDDM_MSAMalfuncDetDTC_raw32)  "<VDDM_MSAMalfuncDetDTC_raw32>"
  outpmodule/559(VOUTP_V2BAux3OnOff_enum) -> bus_creator/559
  bus_selector4/94 -> outpmodule/340(VDDM_CCMalfuncDetDTC_raw32)  "<VDDM_CCMalfuncDetDTC_raw32>"
  outpmodule/550(VOUTP_LostHVComActivePwrDown_flg) -> bus_creator/550
  BSYS_outputs/1 -> bus_selector13/1
  bus_selector6/23 -> outpmodule/424(VDID_IPSAR_sec)  "<VDID_IPSAR_sec>"
  outpmodule/321(VOUTP_RLRUSSDTC_raw32) -> bus_creator/321
  outpmodule/697(VOUTP_S4L_enum) -> bus_creator/697
  bus_selector4/92 -> outpmodule/338(VDDM_ACCAccelCmdErrDetDTC_raw32)  "<VDDM_ACCAccelCmdErrDetDTC_raw32>"
  bus_selector15/54 -> outpmodule/702(VTPM_RRP20_raw8)  "<VTPM_RRP20_raw8>"
  bus_selector4/93 -> outpmodule/339(VDDM_ACCMalfuncDetDTC_raw32)  "<VDDM_ACCMalfuncDetDTC_raw32>"
  outpmodule/139(VOUTP_ESCAPSSta_enum) -> bus_creator/139
  outpmodule/530(VOUTP_PowerUpState_enum) -> bus_creator/530
  bus_selector19/43 -> outpmodule/884(VVMC_ACCJerkLowerLimit_mps3)  "<VVMC_ACCJerkLowerLimit_mps3>"
  bus_selector4/90 -> outpmodule/336(VDDM_RrMCUSigErrDetDTC_raw32)  "<VDDM_RrMCUSigErrDetDTC_raw32>"
  bus_selector4/89 -> outpmodule/335(VDDM_FrMCUSigErrDetDTC_raw32)  "<VDDM_FrMCUSigErrDetDTC_raw32>"
  outpmodule/767(VOUTP_EVCU1EMotorSpd_rpm) -> bus_creator/767
  bus_selector4/87 -> outpmodule/333(VDDM_BMSSigErrDetDTC_raw32)  "<VDDM_BMSSigErrDetDTC_raw32>"
  outpmodule/114(VOUTP_SASVTimeOut_flg) -> bus_creator/114
  bus_selector4/88 -> outpmodule/334(VDDM_FCMACCSigErrDetDTC_raw32)  "<VDDM_FCMACCSigErrDetDTC_raw32>"
  outpmodule/151(VOUTP_AVMparkingexcute_enum) -> bus_creator/151
  bus_selector19/96 -> outpmodule/937(VVMC_APSReq_enum)  "<VVMC_APSReq_enum>"
  bus_selector4/85 -> outpmodule/331(VDDM_FCM5CSErrDTC_raw32)  "<VDDM_FCM5CSErrDTC_raw32>"
  bus_selector13/29 -> outpmodule/633(VSYS_SHA8_cnt)  "<VSYS_SHA8_cnt>"
  bus_selector4/83 -> outpmodule/329(VDDM_FCM4CSErrDTC_raw32)  "<VDDM_FCM4CSErrDTC_raw32>"
  bus_selector4/86 -> outpmodule/332(VDDM_ZoneSCPNoComDTC_raw32)  "<VDDM_ZoneSCPNoComDTC_raw32>"
  outpmodule/94(VOUTP_RFPulseCountTimeOut_flg) -> bus_creator/94
  bus_selector15/83 -> outpmodule/731(VTPM_Flashdatavalid_enum)  "<VTPM_Flashdatavalid_enum>"
  bus_selector4/81 -> outpmodule/327(VDDM_FCM3CSErrDTC_raw32)  "<VDDM_FCM3CSErrDTC_raw32>"
  bus_selector4/82 -> outpmodule/328(VDDM_FCM4NoComDTC_raw32)  "<VDDM_FCM4NoComDTC_raw32>"
  bus_selector16/40 -> outpmodule/785(VTQD_EC1EMSpdIdleP2_rpm)  "<VTQD_EC1EMSpdIdleP2_rpm>"
  bus_selector4/77 -> outpmodule/323(VDDM_FCM2RCErrDTC_raw32)  "<VDDM_FCM2RCErrDTC_raw32>"
  outpmodule/912(VOUTP_ADASLFCHandsOffWarning_enum) -> bus_creator/912
  bus_selector15/70 -> outpmodule/718(VTPM_LFPindi_enum)  "<VTPM_LFPindi_enum>"
  outpmodule/634(VOUTP_NvWriteReqRisingEdge_flg) -> bus_creator/634
  bus_selector19/54 -> outpmodule/895(VVMC_ADASFltWrnReq_flg)  "<VVMC_ADASFltWrnReq_flg>"
  outpmodule/203(VOUTP_FDCBCMStopINDCmd_flg) -> bus_creator/203
  bus_selector4/78 -> outpmodule/324(VDDM_FCM2CSErrDTC_raw32)  "<VDDM_FCM2CSErrDTC_raw32>"
  bus_selector4/72 -> outpmodule/318(VDDM_FLLUSSDTC_raw32)  "<VDDM_FLLUSSDTC_raw32>"
  bus_selector4/74 -> outpmodule/320(VDDM_RLLUSSDTC_raw32)  "<VDDM_RLLUSSDTC_raw32>"
  bus_selector4/71 -> outpmodule/317(VDDM_RCRUSSDTC_raw32)  "<VDDM_RCRUSSDTC_raw32>"
  outpmodule/692(VOUTP_S3ID_raw32) -> bus_creator/692
  bus_selector4/68 -> outpmodule/314(VDDM_RCLUSSDTC_raw32)  "<VDDM_RCLUSSDTC_raw32>"
  bus_selector4/66 -> outpmodule/312(VDDM_FMRUSSDTC_raw32)  "<VDDM_FMRUSSDTC_raw32>"
  outpmodule/802(VOUTP_EC1EMDefTrqLmt_rpm) -> bus_creator/802
  bus_selector4/64 -> outpmodule/310(VDDM_FCLUSSDTC_raw32)  "<VDDM_FCLUSSDTC_raw32>"
  bus_selector4/62 -> outpmodule/308(VDDM_DiagRLTSDTC_raw32)  "<VDDM_DiagRLTSDTC_raw32>"
  bus_selector4/57 -> outpmodule/303(VDDM_ESC5NoComDTC_raw32)  "<VDDM_ESC5NoComDTC_raw32>"
  outpmodule/881(VOUTP_TimeGapLevel_enum) -> bus_creator/881
  bus_selector16/84 -> outpmodule/829(VTQD_EMRC1RetSelNonEng_pct)  "<VTQD_EMRC1RetSelNonEng_pct>"
  outpmodule/160(VOUTP_CAASSwTimeOut_flg) -> bus_creator/160
  outpmodule/408(VOUTP_APPE_pct) -> bus_creator/408
  bus_selector4/52 -> outpmodule/298(VDDM_MCUF1NoComDTC_raw32)  "<VDDM_MCUF1NoComDTC_raw32>"
  bus_selector4/53 -> outpmodule/299(VDDM_MCUR1NoComDTC_raw32)  "<VDDM_MCUR1NoComDTC_raw32>"
  BTQD_outputs/1 -> bus_selector16/1
  bus_selector4/49 -> outpmodule/295(VDDM_APS1SigOoRDTC_raw32)  "<VDDM_APS1SigOoRDTC_raw32>"
  BTQR_outputs/1 -> bus_selector17/1
  bus_selector4/48 -> outpmodule/294(VDDM_VehMalfunLevel_enum)  "<VDDM_VehMalfunLevel_enum>"
  outpmodule/939(VOUTP_CCMSASpdWar_flg) -> bus_creator/939
  bus_selector4/45 -> outpmodule/291(VDDM_HoodSWDTC_raw32)  "<VDDM_HoodSWDTC_raw32>"
  outpmodule/232(VOUTP_FDCBCMRRoomLpCmd_pct) -> bus_creator/232
  bus_selector12/8 -> outpmodule/597(VSCP_DTbyte0_raw)  "<VSCP_DTbyte0_raw>"
  bus_selector19/55 -> outpmodule/896(VVMC_ACCObjDstLvl_enum)  "<VVMC_ACCObjDstLvl_enum>"
  outpmodule/818(VOUTP_RC1PctTrqP3_pct) -> bus_creator/818
  bus_selector4/43 -> outpmodule/289(VDDM_FRDoorSWDTC_raw32)  "<VDDM_FRDoorSWDTC_raw32>"
  bus_selector4/44 -> outpmodule/290(VDDM_RRDoorSWDTC_raw32)  "<VDDM_RRDoorSWDTC_raw32>"
  bus_selector4/40 -> outpmodule/286(VDDM_DrStSWDTC_raw32)  "<VDDM_DrStSWDTC_raw32>"
  bus_selector15/56 -> outpmodule/704(VTPM_IDin_raw32)  "<VTPM_IDin_raw32>"
  bus_selector4/138 -> outpmodule/384(VDDM_EDriveSysErrShifterErr_flg)  "<VDDM_EDriveSysErrShifterErr_flg>"
  outpmodule/50(VOUTP_USSStaFLL_flg) -> bus_creator/50
  bus_selector7/19 -> outpmodule/512(VDKC_JudgeKeepUnlockZone_flg)  "<VDKC_JudgeKeepUnlockZone_flg>"
  bus_selector4/7 -> outpmodule/253(VDDM_C3CCU1RCDTC_raw32)  "<VDDM_C3CCU1RCDTC_raw32>"
  outpmodule/21(VOUTP_PASDRMR_cm) -> bus_creator/21
  outpmodule/339(VOUTP_ACCMalfuncDetDTC_raw32) -> bus_creator/339
  bus_selector4/8 -> outpmodule/254(VDDM_C3CCU1CSDTC_raw32)  "<VDDM_C3CCU1CSDTC_raw32>"
  bus_selector4/5 -> outpmodule/251(VDDM_C3BMS1CSDTC_raw32)  "<VDDM_C3BMS1CSDTC_raw32>"
  bus_selector4/4 -> outpmodule/250(VDDM_C3BMS1RCDTC_raw32)  "<VDDM_C3BMS1RCDTC_raw32>"
  bus_selector4/3 -> outpmodule/249(VDDM_C3BMS6LCDTC_raw32)  "<VDDM_C3BMS6LCDTC_raw32>"
  bus_selector19/6 -> outpmodule/847(VVMC_VMCACCCtrlAvail_flg)  "<VVMC_VMCACCCtrlAvail_flg>"
  bus_selector4/2 -> outpmodule/248(VDDM_C3BMS6CSDTC_raw32)  "<VDDM_C3BMS6CSDTC_raw32>"
  bus_selector4/1 -> outpmodule/247(VDDM_C3BMS6RCDTC_raw32)  "<VDDM_C3BMS6RCDTC_raw32>"
  bus_selector13/7 -> outpmodule/611(VSYS_ECU1_cnt)  "<VSYS_ECU1_cnt>"
  bus_selector6/87 -> outpmodule/488(VDID_VinCode_cnt)  "<VDID_VinCode_cnt>"
  bus_selector4/11 -> outpmodule/257(VDDM_C3CCU2CSDTC_raw32)  "<VDDM_C3CCU2CSDTC_raw32>"
  outpmodule/299(VOUTP_MCUR1NoComDTC_raw32) -> bus_creator/299
  bus_selector4/31 -> outpmodule/277(VDDM_MidLvSaChkDTC_raw32)  "<VDDM_MidLvSaChkDTC_raw32>"
  outpmodule/255(VOUTP_C3CCU1LCDTC_raw32) -> bus_creator/255
  bus_selector4/22 -> outpmodule/268(VDDM_KeyAuthDTC_raw32)  "<VDDM_KeyAuthDTC_raw32>"
  bus_selector4/132 -> outpmodule/378(VDDM_LimpHomeActTmp_flg)  "<VDDM_LimpHomeActTmp_flg>"
  bus_selector4/24 -> outpmodule/270(VDDM_HVB4PreDTC_raw32)  "<VDDM_HVB4PreDTC_raw32>"
  bus_selector4/21 -> outpmodule/267(VDDM_BrkSWNoBacDTC_raw32)  "<VDDM_BrkSWNoBacDTC_raw32>"
  outpmodule/33(VOUTP_PASAFCL_enum) -> bus_creator/33
  bus_selector4/23 -> outpmodule/269(VDDM_ONtoRdyDTC_raw32)  "<VDDM_ONtoRdyDTC_raw32>"
  outpmodule/812(VOUTP_RC1RetCtrlMth_enum) -> bus_creator/812
  bus_selector4/39 -> outpmodule/285(VDDM_LVSupHiDTC_raw32)  "<VDDM_LVSupHiDTC_raw32>"
  bus_selector19/78 -> outpmodule/919(VVMC_FCMACCmode_enum)  "<VVMC_FCMACCmode_enum>"
  outpmodule/787(VOUTP_EC1EMSpdIdleP3_rpm) -> bus_creator/787
  bus_selector4/18 -> outpmodule/264(VDDM_Lv3ErrDTC_raw32)  "<VDDM_Lv3ErrDTC_raw32>"
  outpmodule/46(VOUTP_USSStaRCL_flg) -> bus_creator/46
  bus_selector4/16 -> outpmodule/262(VDDM_Lv1ErrDTC_raw32)  "<VDDM_Lv1ErrDTC_raw32>"
  outpmodule/12(VOUTP_EHPSDisEnTimeout_flg) -> bus_creator/12
  bus_selector4/14 -> outpmodule/260(VDDM_C1ABM1CSDTC_raw32)  "<VDDM_C1ABM1CSDTC_raw32>"
  bus_selector4/15 -> outpmodule/261(VDDM_C1ABM1LCDTC_raw32)  "<VDDM_C1ABM1LCDTC_raw32>"
  outpmodule/158(VOUTP_IVIStatusTimeOut_flg) -> bus_creator/158
  bus_selector19/24 -> outpmodule/865(VVMC_DISCReqAcc_mps2)  "<VVMC_DISCReqAcc_mps2>"
  bus_selector6/75 -> outpmodule/476(VDID_RESSCNTSDODRNGAXIS_enum)  "<VDID_RESSCNTSDODRNGAXIS_enum>"
  bus_selector4/13 -> outpmodule/259(VDDM_C1ABM1RCDTC_raw32)  "<VDDM_C1ABM1RCDTC_raw32>"
  bus_selector4/12 -> outpmodule/258(VDDM_C3CCU2LCDTC_raw32)  "<VDDM_C3CCU2LCDTC_raw32>"
  bus_selector3/54 -> outpmodule/244(VBCM_FDCBCMTurnBuzzerENSta_flg)  "<VBCM_FDCBCMTurnBuzzerENSta_flg>"
  outpmodule/128(VOUTP_LatAccelVTimeOut_flg) -> bus_creator/128
  bus_selector3/51 -> outpmodule/241(VBCM_FDCBCMRTurnSWSta_flg)  "<VBCM_FDCBCMRTurnSWSta_flg>"
  outpmodule/101(VOUTP_DriIntend_enum) -> bus_creator/101
  outpmodule/263(VOUTP_Lv2ErrDTC_raw32) -> bus_creator/263
  bus_selector9/4 -> outpmodule/520(VNMM_CSB_flg)  "<VNMM_CSB_flg>"
  bus_selector3/52 -> outpmodule/242(VBCM_FDCBCMRGearSta_flg)  "<VBCM_FDCBCMRGearSta_flg>"
  bus_selector3/47 -> outpmodule/237(VBCM_FDCBCMFDCloseSVCmd_flg)  "<VBCM_FDCBCMFDCloseSVCmd_flg>"
  bus_selector4/10 -> outpmodule/256(VDDM_C3CCU2RCDTC_raw32)  "<VDDM_C3CCU2RCDTC_raw32>"
  bus_selector3/50 -> outpmodule/240(VBCM_FDCBCMLTurnSWSta_flg)  "<VBCM_FDCBCMLTurnSWSta_flg>"
  outpmodule/528(VOUTP_NetworkReq_flg) -> bus_creator/528
  outpmodule/732(VOUTP_unlearnSfali_flg) -> bus_creator/732
  bus_selector15/51 -> outpmodule/699(VTPM_LFP20_raw8)  "<VTPM_LFP20_raw8>"
  outpmodule/941(VOUTP_CAASCtrlAvail_flg) -> bus_creator/941
  bus_selector16/27 -> outpmodule/772(VTQD_EVCU2MinTorqAvail_pct)  "<VTQD_EVCU2MinTorqAvail_pct>"
  bus_selector3/48 -> outpmodule/238(VBCM_FDCBCMMDOpenSVCmd_flg)  "<VBCM_FDCBCMMDOpenSVCmd_flg>"
  outpmodule/576(VOUTP_V2BAux4RlySta_enum) -> bus_creator/576
  bus_selector3/46 -> outpmodule/236(VBCM_FDCBCMFDOpenSVCmd_flg)  "<VBCM_FDCBCMFDOpenSVCmd_flg>"
  outpmodule/568(VOUTP_V2BDCDCPosRlySta_enum) -> bus_creator/568
  bus_selector4/42 -> outpmodule/288(VDDM_RLDoorSWDTC_raw32)  "<VDDM_RLDoorSWDTC_raw32>"
  bus_selector15/37 -> outpmodule/685(VTPM_AutoLTips_enum)  "<VTPM_AutoLTips_enum>"
  bus_selector12/9 -> outpmodule/598(VSCP_DTbyte1_raw)  "<VSCP_DTbyte1_raw>"
  bus_selector3/41 -> outpmodule/231(VBCM_FDCBCMRRoomLpSetSta_pct)  "<VBCM_FDCBCMRRoomLpSetSta_pct>"
  bus_selector12/13 -> outpmodule/602(VSCP_DTbyte5_raw)  "<VSCP_DTbyte5_raw>"
  bus_selector3/43 -> outpmodule/233(VBCM_FDCBCMHelpINDCmd_flg)  "<VBCM_FDCBCMHelpINDCmd_flg>"
  outpmodule/874(VOUTP_ADASFaultSta_flg) -> bus_creator/874
  outpmodule/303(VOUTP_ESC5NoComDTC_raw32) -> bus_creator/303
  bus_selector3/42 -> outpmodule/232(VBCM_FDCBCMRRoomLpCmd_pct)  "<VBCM_FDCBCMRRoomLpCmd_pct>"
  outpmodule/260(VOUTP_C1ABM1CSDTC_raw32) -> bus_creator/260
  bus_selector4/122 -> outpmodule/368(VDDM_RRWheelTmpHighDTC_raw32)  "<VDDM_RRWheelTmpHighDTC_raw32>"
  bus_selector15/6 -> outpmodule/654(VTPM_RFWheelPress_raw8)  "<VTPM_RFWheelPress_raw8>"
  bus_selector7/9 -> outpmodule/502(VDKC_PCommandToBCM_enum)  "<VDKC_PCommandToBCM_enum>"
  bus_selector3/38 -> outpmodule/228(VBCM_FDCBCMFRoomLpCmd_pct)  "<VBCM_FDCBCMFRoomLpCmd_pct>"
  bus_selector3/35 -> outpmodule/225(VBCM_FDCBCMRoomLpAmbSetSta_flg)  "<VBCM_FDCBCMRoomLpAmbSetSta_flg>"
  bus_selector12/5 -> outpmodule/594(VSCP_CFGEM1BAMRsv_raw)  "<VSCP_CFGEM1BAMRsv_raw>"
  BDSC_outputs/1 -> bus_selector8/1
  bus_selector3/37 -> outpmodule/227(VBCM_FDCBCMFRoomLpSetSta_pct)  "<VBCM_FDCBCMFRoomLpSetSta_pct>"
  bus_selector4/58 -> outpmodule/304(VDDM_EnterNewOperCyc_flg)  "<VDDM_EnterNewOperCyc_flg>"
  outpmodule/88(VOUTP_LRPulseCountVTimeOut_flg) -> bus_creator/88
  bus_selector3/32 -> outpmodule/222(VBCM_FDCBCMEmExitSWSta_flg)  "<VBCM_FDCBCMEmExitSWSta_flg>"
  bus_selector4/70 -> outpmodule/316(VDDM_RMRUSSDTC_raw32)  "<VDDM_RMRUSSDTC_raw32>"
  outpmodule/102(VOUTP_DriIntendTimeOut_flg) -> bus_creator/102
  bus_selector15/41 -> outpmodule/689(VTPM_RRSensorMode_flg)  "<VTPM_RRSensorMode_flg>"
  outpmodule/31(VOUTP_APSDFLR_cm) -> bus_creator/31
  bus_selector3/33 -> outpmodule/223(VBCM_InnerBuzzerModeSta_enum)  "<VBCM_InnerBuzzerModeSta_enum>"
  bus_selector3/31 -> outpmodule/221(VBCM_FDCBCMRBSDYCmd_flg)  "<VBCM_FDCBCMRBSDYCmd_flg>"
  bus_selector3/29 -> outpmodule/219(VBCM_FDCBCMLBSDYCmd_flg)  "<VBCM_FDCBCMLBSDYCmd_flg>"
  bus_selector3/27 -> outpmodule/217(VBCM_FDCBCMRoomLpAmbCmd_flg)  "<VBCM_FDCBCMRoomLpAmbCmd_flg>"
  outpmodule/824(VOUTP_VCUMCUGearSta_enum) -> bus_creator/824
  bus_selector3/25 -> outpmodule/215(VBCM_FDCBCMMDoorSta_flg)  "<VBCM_FDCBCMMDoorSta_flg>"
  bus_selector3/22 -> outpmodule/212(VBCM_FDCBCMRFLampCmd_flg)  "<VBCM_FDCBCMRFLampCmd_flg>"
  bus_selector19/103 -> outpmodule/944(VVMC_CalibratedAccX_G)  "<VVMC_CalibratedAccX_G>"
  outpmodule/851(VOUTP_FeatReqSpd_kph) -> bus_creator/851
  bus_selector3/23 -> outpmodule/213(VBCM_TurnLpPatternSta_enum)  "<VBCM_TurnLpPatternSta_enum>"
  bus_selector15/69 -> outpmodule/717(VTPM_TPMSResButt_flg)  "<VTPM_TPMSResButt_flg>"
  bus_selector3/21 -> outpmodule/211(VBCM_FDCBCMRDRLCmd_flg)  "<VBCM_FDCBCMRDRLCmd_flg>"
  bus_selector3/17 -> outpmodule/207(VBCM_FDCBCMWiperHCmd_flg)  "<VBCM_FDCBCMWiperHCmd_flg>"
  bus_selector4/141 -> outpmodule/387(VDDM_MCUActDisFail_flg)  "<VDDM_MCUActDisFail_flg>"
  bus_selector3/15 -> outpmodule/205(VBCM_FDCBCMInnerCallBellCmd_flg)  "<VBCM_FDCBCMInnerCallBellCmd_flg>"
  bus_selector3/12 -> outpmodule/202(VBCM_FDCBCMRTurnLpCmd_flg)  "<VBCM_FDCBCMRTurnLpCmd_flg>"
  bus_selector4/37 -> outpmodule/283(VDDM_IniLVLoDTC_raw32)  "<VDDM_IniLVLoDTC_raw32>"
  outpmodule/190(VOUTP_IVIUserTakeOverAPSSta_flg) -> bus_creator/190
  bus_selector3/10 -> outpmodule/200(VBCM_FDCBCMSRTLpCmd_flg)  "<VBCM_FDCBCMSRTLpCmd_flg>"
  outpmodule/72(VOUTP_LRRawWhlSpeedVTimeOut_flg) -> bus_creator/72
  bus_selector3/7 -> outpmodule/197(VBCM_FDCBCMDVRSignalRCmd_flg)  "<VBCM_FDCBCMDVRSignalRCmd_flg>"
  bus_selector4/113 -> outpmodule/359(VDDM_LRBatwarnDTC_raw32)  "<VDDM_LRBatwarnDTC_raw32>"
  outpmodule/442(VOUTP_GECHGOVCACL_kWh) -> bus_creator/442
  bus_selector3/8 -> outpmodule/198(VBCM_FDCBCMBSDBuzzerCmd_flg)  "<VBCM_FDCBCMBSDBuzzerCmd_flg>"
  bus_selector19/45 -> outpmodule/886(VVMC_ADASVehSpdLim_raw32)  "<VVMC_ADASVehSpdLim_raw32>"
  bus_selector6/53 -> outpmodule/454(VDID_AvgBattTempOFFR_C)  "<VDID_AvgBattTempOFFR_C>"
  bus_selector3/9 -> outpmodule/199(VBCM_FDCBCMSLTLpCmd_flg)  "<VBCM_FDCBCMSLTLpCmd_flg>"
  bus_selector3/36 -> outpmodule/226(VBCM_FDCBCMRoomLpSetSta_flg)  "<VBCM_FDCBCMRoomLpSetSta_flg>"
  outpmodule/41(VOUTP_USSStaRMR_flg) -> bus_creator/41
  bus_selector3/6 -> outpmodule/196(VBCM_FDCBCMDVRSignalLCmd_flg)  "<VBCM_FDCBCMDVRSignalLCmd_flg>"
  outpmodule/774(VOUTP_EEC3EMPressLoss_pct) -> bus_creator/774
  bus_selector3/4 -> outpmodule/194(VBCM_FDCBCMSMKLCmd_flg)  "<VBCM_FDCBCMSMKLCmd_flg>"
  bus_selector6/42 -> outpmodule/443(VDID_RESSV2XENNONPSAR_kWh)  "<VDID_RESSV2XENNONPSAR_kWh>"
  bus_selector3/1 -> outpmodule/191(VBCM_FDCBCMLBeamCmd_flg)  "<VBCM_FDCBCMLBeamCmd_flg>"
  bus_selector3/2 -> outpmodule/192(VBCM_FDCBCMPLampCmd_flg)  "<VBCM_FDCBCMPLampCmd_flg>"
  bus_selector4/120 -> outpmodule/366(VDDM_RFWheelTmpHighDTC_raw32)  "<VDDM_RFWheelTmpHighDTC_raw32>"
  outpmodule/196(VOUTP_FDCBCMDVRSignalLCmd_flg) -> bus_creator/196
  bus_selector15/36 -> outpmodule/684(VTPM_CWheelTips_enum)  "<VTPM_CWheelTips_enum>"
  bus_selector4/32 -> outpmodule/278(VDDM_MCUDisDTC_raw32)  "<VDDM_MCUDisDTC_raw32>"
  bus_selector3/3 -> outpmodule/193(VBCM_FDCBCMHBeamCmd_flg)  "<VBCM_FDCBCMHBeamCmd_flg>"
  outpmodule/932(VOUTP_APSCtrlAvail_flg) -> bus_creator/932
  bus_selector4/127 -> outpmodule/373(VDDM_C1EPAS2LCDTC_raw32)  "<VDDM_C1EPAS2LCDTC_raw32>"
  bus_selector14/3 -> outpmodule/648(VTHC_AfterrunningMode_flg)  "<VTHC_AfterrunningMode_flg>"
  outpmodule/397(VOUTP_EAPS1MIN_pct) -> bus_creator/397
  bus_selector18/4 -> outpmodule/838(VV2L_ReqOBCExtrV2LEna_enum)  "<VV2L_ReqOBCExtrV2LEna_enum>"
  bus_selector4/36 -> outpmodule/282(VDDM_OBC4PreDTC_raw32)  "<VDDM_OBC4PreDTC_raw32>"
  outpmodule/719(VOUTP_RFPind_enum) -> bus_creator/719
  bus_selector4/33 -> outpmodule/279(VDDM_DCDCDisDTC_raw32)  "<VDDM_DCDCDisDTC_raw32>"
  bus_selector4/29 -> outpmodule/275(VDDM_DCDCEnaDTC_raw32)  "<VDDM_DCDCEnaDTC_raw32>"
  outpmodule/199(VOUTP_FDCBCMSLTLpCmd_flg) -> bus_creator/199
  bus_selector2/175 -> outpmodule/190(VAPM_IVIUserTakeOverAPSSta_flg)  "<VAPM_IVIUserTakeOverAPSSta_flg>"
  bus_selector2/170 -> outpmodule/185(VAPM_RAPSBCMLamp_enum)  "<VAPM_RAPSBCMLamp_enum>"
  bus_selector19/28 -> outpmodule/869(VVMC_ADASLKASta_enum)  "<VVMC_ADASLKASta_enum>"
  bus_selector2/171 -> outpmodule/186(VAPM_RAPSBCMLockReq_flg)  "<VAPM_RAPSBCMLockReq_flg>"
  bus_selector19/38 -> outpmodule/879(VVMC_ACCObjDist_m)  "<VVMC_ACCObjDist_m>"
  outpmodule/920(VOUTP_ADASLanetypeR_enum) -> bus_creator/920
  bus_selector2/173 -> outpmodule/188(VAPM_RAPSErrWarnSta_enum)  "<VAPM_RAPSErrWarnSta_enum>"
  bus_selector2/168 -> outpmodule/183(VAPM_APSSpeedCMD_kph)  "<VAPM_APSSpeedCMD_kph>"
  bus_selector2/169 -> outpmodule/184(VAPM_APSVMCReqA_flg)  "<VAPM_APSVMCReqA_flg>"
  bus_selector2/164 -> outpmodule/179(VAPM_DKCParkingModeCmd_enum)  "<VAPM_DKCParkingModeCmd_enum>"
  outpmodule/153(VOUTP_AVMParkingmode_enum) -> bus_creator/153
  bus_selector2/163 -> outpmodule/178(VAPM_DKCPDkeyAreaRAPSSta_enum)  "<VAPM_DKCPDkeyAreaRAPSSta_enum>"
  bus_selector19/50 -> outpmodule/891(VVMC_RightTurnLightReq_flg)  "<VVMC_RightTurnLightReq_flg>"
  bus_selector2/162 -> outpmodule/177(VAPM_CAASSta_enum)  "<VAPM_CAASSta_enum>"
  bus_selector9/12 -> outpmodule/528(VNMM_NetworkReq_flg)  "<VNMM_NetworkReq_flg>"
  bus_selector2/158 -> outpmodule/173(VAPM_APSExitCondition_enum)  "<VAPM_APSExitCondition_enum>"
  bus_selector13/33 -> outpmodule/637(VSYS_PmicBootReason_enum)  "<VSYS_PmicBootReason_enum>"
  bus_selector16/47 -> outpmodule/792(VTQD_EC1EMSpdIdleP5_rpm)  "<VTQD_EC1EMSpdIdleP5_rpm>"
  bus_selector4/140 -> outpmodule/386(VDDM_HVRlyOpFail_flg)  "<VDDM_HVRlyOpFail_flg>"
  outpmodule/78(VOUTP_RFWhlRotDirTimeOut_flg) -> bus_creator/78
  outpmodule/615(VOUTP_Minor1_cnt) -> bus_creator/615
  bus_selector2/161 -> outpmodule/176(VAPM_APSRqEPASCtrl_flg)  "<VAPM_APSRqEPASCtrl_flg>"
  bus_selector2/157 -> outpmodule/172(VAPM_APSHWVer_enum)  "<VAPM_APSHWVer_enum>"
  outpmodule/91(VOUTP_LFPulseCount_enum) -> bus_creator/91
  bus_selector2/156 -> outpmodule/171(VAPM_APSSWVer_enum)  "<VAPM_APSSWVer_enum>"
  bus_selector4/131 -> outpmodule/377(VDDM_EPBUnlockTODTC_raw32)  "<VDDM_EPBUnlockTODTC_raw32>"
  bus_selector15/27 -> outpmodule/675(VTPM_TPMSWarnIndi_enum)  "<VTPM_TPMSWarnIndi_enum>"
  bus_selector6/14 -> outpmodule/415(VDID_HVBCellVoltMin_V)  "<VDID_HVBCellVoltMin_V>"
  bus_selector2/152 -> outpmodule/167(VAPM_DriverSeatBeltCmd_flg)  "<VAPM_DriverSeatBeltCmd_flg>"
  outpmodule/132(VOUTP_MCPressureVTimeOut_flg) -> bus_creator/132
  bus_selector2/154 -> outpmodule/169(VAPM_APSProgressPCT_pct)  "<VAPM_APSProgressPCT_pct>"
  outpmodule/683(VOUTP_RRWheelPSW_raw8) -> bus_creator/683
  bus_selector2/151 -> outpmodule/166(VAPM_TCSActiveTimeOut_flg)  "<VAPM_TCSActiveTimeOut_flg>"
  bus_selector2/149 -> outpmodule/164(VAPM_ABSActiveTimeOut_flg)  "<VAPM_ABSActiveTimeOut_flg>"
  bus_selector4/51 -> outpmodule/297(VDDM_APSCorrErrDTC_raw32)  "<VDDM_APSCorrErrDTC_raw32>"
  bus_selector12/14 -> outpmodule/603(VSCP_DTbyte6_raw)  "<VSCP_DTbyte6_raw>"
  bus_selector10/40 -> outpmodule/568(VPMM_V2BDCDCPosRlySta_enum)  "<VPMM_V2BDCDCPosRlySta_enum>"
  bus_selector2/148 -> outpmodule/163(VAPM_ABSActive_flg)  "<VAPM_ABSActive_flg>"
  bus_selector2/141 -> outpmodule/156(VAPM_AVMErrSTATimeOut_flg)  "<VAPM_AVMErrSTATimeOut_flg>"
  outpmodule/934(VOUTP_APSStaSys_enum) -> bus_creator/934
  bus_selector4/125 -> outpmodule/371(VDDM_LRSensorFailDTC_raw32)  "<VDDM_LRSensorFailDTC_raw32>"
  outpmodule/584(VOUTP_VSPTurnLeft_enum) -> bus_creator/584
  bus_selector2/145 -> outpmodule/160(VAPM_CAASSwTimeOut_flg)  "<VAPM_CAASSwTimeOut_flg>"
  outpmodule/96(VOUTP_LRPulseCountTimeOut_flg) -> bus_creator/96
  bus_selector2/144 -> outpmodule/159(VAPM_CAASSw_enum)  "<VAPM_CAASSw_enum>"
  bus_selector14/1 -> outpmodule/646(VTHC_EWPPEReq_rpm)  "<VTHC_EWPPEReq_rpm>"
  bus_selector16/34 -> outpmodule/779(VTQD_EMRC1ActEMpTrq_pct)  "<VTQD_EMRC1ActEMpTrq_pct>"
  bus_selector2/138 -> outpmodule/153(VAPM_AVMParkingmode_enum)  "<VAPM_AVMParkingmode_enum>"
  outpmodule/109(VOUTP_SASSpeedValid_flg) -> bus_creator/109
  bus_selector2/137 -> outpmodule/152(VAPM_AVMparkingexcuteTimeOut_flg)  "<VAPM_AVMparkingexcuteTimeOut_flg>"
  bus_selector4/112 -> outpmodule/358(VDDM_RFBatwarnDTC_raw32)  "<VDDM_RFBatwarnDTC_raw32>"
  outpmodule/552(VOUTP_ChrgPowerUpFail_flg) -> bus_creator/552
  bus_selector3/26 -> outpmodule/216(VBCM_FDCBCMRDoorSta_flg)  "<VBCM_FDCBCMRDoorSta_flg>"
  bus_selector19/44 -> outpmodule/885(VVMC_ACCComfortBandLower_mps2)  "<VVMC_ACCComfortBandLower_mps2>"
  outpmodule/656(VOUTP_RRWheelPress_raw8) -> bus_creator/656
  bus_selector2/134 -> outpmodule/149(VAPM_AVMparkingcancel_enum)  "<VAPM_AVMparkingcancel_enum>"
  outpmodule/676(VOUTP_LFWheelTmpIndi_flg) -> bus_creator/676
  bus_selector2/135 -> outpmodule/150(VAPM_AVMparkingcancelTimeOut_flg)  "<VAPM_AVMparkingcancelTimeOut_flg>"
  outpmodule/632(VOUTP_SHA7_cnt) -> bus_creator/632
  bus_selector2/132 -> outpmodule/147(VAPM_EPBSta_enum)  "<VAPM_EPBSta_enum>"
  bus_selector19/79 -> outpmodule/920(VVMC_ADASLanetypeR_enum)  "<VVMC_ADASLanetypeR_enum>"
  outpmodule/779(VOUTP_EMRC1ActEMpTrq_pct) -> bus_creator/779
  bus_selector6/39 -> outpmodule/440(VDID_GECHGOVCDCL_kWh)  "<VDID_GECHGOVCDCL_kWh>"
  bus_selector15/14 -> outpmodule/662(VTPM_RFSensorFail_flg)  "<VTPM_RFSensorFail_flg>"
  bus_selector2/127 -> outpmodule/142(VAPM_EPBExtReleaseAvailTimeOut_flg)  "<VAPM_EPBExtReleaseAvailTimeOut_flg>"
  outpmodule/718(VOUTP_LFPindi_enum) -> bus_creator/718
  bus_selector2/128 -> outpmodule/143(VAPM_EPBExtApplyAvail_flg)  "<VAPM_EPBExtApplyAvail_flg>"
  bus_selector2/126 -> outpmodule/141(VAPM_EPBExtReleaseAvail_flg)  "<VAPM_EPBExtReleaseAvail_flg>"
  outpmodule/659(VOUTP_LRWheelTemp_C) -> bus_creator/659
  bus_selector10/16 -> outpmodule/544(VPMM_HVSysReady_enum)  "<VPMM_HVSysReady_enum>"
  bus_selector2/124 -> outpmodule/139(VAPM_ESCAPSSta_enum)  "<VAPM_ESCAPSSta_enum>"
  bus_selector2/125 -> outpmodule/140(VAPM_ESCAPSStaTimeOut_flg)  "<VAPM_ESCAPSStaTimeOut_flg>"
  bus_selector3/39 -> outpmodule/229(VBCM_FDCBCMMRoomLpSetSta_pct)  "<VBCM_FDCBCMMRoomLpSetSta_pct>"
  bus_selector15/57 -> outpmodule/705(VTPM_S1WheelDebugALTU_pct)  "<VTPM_S1WheelDebugALTU_pct>"
  bus_selector2/123 -> outpmodule/138(VAPM_ESCStandstillTimeOut_flg)  "<VAPM_ESCStandstillTimeOut_flg>"
  bus_selector2/143 -> outpmodule/158(VAPM_IVIStatusTimeOut_flg)  "<VAPM_IVIStatusTimeOut_flg>"
  bus_selector15/18 -> outpmodule/666(VTPM_LRWheelDebug_flg)  "<VTPM_LRWheelDebug_flg>"
  bus_selector2/122 -> outpmodule/137(VAPM_ESCStandstill_flg)  "<VAPM_ESCStandstill_flg>"
  bus_selector4/96 -> outpmodule/342(VDDM_ISAMalfuncDetDTC_raw32)  "<VDDM_ISAMalfuncDetDTC_raw32>"
  bus_selector2/120 -> outpmodule/135(VAPM_BrkSwV_flg)  "<VAPM_BrkSwV_flg>"
  bus_selector2/119 -> outpmodule/134(VAPM_BrkSwStaTimeOut_flg)  "<VAPM_BrkSwStaTimeOut_flg>"
  bus_selector19/62 -> outpmodule/903(VVMC_LKAHODDisplayWarning_flg)  "<VVMC_LKAHODDisplayWarning_flg>"
  outpmodule/450(VOUTP_AvgBattTempPSAR_C) -> bus_creator/450
  bus_selector2/117 -> outpmodule/132(VAPM_MCPressureVTimeOut_flg)  "<VAPM_MCPressureVTimeOut_flg>"
  outpmodule/527(VOUTP_SysNMmSta_enum) -> bus_creator/527
  bus_selector15/26 -> outpmodule/674(VTPM_RRPressIndi_enum)  "<VTPM_RRPressIndi_enum>"
  bus_selector4/41 -> outpmodule/287(VDDM_FLDoorSWDTC_raw32)  "<VDDM_FLDoorSWDTC_raw32>"
  bus_selector13/37 -> outpmodule/641(VSYS_ECUGen1_cnt)  "<VSYS_ECUGen1_cnt>"
  bus_selector2/118 -> outpmodule/133(VAPM_BrkSwSta_flg)  "<VAPM_BrkSwSta_flg>"
  outpmodule/426(VOUTP_CPSAR_sec) -> bus_creator/426
  bus_selector2/153 -> outpmodule/168(VAPM_DriverSeatBeltCmdTimeOut_flg)  "<VAPM_DriverSeatBeltCmdTimeOut_flg>"
  bus_selector2/116 -> outpmodule/131(VAPM_MCPressureV_bar)  "<VAPM_MCPressureV_bar>"
  outpmodule/841(VOUTP_HVPO120VGrpBLDSt_enum) -> bus_creator/841
  bus_selector2/114 -> outpmodule/129(VAPM_LongAccelV_flg)  "<VAPM_LongAccelV_flg>"
  outpmodule/39(VOUTP_PASAFML_enum) -> bus_creator/39
  bus_selector2/111 -> outpmodule/126(VAPM_YawRateVTimeOut_flg)  "<VAPM_YawRateVTimeOut_flg>"
  outpmodule/230(VOUTP_FDCBCMMRoomLpCmd_pct) -> bus_creator/230
  bus_selector3/55 -> outpmodule/245(VBCM_WakeUp_flg)  "<VBCM_WakeUp_flg>"
  bus_selector19/29 -> outpmodule/870(VVMC_LKAStrToqReq_Nm)  "<VVMC_LKAStrToqReq_Nm>"
  outpmodule/122(VOUTP_LongAccelTimeOut_flg) -> bus_creator/122
  bus_selector2/110 -> outpmodule/125(VAPM_YawRateV_flg)  "<VAPM_YawRateV_flg>"
  bus_selector4/60 -> outpmodule/306(VDDM_DiagFLTSDTC_raw32)  "<VDDM_DiagFLTSDTC_raw32>"
  bus_selector2/109 -> outpmodule/124(VAPM_MCPressureTimeOut_flg)  "<VAPM_MCPressureTimeOut_flg>"
  outpmodule/256(VOUTP_C3CCU2RCDTC_raw32) -> bus_creator/256
  outpmodule/421(VOUTP_HVBattCurr_Ahps) -> bus_creator/421
  bus_selector6/85 -> outpmodule/486(VDID_OFFL_sec)  "<VDID_OFFL_sec>"
  bus_selector2/130 -> outpmodule/145(VAPM_EPBErrSta_enum)  "<VAPM_EPBErrSta_enum>"
  bus_selector3/44 -> outpmodule/234(VBCM_FDCBCMOSDrOpenSWSta_enum)  "<VBCM_FDCBCMOSDrOpenSWSta_enum>"
  outpmodule/872(VOUTP_LKATOIAct_enum) -> bus_creator/872
  bus_selector19/47 -> outpmodule/888(VVMC_ADASShftPosnReq_enum)  "<VVMC_ADASShftPosnReq_enum>"
  bus_selector10/58 -> outpmodule/586(VPMM_DCCurr_A)  "<VPMM_DCCurr_A>"
  bus_selector2/108 -> outpmodule/123(VAPM_MCPressure_bar)  "<VAPM_MCPressure_bar>"
  bus_selector2/107 -> outpmodule/122(VAPM_LongAccelTimeOut_flg)  "<VAPM_LongAccelTimeOut_flg>"
  bus_selector19/15 -> outpmodule/856(VVMC_SingleWhlSlipRatioCtrl_flg)  "<VVMC_SingleWhlSlipRatioCtrl_flg>"
  bus_selector10/54 -> outpmodule/582(VPMM_VSPReversed_flg)  "<VPMM_VSPReversed_flg>"
  bus_selector6/83 -> outpmodule/484(VDID_OVCL_sec)  "<VDID_OVCL_sec>"
  bus_selector2/106 -> outpmodule/121(VAPM_LongAccel_Gps)  "<VAPM_LongAccel_Gps>"
  bus_selector4/56 -> outpmodule/302(VDDM_ESC1NoComDTC_raw32)  "<VDDM_ESC1NoComDTC_raw32>"
  bus_selector2/104 -> outpmodule/119(VAPM_LatAccel_Gps)  "<VAPM_LatAccel_Gps>"
  bus_selector1/5 -> outpmodule/5(VACC_EHPSEnDemand_enum)  "<VACC_EHPSEnDemand_enum>"
  bus_selector16/79 -> outpmodule/824(VTQD_VCUMCUGearSta_enum)  "<VTQD_VCUMCUGearSta_enum>"
  bus_selector1/2 -> outpmodule/2(VACC_CACTempOverHigh_flg)  "<VACC_CACTempOverHigh_flg>"
  bus_selector10/38 -> outpmodule/566(VPMM_V2BOilPosRlySta_enum)  "<VPMM_V2BOilPosRlySta_enum>"
  bus_selector13/8 -> outpmodule/612(VSYS_ECU2_cnt)  "<VSYS_ECU2_cnt>"
  outpmodule/828(VOUTP_EMRC1DrvDemEMRtapTrq_pct) -> bus_creator/828
  outpmodule/32(VOUTP_APSDFLL_cm) -> bus_creator/32
  bus_selector1/3 -> outpmodule/3(VACC_CACPresWarn_flg)  "<VACC_CACPresWarn_flg>"
  bus_selector16/38 -> outpmodule/783(VTQD_EC1EMSpdIdleP1_rpm)  "<VTQD_EC1EMSpdIdleP1_rpm>"
  bus_selector3/11 -> outpmodule/201(VBCM_FDCBCMLTurnLpCmd_flg)  "<VBCM_FDCBCMLTurnLpCmd_flg>"
  bus_selector12/1 -> outpmodule/590(VSCP_triggerBAM_flg)  "<VSCP_triggerBAM_flg>"
  bus_selector1/1 -> outpmodule/1(VACC_EACEnDemand_enum)  "<VACC_EACEnDemand_enum>"
  outpmodule/614(VOUTP_Major2_cnt) -> bus_creator/614
  bus_selector2/25 -> outpmodule/40(VAPM_PASAFCR_enum)  "<VAPM_PASAFCR_enum>"
  outpmodule/284(VOUTP_LVSupLoDTC_raw32) -> bus_creator/284
  outpmodule/354(VOUTP_ESC5CSErrDTC_raw32) -> bus_creator/354
  bus_selector2/1 -> outpmodule/16(VAPM_VehSpeed_kph)  "<VAPM_VehSpeed_kph>"
  bus_selector2/43 -> outpmodule/58(VAPM_BrkPedalPosTimeOut_flg)  "<VAPM_BrkPedalPosTimeOut_flg>"
  bus_selector6/37 -> outpmodule/438(VDID_TGEOVCL_kWh)  "<VDID_TGEOVCL_kWh>"
  bus_selector10/32 -> outpmodule/560(VPMM_V2BMainPosRlySta_enum)  "<VPMM_V2BMainPosRlySta_enum>"
  bus_selector3/14 -> outpmodule/204(VBCM_FDCBCMSTOPBALLCmd_flg)  "<VBCM_FDCBCMSTOPBALLCmd_flg>"
  bus_selector19/91 -> outpmodule/932(VVMC_APSCtrlAvail_flg)  "<VVMC_APSCtrlAvail_flg>"
  bus_selector2/10 -> outpmodule/25(VAPM_PASDFMR_cm)  "<VAPM_PASDFMR_cm>"
  bus_selector19/9 -> outpmodule/850(VVMC_FeatArbitrSta_enum)  "<VVMC_FeatArbitrSta_enum>"
  outpmodule/738(VOUTP_FlashS4ID_raw) -> bus_creator/738
  bus_selector19/63 -> outpmodule/904(VVMC_LKAHODSoundWarning_flg)  "<VVMC_LKAHODSoundWarning_flg>"
  bus_selector13/6 -> outpmodule/610(VSYS_CarModel3_cnt)  "<VSYS_CarModel3_cnt>"
  bus_selector2/9 -> outpmodule/24(VAPM_PASDRCL_cm)  "<VAPM_PASDRCL_cm>"
  bus_selector2/8 -> outpmodule/23(VAPM_PASDRCR_cm)  "<VAPM_PASDRCR_cm>"
  bus_selector4/67 -> outpmodule/313(VDDM_FCRUSSDTC_raw32)  "<VDDM_FCRUSSDTC_raw32>"
  bus_selector2/7 -> outpmodule/22(VAPM_PASDRML_cm)  "<VAPM_PASDRML_cm>"
  bus_selector14/2 -> outpmodule/647(VTHC_CoolFanReq_pct)  "<VTHC_CoolFanReq_pct>"
  bus_selector10/42 -> outpmodule/570(VPMM_V2BAux1RlySta_enum)  "<VPMM_V2BAux1RlySta_enum>"
  outpmodule/674(VOUTP_RRPressIndi_enum) -> bus_creator/674
  bus_selector6/60 -> outpmodule/461(VDID_ETMATOEL_kWh)  "<VDID_ETMATOEL_kWh>"
  bus_selector2/33 -> outpmodule/48(VAPM_USSStaFML_flg)  "<VAPM_USSStaFML_flg>"
  bus_selector4/75 -> outpmodule/321(VDDM_RLRUSSDTC_raw32)  "<VDDM_RLRUSSDTC_raw32>"
  bus_selector2/29 -> outpmodule/44(VAPM_USSStaRLL_flg)  "<VAPM_USSStaRLL_flg>"
  bus_selector13/3 -> outpmodule/607(VSYS_HWVer3_cnt)  "<VSYS_HWVer3_cnt>"
  bus_selector2/165 -> outpmodule/180(VAPM_PUIDLowPower_flg)  "<VAPM_PUIDLowPower_flg>"
  outpmodule/237(VOUTP_FDCBCMFDCloseSVCmd_flg) -> bus_creator/237
  outpmodule/717(VOUTP_TPMSResButt_flg) -> bus_creator/717
  bus_selector2/3 -> outpmodule/18(VAPM_FSOffSw_enum)  "<VAPM_FSOffSw_enum>"
  bus_selector15/72 -> outpmodule/720(VTPM_LRPindi_enum)  "<VTPM_LRPindi_enum>"
  outpmodule/395(VOUTP_VCUTailgateSWSta_flg) -> bus_creator/395
  outpmodule/752(VOUTP_VCUEBSHHSw_enum) -> bus_creator/752
  bus_selector2/147 -> outpmodule/162(VAPM_IVIScreenTimeOut_flg)  "<VAPM_IVIScreenTimeOut_flg>"
  bus_selector2/5 -> outpmodule/20(VAPM_ChrgPlugSta_enum)  "<VAPM_ChrgPlugSta_enum>"
  bus_selector2/2 -> outpmodule/17(VAPM_VehSpeedTimeOut_flg)  "<VAPM_VehSpeedTimeOut_flg>"
  bus_selector2/13 -> outpmodule/28(VAPM_PASDFCL_cm)  "<VAPM_PASDFCL_cm>"
  bus_selector19/4 -> outpmodule/845(VVMC_MeterIndSpeed_raw32)  "<VVMC_MeterIndSpeed_raw32>"
  bus_selector19/5 -> outpmodule/846(VVMC_VMCAEBCtrlAvail_flg)  "<VVMC_VMCAEBCtrlAvail_flg>"
  bus_selector2/12 -> outpmodule/27(VAPM_PASDFCR_cm)  "<VAPM_PASDFCR_cm>"
  bus_selector2/48 -> outpmodule/63(VAPM_LRRawWhlSpeed_kph)  "<VAPM_LRRawWhlSpeed_kph>"
  outpmodule/76(VOUTP_LFWhlRotDirTimeOut_flg) -> bus_creator/76
  bus_selector2/11 -> outpmodule/26(VAPM_PASDFML_cm)  "<VAPM_PASDFML_cm>"
  bus_selector2/15 -> outpmodule/30(VAPM_APSDRLL_cm)  "<VAPM_APSDRLL_cm>"
  bus_selector4/80 -> outpmodule/326(VDDM_FCM3RCErrDTC_raw32)  "<VDDM_FCM3RCErrDTC_raw32>"
  bus_selector2/27 -> outpmodule/42(VAPM_USSStaRML_flg)  "<VAPM_USSStaRML_flg>"
  bus_selector6/71 -> outpmodule/472(VDID_AVGBATTEMPL_C)  "<VDID_AVGBATTEMPL_C>"
  outpmodule/737(VOUTP_FlashS3ID_raw) -> bus_creator/737
  bus_selector2/32 -> outpmodule/47(VAPM_USSStaFMR_flg)  "<VAPM_USSStaFMR_flg>"
  outpmodule/205(VOUTP_FDCBCMInnerCallBellCmd_flg) -> bus_creator/205
  bus_selector10/34 -> outpmodule/562(VPMM_V2BACPosRlySta_enum)  "<VPMM_V2BACPosRlySta_enum>"
  bus_selector2/19 -> outpmodule/34(VAPM_PASARMR_enum)  "<VAPM_PASARMR_enum>"
  bus_selector2/131 -> outpmodule/146(VAPM_EPBErrStaTimeOut_flg)  "<VAPM_EPBErrStaTimeOut_flg>"
  outpmodule/758(VOUTP_GearFlashInd_flg) -> bus_creator/758
  bus_selector16/20 -> outpmodule/765(VTQD_EVCU1ActDrvMode_enum)  "<VTQD_EVCU1ActDrvMode_enum>"
  bus_selector6/84 -> outpmodule/485(VDID_OFFR_sec)  "<VDID_OFFR_sec>"
  bus_selector2/42 -> outpmodule/57(VAPM_BrkPedalPos_pct)  "<VAPM_BrkPedalPos_pct>"
  bus_selector4/84 -> outpmodule/330(VDDM_FCM5NoComDTC_raw32)  "<VDDM_FCM5NoComDTC_raw32>"
  bus_selector13/20 -> outpmodule/624(VSYS_Change2_cnt)  "<VSYS_Change2_cnt>"
  outpmodule/645(VOUTP_ModelYear_cnt) -> bus_creator/645
  bus_selector16/86 -> outpmodule/831(VTQD_VCUMCUHandBrk_flg)  "<VTQD_VCUMCUHandBrk_flg>"
  bus_selector2/18 -> outpmodule/33(VAPM_PASAFCL_enum)  "<VAPM_PASAFCL_enum>"
  outpmodule/174(VOUTP_APSAngleTarget_Deg) -> bus_creator/174
  outpmodule/392(VOUTP_VCURRDoorSta_flg) -> bus_creator/392
  bus_selector19/39 -> outpmodule/880(VVMC_ACCObjRelSpd_mps)  "<VVMC_ACCObjRelSpd_mps>"
  bus_selector2/16 -> outpmodule/31(VAPM_APSDFLR_cm)  "<VAPM_APSDFLR_cm>"
  bus_selector15/85 -> outpmodule/733(VTPM_unlearnSfailvalid_enum)  "<VTPM_unlearnSfailvalid_enum>"
  bus_selector1/14 -> outpmodule/14(VACC_EACSpdDemand_rpm)  "<VACC_EACSpdDemand_rpm>"
  bus_selector1/13 -> outpmodule/13(VACC_EHPSSpdCtrlMode_enum)  "<VACC_EHPSSpdCtrlMode_enum>"
  outpmodule/673(VOUTP_LRPressIndi_enum) -> bus_creator/673
  bus_selector16/37 -> outpmodule/782(VTQD_EMRC1ActMaxAvaEMRecpTrq_pct)  "<VTQD_EMRC1ActMaxAvaEMRecpTrq_pct>"
  bus_selector10/5 -> outpmodule/533(VPMM_PowerUpFault_enum)  "<VPMM_PowerUpFault_enum>"
  bus_selector4/116 -> outpmodule/362(VDDM_RFPressIndiDTC_raw32)  "<VDDM_RFPressIndiDTC_raw32>"
  bus_selector1/11 -> outpmodule/11(VACC_EHPSDisEnTimeout_flg)  "<VACC_EHPSDisEnTimeout_flg>"
  bus_selector19/2 -> outpmodule/843(VVMC_VehicleSpeed_mph)  "<VVMC_VehicleSpeed_mph>"
  bus_selector1/10 -> outpmodule/10(VACC_EHPSEnTimeout_flg)  "<VACC_EHPSEnTimeout_flg>"
  outpmodule/148(VOUTP_EPBStaTimeOut_flg) -> bus_creator/148
  outpmodule/499(VOUTP_DkeyShowIVISta_enum) -> bus_creator/499
  bus_selector4/59 -> outpmodule/305(VDDM_DiagHCrashDTC_raw32)  "<VDDM_DiagHCrashDTC_raw32>"
  outpmodule/768(VOUTP_EVCU1EMotorOvrerSpd_enum) -> bus_creator/768
  bus_selector1/9 -> outpmodule/9(VACC_EHPSSpdDemTimeout_flg)  "<VACC_EHPSSpdDemTimeout_flg>"
  bus_selector1/12 -> outpmodule/12(VACC_DCDCEnDemamd_enum)  "<VACC_DCDCEnDemamd_enum>"
  bus_selector13/40 -> outpmodule/644(VSYS_DrivingMode_cnt)  "<VSYS_DrivingMode_cnt>"
  bus_selector2/17 -> outpmodule/32(VAPM_APSDFLL_cm)  "<VAPM_APSDFLL_cm>"
  outpmodule/558(VOUTP_V2BAux2OnOff_enum) -> bus_creator/558
  bus_selector16/75 -> outpmodule/820(VTQD_RC1RetSpdPekTrqP5_Nm)  "<VTQD_RC1RetSpdPekTrqP5_Nm>"
  bus_selector2/136 -> outpmodule/151(VAPM_AVMparkingexcute_enum)  "<VAPM_AVMparkingexcute_enum>"
  outpmodule/926(VOUTP_FCMLDWFault_flg) -> bus_creator/926
  bus_selector1/7 -> outpmodule/7(VACC_CACRunFail_flg)  "<VACC_CACRunFail_flg>"
  outpmodule/478(VOUTP_ECUNAME_cnt) -> bus_creator/478
  bus_selector3/24 -> outpmodule/214(VBCM_FDCBCMFDoorSta_flg)  "<VBCM_FDCBCMFDoorSta_flg>"
  bus_selector2/38 -> outpmodule/53(VAPM_Chime_enum)  "<VAPM_Chime_enum>"
  bus_selector2/35 -> outpmodule/50(VAPM_USSStaFLL_flg)  "<VAPM_USSStaFLL_flg>"
  outpmodule/777(VOUTP_RC1PctTrqPekTrqP5_pct) -> bus_creator/777
  bus_selector2/30 -> outpmodule/45(VAPM_USSStaRCR_flg)  "<VAPM_USSStaRCR_flg>"
